simulink model "SAME5x_EXpicGUI_base"  (R2020b)
settings: Solver=FixedStepDiscrete  StartTime=0.0  StopTime=10.0  FixedStep=Ts  RelTol=1e-3  EnableMultiTasking=on
InitFcn:
  | % DC Voltage
  | VDC = 24;
  | 
  | 
  | % Intersective PMW
  | Vmax = VDC/2;
  | Imax = 4;
  | 
  | Ts = 1e-4;
  | 
  | 
  | 
  | 
  | 
  | 
  | % pole paires
  | p = 4;
  | 
  | % QEI
  | lines = 4*1000;
  | eleclines = lines/p;
  | inveleclines = 1/eleclines
  | gainQEIspeed = 2*pi/Ts/lines
  | 
  | 
  | 
  | % Electrical parameters
  | R=0.656; L=0.35e-3; Phif=0.0066;
  | % Mechanical parameters
  | F=1.e-05; J=1e-05; C0 = 0.01;%10;%1;
  | 
  | %% Current control synthesis
  | % Desired Carateristc Equation
  | %  1         2zeta
  | % ---- p^2+ ------- p + 1
  | % wn^2        wn
  | % Overshoot 5%, Trbf x wnbf = 3
  | tauE = L/R;
  | kE = 1/R;
  | trE = 3*tauE;
  | trED = trE;
  | zetaED = 1;
  | trwnE = 5;
  | wnED = trwnE/trED;
  | Pole_elec_desiree = roots([1/wnED^2 2*zetaED/wnED 1]);
  | 
  | % Retour d'etat de la dynamique electrique
  | Ae = [
  |         -R/L 0;
  |         -1 0;
  |     ];
  | 
  | Be = [
  |         1/L;
  |         0;
  |     ];
  | 
  | Kelec = place(Ae,Be,Pole_elec_desiree)
  | Kelec2 = [(2*zetaED*wnED*tauE-1)/kE -tauE*wnED^2/kE]
  | 
  | %% Asservissement de vitesse
  | % Desired polynomial equation
  | %  1         2 zeta
  | % ---- p^2+ ------- p + 1
  | % wn^2        wn
  | % overshoot 5%, Trbf x wnbf = 3
  | tauM = J/F;
  | kM = 3/2*p*Phif/F;
  | trM = 3*tauM;
  | zetaMD = 0.7;
  | trMD = trM/10;
  | trwnM = 3;
  | wnMD = trwnM/trMD;
  | Desired_mecha_pole = roots([1/wnMD^2 2*zetaMD/wnMD 1]);
  | % Mechanical state feedback
  | Am = [
  |         -1/tauM 0;
  |         -1 0;
  |     ];
  | 
  | Bm = [
  |         kM/tauM;
  |         0;
  |     ];
  | 
  | 
  | Kmeca = place(Am,Bm,Desired_mecha_pole)
  | 
  | Kmeca2 = [(2*zetaMD*wnMD*tauM-1)/kM -tauM*wnMD^2/kM]
  | 
  | 
  | 
  | 
  | 
  | 
  | % pole paires
  | pinit = 5;
  | % Electrical parameters
  | Rinit=0; Linit=0; Phifinit=0;
  | % Mechanical parameters
  | finit=1.0441e-04; Jinit=1.908e-04;
  | 
  | 
  | linesinit = 250;
  | 
  | %% Control law
  | %% Current control synthesis
  | 
  | Gainelecinit = 3;
  | Gainmecainit = .1;
undefined symbols (not defined in the file or in its folder): DiscIntNeverNeededParam, gcbh, MCHP_Digital_Input_Callback, MCHP_Digital_Output_Write_Callback, MCHP_Master_Callback, MCHP_OrderInOut, myParam, PA10, PA11, PA12, PA13, pad0, pad1, pad2, pad3, Pin
libraries: simulink x13, MCHP_Blockset x5
(part 1 of 3)
Description:
  | Motor Control Demo SAME5x
  | contacts : romain.delpoux@insa-lyon.fr, lubin.kerhuel@microchip.com
settings Model: Creator=r.delpoux  LastModifiedBy=promu
settings OptimizationCC: DefaultParameterBehavior=Inlined  DefaultUnderspecifiedDataType=single  EnhancedBackFolding=on  BooleansAsBitfields=on  PassReuseOutputArgsAs=Individual arguments  ZeroExternalMemoryAtStartup=off  ZeroInternalMemoryAtStartup=off  OptimizeBlockOrder=speed  DifferentSizesBufferReuse=on  EfficientTunableParamExpr=on
settings DebuggingCC: MultiTaskDSMMsg=none  MultiTaskCondExecSysMsg=warning  ParameterTunabilityLossMsg=error
settings HardwareCC: ProdBitPerPointer=32  ProdBitPerSizeT=32  ProdBitPerPtrDiffT=32  ProdLargestAtomicInteger=Long  ProdLargestAtomicFloat=Double  ProdWordSize=32  ProdHWDeviceType=ARM Compatible->ARM Cortex
settings ModelReferenceCC: ModelReferenceNumInstancesAllowed=Single
settings SFSimCC: MATLABDynamicMemAlloc=off
settings RTWCC: Description=Microchip Embedded Target Cortex M7 (real-time)  SystemTargetFile=MCHP_ARM7_stf.tlc  TemplateMakefile=MCHP_ARM7.tmf  Toolchain=xc32 - v2.50 for Mirochip SAMx7 device  BuildConfiguration=Specify
settings CodeAppCC: ForceParamTrailComments=on  IgnoreCustomStorageClasses=off  MaxIdLength=255  OperatorAnnotations=on  SimulinkDataObjDesc=on  SFDataObjDesc=on  InsertBlockDesc=on
settings STFCustomTargetCC: MultiwordLength=256  ConcurrentExecutionCompliant=off  IncludeMdlTerminateFcn=off  CombineOutputUpdateFcns=on  CombineSignalStateStructs=on  SuppressErrorStatus=on  ERTCustomFileBanners=on  SupportContinuousTime=off  RemoveResetFunc=on  MATLABClassNameForMDSCustomization=Simulink.SoftwareTarget.ERTCustomization  CPPClassGenCompliant=off  GRTInterface=off  UseToolchainInfoCompliant=on  SystemTargetFile=MCHP_ARM7_stf.tlc
settings ERTTargetCC: ParMdlRefBuildCompliant=off  CompOptLevelCompliant=off  ConcurrentExecutionCompliant=off  IncludeMdlTerminateFcn=off  CombineSignalStateStructs=on  SuppressErrorStatus=on  SupportNonInlinedSFcns=on  ModelStepFunctionPrototypeControlCompliant=off  CPPClassGenCompliant=off  ExtModeStaticAllocSize=2000  InlinedParameterPlacement=NonHierarchical  ERTSrcFileBannerTemplate=MCHP_dsPIC_code_template.cgt  ERTHdrFileBannerTemplate=MCHP_dsPIC_code_template.cgt  ERTDataSrcFileTemplate=MCHP_dsPIC_code_template.cgt  ERTDataHdrFileTemplate=MCHP_dsPIC_code_template.cgt  ERTCustomFileTemplate=MCHP_main.tlc  MaxLineWidth=110

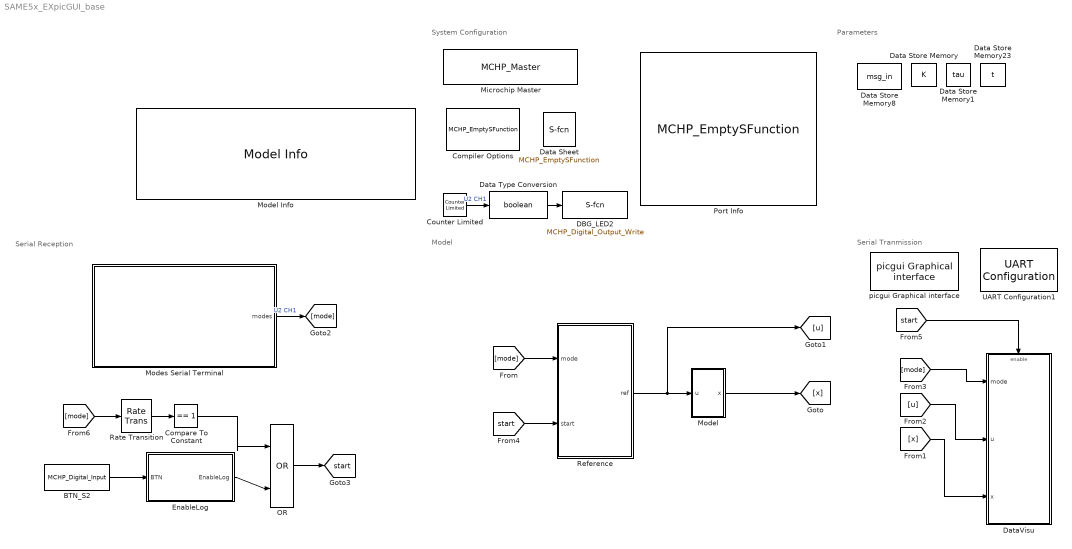
== system SAME5x_EXpicGUI_base ==
  note: Serial Reception
  note: System Configuration
  note: Serial Tranmission
  note: Model
  note: Parameters
  BTN_S2 : S-Function  FunctionName=MCHP_Digital_Input  Parameters=SampleTime,[],MCHP_Digital_Input_Callback(gcb,'S_OUTPUT'),MCHP_OrderInOut(gcbh)  SFunctionDeploymentMode=off  EnableBusSupport=off  mask(Input driver for Digital Input Pins){PORT=Dynamic Options, PORT_TXT=D   [ 0  1  8  9  10  11  12  20  21 ], PIN=9, PACK=off, SIMULTANEOUS=off, ORDERING=None, SampleTime=.1, MCHP_PORT={Digital In}{DIN}2:0:D9;, MCHP_MASTERLINK=SAME5x_EXpicGUI/Microchip Master}
      mask prompts: PORT_TXT "Port TXT"; PIN "PORT D Indexes within [ 0  1  8  9  10  11  12  20  21 ]"; PACK "set block output as one uint32"; SIMULTANEOUS "Exact simultaneous sample"; ORDERING "Block execution ordering"; SampleTime "Sample Time"
      mask help:
      | Selected pin(s) are configured as a digital input.
      |
      | When the block output is defined as one uint16, user should
      | take into account only bits corresponding to pins selected.
      mask init:
      | MCHP_Digital_Input_Callback(gcb,'INITIALISATION');
      settings: PreSaveFcn=MCHP_Fun.PreSaveFcn_DynamicOptions(gcbh);  OpenFcn=MCHP_Digital_Input_Callback(gcb,'OPEN');
      mask TypeOptions PORT: Dynamic Options
      mask Callback PORT: MCHP_Fun.BlockUpdate(gcbh);
      mask Callback PIN: MCHP_Fun.BlockUpdate(gcbh);
      mask Callback PACK: MCHP_Fun.BlockUpdate(gcbh);
      mask Callback SIMULTANEOUS: %MCHP_Fun.BlockUpdate(gcbh);
      mask TypeOptions ORDERING: None | Input | Output | Input & Output
      mask Display:
      | MCHP_DrawLogo;fprintf('Digital\nInput')
      | port_label('output',1,'D9');
  Compare To Constant : simulink/Logic and Bit Operations/Compare To Constant  relop===  const=1  OutDataTypeStr=boolean
  Compiler Options : S-Function  Priority=1  FunctionName=MCHP_EmptySFunction  SFunctionDeploymentMode=off  EnableBusSupport=off  mask{LATEST_CMPLR=on, COMP_LIST=Dynamic Options, COMP_LIST_TXT=xc32 - v2.50, DFP_LIST=Dynamic Options, DFP_LIST_TXT=v 3.2.56, CMSIS_DSP=Dynamic Options, CMSIS_DSP_TXT=Not used, USE_64BIT_DOUBLE=off, MCHP_MULTITHREAD_COMPILATION=on, UseCustom_LinkerScript=off, LinkerScript=, MCHP_MASTERLINK=SAME5x_EXpicGUI/Microchip Master, OPTIMIZATION_LEVEL=3, OPTIMIZATION_FLTO=off, OPTIMIZATION_REORDER=off, UNROLL_LOOPS=off, PROCEDURAL_ABSTRACTION=off, MPLAB_LINKLIB=default, MPLAB_LINKLIB1=fast floating-point math, CUSTOM_OPTIM=, CUSTOM_OPTIM_LD=, MCODE=is less than 32768 (faster), MCONST=in data memory, MDATA=Use only memory below address 8192 (faster), MSCALAR=Use only memory below address 8192 (faster), MLARGEARRAY=off, MAGGREGATE=off, HEAP_SIZE=1024, OMF=elf, DEBUG_INFO=on, ProduceHexOutput=on, AssemblyListing=off, NO_EDS_WARN=on, PRINT_STATISTICS=off}
      mask prompts: LATEST_CMPLR "Always use the latest compiler"; COMP_LIST "Select Compiler"; DFP_LIST "Device Family Pack (DFP)"; CMSIS_DSP "CMSIS DSP library"; USE_64BIT_DOUBLE "Use 64-bit double"; MCHP_MULTITHREAD_COMPILATION "Multithread Compilation (faster build)"; UseCustom_LinkerScript "Use a Custom Linker Script"; LinkerScript "Linker Script filename (full path if not in the model folder)"; OPTIMIZATION_LEVEL "Optimisation Level"; OPTIMIZATION_FLTO "Enable link-time optimizer"; OPTIMIZATION_REORDER "Allow reordering for ( fcts - variable - asm )"; UNROLL_LOOPS "Unroll Loops (improve speed)"; PROCEDURAL_ABSTRACTION "Procedural abstraction (reduce size)"; MPLAB_LINKLIB "Math Library"; MPLAB_LINKLIB1 "Math Library"; CUSTOM_OPTIM "Add custom argument for compiler"; CUSTOM_OPTIM_LD "Add custom argument for linker (coma separated)"; MCODE "Code size"; MCONST "Store Constant"; MDATA "Table data"; MSCALAR "Scalar data"; MLARGEARRAY "Allow array larger than 32K"; MAGGREGATE "Use aggregate data model"; HEAP_SIZE "Heap size"; OMF "Binary format :"; DEBUG_INFO "Generate debugging information"; ProduceHexOutput "Produce hex binary output file (.hex)"; AssemblyListing "Produce assembly listing file (.lst)"; NO_EDS_WARN "Disable eds-warning"; PRINT_STATISTICS "Print some statistics"
      mask init:
      | MCHP_CompilerOptimisation_Callback(gcbh, 'INITIALISATION');
      settings: PreSaveFcn=MCHP_Fun.PreSaveFcn_DynamicOptions(gcbh);  OpenFcn=MCHP_CompilerOptimisation_Callback(gcbh, 'OPEN');
      mask Callback LATEST_CMPLR: MCHP_Fun.BlockUpdate(gcbh);
      mask TypeOptions COMP_LIST: Dynamic Options
      mask Callback COMP_LIST: MCHP_Fun.BlockUpdate(gcbh);
      mask TypeOptions DFP_LIST: Dynamic Options
      mask TypeOptions CMSIS_DSP: Dynamic Options
      mask Callback UseCustom_LinkerScript: MCHP_CompilerOptimisation_Callback(gcbh, 'UseCustom_LinkerScript');
      mask TypeOptions OPTIMIZATION_LEVEL: 0 | 1 | 2 | s | 3
      mask TypeOptions MPLAB_LINKLIB: default | fast floating-point math | relaxed floating-point math
      mask TypeOptions MPLAB_LINKLIB1: default | fast floating-point math
      mask TypeOptions MCODE: is less than 32768 (faster) | is more than 32768
      mask TypeOptions MCONST: in code memory | in data memory
      mask TypeOptions MDATA: Use only memory below address 8192 (faster) | Can use all available memory
      mask TypeOptions MSCALAR: Use only memory below address 8192 (faster) | Can use all available memory
      mask TypeOptions OMF: elf | coff
      mask DialogControl ParameterTabVar0 Prompt: Compiler
      mask DialogControl ParameterTabVar01 Prompt: Optimization
      mask DialogControl ParameterTabVar012 Prompt: Memory
      mask DialogControl ParameterTabVar0123 Prompt: Output
      mask DialogControl ParameterTabVar01234 Prompt: Messages
      mask Display: MCHP_DrawLogo;disp(['Compiler-Version\n' COMP_LIST_TXT]);
  Counter Limited : simulink/Sources/Counter Limited  uplimit=1  tsamp=.1
  DBG_LED2 : S-Function  FunctionName=MCHP_Digital_Output_Write  Parameters=SampleTime,MCHP_Digital_Output_Write_Callback(gcb,'S_INPUT'),MCHP_Digital_Output_Write_Callback(gcb,'S_OUTPUT'),MCHP_OrderInOut(gcbh)  SFunctionDeploymentMode=off  EnableBusSupport=off  mask(Output driver for Digital Output Pins){PORT=Dynamic Options, PORT_TXT=B   [ 0 : 31 ], PIN=26, PACK=off, SIMULTANEOUS=off, ORDERING=None, SampleTime=-1, MCHP_PORT={Digital Out}{DOU}1:1:B26;, MCHP_MASTERLINK=SAME5x_EXpicGUI/Microchip Master}
      mask prompts: PORT_TXT "Port TXT"; PIN "PORT D Indexes within [ 0  1  8  9  10  11  12  20  21 ]"; PACK "set input as one uint16"; SIMULTANEOUS "Exact simultaneous update"; ORDERING "Block execution ordering"; SampleTime "Sample Time"
      mask help:
      | Selected pin(s) are configured as a digital output.
      |
      | When the block input is defined as one uint16, the value
      | is beeing used as is without masks.
      | This behaviour might affect others pins from the same port
      | provided they are configured as digital output as well.
      mask init:
      | MCHP_Digital_Output_Write_Callback(gcb,'INITIALISATION');
      settings: PreSaveFcn=MCHP_Fun.PreSaveFcn_DynamicOptions(gcbh);  OpenFcn=MCHP_Digital_Output_Write_Callback(gcb,'OPEN');
      mask TypeOptions PORT: Dynamic Options
      mask Callback PORT: MCHP_Fun.BlockUpdate(gcbh);
      mask Callback PIN: MCHP_Fun.BlockUpdate(gcbh);
      mask Callback PACK: MCHP_Fun.BlockUpdate(gcbh);
      mask Callback SIMULTANEOUS: %MCHP_Digital_Output_Write_Callback(gcb,'SIMULTANEOUS');
      mask TypeOptions ORDERING: None | Input | Output | Input & Output
      mask Display:
      | MCHP_DrawLogo;fprintf('Digital\nOutput\nWrite')
      | port_label('input',1,'B26');
  Data Sheet : S-Function  FunctionName=MCHP_EmptySFunction  SFunctionDeploymentMode=off  EnableBusSupport=off  mask{DOC_Type=datasheet, DOC_MCHP_Id=SAME54P20A_datasheet, DOC_FilePath=C:\Users\M91449\AppData\Local\Temp\60001507E.pdf, DOC_FileLastCheckTime=[2020              3             11             16              4         38.212], cpy_MCHP_Id=SAME54P20A, MCHP_MASTERLINK=SAME5x_EXpicGUI/Microchip Master}
      mask init:
      | MCHP_Doc_Callback(gcb,'INITIALISATION');
      settings: AttributesFormatString=%<cpy_MCHP_Id>  CopyFcn=MCHP_Doc_Callback(gcb,'COPY');  OpenFcn=MCHP_Doc_Callback(gcb,'OPEN');
      mask TypeOptions DOC_Type: datasheet | errata | www
      mask Display:
      | MCHP_DrawLogo;
      | plot([.8 0 0 1 1 .8 .8 1],[1 1 0 0 .8 1 .8 .8]);
      | text(.5,.6,'DOC','horizontalalignment','center');
      | text(.95,.05,'Pdf','verticalalignment','bottom','horizontalalignment','right');
  Data Store Memory : DataStoreMemory  DataStoreName=K  ReadBeforeWriteMsg=warning  WriteAfterWriteMsg=warning  WriteAfterReadMsg=warning  InitialValue=1  ShowAdditionalParam=off  OutDataTypeStr=single
  Data Store Memory1 : DataStoreMemory  DataStoreName=tau  ReadBeforeWriteMsg=warning  WriteAfterWriteMsg=warning  WriteAfterReadMsg=warning  InitialValue=0.1  ShowAdditionalParam=off  OutDataTypeStr=single
  Data Store Memory23 : DataStoreMemory  DataStoreName=t  ReadBeforeWriteMsg=warning  WriteAfterWriteMsg=warning  WriteAfterReadMsg=warning  InitialValue=1  ShowAdditionalParam=off  OutDataTypeStr=single
  Data Store Memory8 : DataStoreMemory  DataStoreName=msg_in  ReadBeforeWriteMsg=warning  WriteAfterWriteMsg=warning  WriteAfterReadMsg=warning  InitialValue=zeros(1,50)  ShowAdditionalParam=off
  Data Type Conversion : DataTypeConversion  OutDataTypeStr=boolean
  DataVisu : Subsystem
  EnableLog : Subsystem
  Microchip Master : S-Function  Priority=1  InitFcn=MCHP_Master_Callback(gcbh,'INIT');  FunctionName=MCHP_Master  SFunctionDeploymentMode=off  EnableBusSupport=off  mask{PICREF=SAME54P20A - TQFP128, PICREF_spd=, TIMESTEP_REF=Timer  ( 0.001s ), BUSYFLAG=Dynamic Options, BUSYFLAG_TXT=None, PWRTEN=Not used, BOREN=Disable, BODENV=2.7V, BORV=Not used, FPWRT=64ms, DSBOREN=Enable ZPBOR during Deep Sleep Mode, DSLPBOR=Not used, MCLRE=Enabled, SMCLR=MCLR pin generates a normal system Reset, PMDL1WAY=Allow only one reconfiguration, RSTPRI=Device will obtain reset instruction from Primary flash, TEMP=Not used, SOSCSRC=Not used, SOSCSEL=Not used, IOL1WAY=Allow only one reconfiguration, ALTVREF=Not used, DISUVREG=Not used, DSSWEN=Not used, LPCFG=Not used, RTCBAT=Not used, VBTBOR=Not used, WUTSEL=Not used, POWERSAVE=off, FNOSC=Primary Oscillator with PLL module (XT + PLL; HS + PLL; EC + PLL), FPR=ECIO w/ PLL 16x, FOSFPR=HS3 w/PLL 16x, FOS=Internal Fast RC, FRANGE=High Range, OSCILLATOR_SELECT=Crystal Oscillator in 8-48MHz on XIN/XOUT 0, OSCILLATOR_SELECT_spd=Crystal Oscillator in 8-48MHz on XIN/XOUT 0, QUARTZ=12e6, QUARTZ_spd=12e6, POSCGAIN=2x gain setting, POSCBOOST=Boost the kick start of the oscillator, SOSCGAIN=2x gain setting, SOSCBOOST=Boost the kick start of the oscillator, ACTIV_PLL=on, ACTIV_PLL_spd=on, MIPS_DESIRED=100e6, MIPS_DESIRED_spd=100e6, FPLLMUL=Not used, FPLLIDIV=8x Divider, POSCFREQ=Not used, POSCMD=Primary Oscillator Disabled, POSCMOD=Primary osc disabled, MIPS=100 * 1e6, ACLKCON=Optimized for PWM resolution & ADC conversion speed, ACLKCON_spd=Optimized for PWM resolution & ADC conversion speed, ACLKCON_Info=use FRC with auxilliary PLL, ADC Tad = 16.961(ns), PWM max resolution = 1.06(ns), FPLLODIV=32x Divider, PLLKEN=Clock switch to PLL source will wait until the PLL lock signal is valid, FCKSM=Both Clock switching and Fail-safe Clock Monitor are disabled, FCKSMEN=Sw Disabled; Mon Disabled, IESO=Start up with FRC; then switch, DSWDTPS=1:2^36, FWDTEN=Disable, FWDTWINSZ=Window size is 25%, FWPSA=1:512, FWPSA0=1:128, FWPSB=1:16, WDT=Disable, WDTPOST=1:32768, WDTPRE=1:128, WDTPS=1:1048576, WINDIS=Watchdog Timer in Non-Window mode, WWDTEN=Non-Window mode, DSWDTEN=Enable DSWDT during Deep Sleep Mode, DSWDTOSC=Select LPRC as DSWDT Reference clock, FPBDIV=Not used, FSOSCEN=Disable Secondary Oscillator, LPRCSEL=Not used, OSCIOFCN=Not used, OSCIOFNC=OSC2 is clock output, LVRCFG=Not used, PLL_96MHZ=Not used, PLL96MHZ=Not used, PLLDIV=Not used, WDTCLK=Not used, WDTCMX=Not used, WDTWIN=WDT Window is 25% of WDT period, XTCFG=24-32 MHz crystals, XTBST=Boost the kick-start, APL=Aux Flash Code protect is disabled, APLK=Aux Flash Write Protection or Code Protection is Enabled, AWRP=Auxiliary program memory is not write-protected, BSS=No Protection (other than BWRP), BWP=Not used, BWRP=Boot Segment may be written, CP=Protection Disabled, EBS=No Boot EEPROM, ESS=No Segment Data EEPROM, GCP=Disable, GSS=No Protection (other than GWRP), GSS0=Not used, GSSK=General Segment Write Protection or Code Protection is Enabled, GWRP=General Segment may be written, PWP=Not used, RBS=No Boot RAM, RSS=No Secure RAM, SSS=No Secure Segment, SWRP=Secure segment may be written, WPCFG=Not used, WPDIS=Not used, WPEND=Not used, WPFP=Not used, ICESEL=Communicate on PGEC1/PGED1, ICS=Communicate on PGEC1 and PGED1, JTAGEN=Disable, COE=Not used, RES=Not used, DEBUG=Debugger is disabled, BACKBUG=Not used, BKBUG=Not used, ALTI2C=I2C mapped to SDA1/SCL1 pins, ALTI2C1=I2C1 mapped to SDA1/SCL1 pins, ALTI2C2=I2C2 mapped to SDA2/SCL2 pins, ALTI2C3=I2C3 mapped to SDA3/SCL3 pins, ALTQIO=QEA1; QEB1; INDX1 are selected as inputs to QEI1, ALTSS1=SS1A is selected as the I/O pin for SPI1, CMPPOL0=Hysteresis is applied to falling edge, CMPPOL1=Hysteresis is applied to falling edge, FCANIO=Not used, FETHIO=Default Ethernet I/O, FMIIEN=MII Enabled, FSRSSEL=Not used, FUSBIDIO=Controlled by the USB Module, FVBUSONIO=Not used, HPOL=Active High, HYST0=45 mV Hysteresis, HYST1=45 mV Hysteresis, I2C1SEL=Not used, LPOL=Active High, PWMPIN=Control with PORT/TRIS regs, RTCOSC=Not used, UPLLEN=USB PLL Disabled, UPLLIDIV=Not used, ATMOD8=Not used, ALTPMP=Not used, I2C2SEL=Not used, ALTADREF=Not used, ALTCVREF=Not used, PWMLOCK=PWM registers may be written without key sequence, INT_PRIORITY_DMA=0, MCHP_TIMER_REQUEST={Time Step}{TS}0:2:3:1:[]:70000;, MCHP_TIMER_RESULT=[1 8748.999999999992724 ], MCHP_PORT=, MCHP_PLLRegisters=[5    243  16387     -1     -1], MCHPVAR=MCHP.id.name='SAME54P20A';MCHP.id.N=reshape([54 20 -1],1,3);MCHP.id.L=reshape({ 'SAME','P','A'},1,3);MCHP.id.Arch=5;MCHP.id.pinout=reshape({ 'TFBGA120','TQFP128'},1,2);MCHP.Rx=reshape([1 125 3 13 -1 -1 -1 -1 -1 -1 -1 -1 -1 -1 -1 -1 -1 -1 -1 -1 -1 2 126 4 16 -1 -1 -1 -1 -1 -1 -1 -1 -1 -1 -1 -1 -1 -1 -1 -1 -1 9 127 7 -1 -1 -1 -1 -1 -1 -1 -1 -1 -1 -1 -1 -1 -1 -1 -1 -1 -1 10 128 8 -1 -1 -1 -1 -1 -1 -1 -1 -1 -1 -1 -1 -1 -1 -1 -1 -1 -1 21 11 27 -1 -1 -1 -1 -1 -1 -1 -1 -1 -1 -1 -1 -1 -1 -1 -1 -1 -1 22 12 28 -1 -1 -1 -1 -1 -1 -1 -1 -1 -1 -1 -1 -1 -1 -1 -1 -1 -1 23 17 29 -1 -1 -1 -1 -1 -1 -1 -1 -1 -1 -1 -1 -1 -1 -1 -1 -1 -1 24 18 30 -1 -1 -1 -1 -1 -1 -1 -1 -1 -1 -1 -1 -1 -1 -1 -1 -1 -1 33 19 -1 47 -1 -1 -1 -1 -1 -1 -1 -1 -1 -1 -1 -1 -1 -1 -1 -1 -1 34 20 -1 48 -1 -1 -1 -1 -1 -1 -1 -1 -1 -1 -1 -1 -1 -1 -1 -1 -1 35 39 52 49 -1 -1 -1 -1 -1 -1 -1 -1 -1 -1 -1 -1 -1 -1 -1 -1 -1 36 40 55 50 -1 -1 -1 -1 -1 -1 -1 -1 -1 -1 -1 -1 -1 -1 -1 -1 -1 60 41 56 51 -1 -1 -1 -1 -1 -1 -1 -1 -1 -1 -1 -1 -1 -1 -1 -1 -1 61 42 57 -1 -1 -1 -1 -1 -1 -1 -1 -1 -1 -1 -1 -1 -1 -1 -1 -1 -1 62 43 58 -1 -1 -1 -1 -1 -1 -1 -1 -1 -1 -1 -1 -1 -1 -1 -1 -1 -1 63 44 59 -1 -1 -1 -1 -1 -1 -1 -1 -1 -1 -1 -1 -1 -1 -1 -1 -1 -1 66 82 70 -1 -1 -1 -1 -1 -1 -1 -1 -1 -1 -1 -1 -1 -1 -1 -1 -1 -1 67 83 71 -1 -1 -1 -1 -1 -1 -1 -1 -1 -1 -1 -1 -1 -1 -1 -1 -1 -1 68 84 72 -1 -1 -1 -1 -1 -1 -1 -1 -1 -1 -1 -1 -1 -1 -1 -1 -1 -1 69 85 73 -1 -1 -1 -1 -1 -1 -1 -1 -1 -1 -1 -1 -1 -1 -1 -1 -1 -1 88 86 74 80 -1 -1 -1 -1 -1 -1 -1 -1 -1 -1 -1 -1 -1 -1 -1 -1 -1 89 87 75 81 -1 -1 -1 -1 -1 -1 -1 -1 -1 -1 -1 -1 -1 -1 -1 -1 -1 92 98 76 -1 -1 -1 -1 -1 -1 -1 -1 -1 -1 -1 -1 -1 -1 -1 -1 -1 -1 93 99 77 -1 -1 -1 -1 -1 -1 -1 -1 -1 -1 -1 -1 -1 -1 -1 -1 -1 -1 94 100 108 -1 -1 -1 -1 -1 -1 -1 -1 -1 -1 -1 -1 -1 -1 -1 -1 -1 -1 95 101 109 -1 -1 -1 -1 -1 -1 -1 -1 -1 -1 -1 -1 -1 -1 -1 -1 -1 -1 -1 102 110 -1 -1 -1 -1 -1 -1 -1 -1 -1 -1 -1 -1 -1 -1 -1 -1 -1 -1 113 103 111 -1 -1 -1 -1 -1 -1 -1 -1 -1 -1 -1 -1 -1 -1 -1 -1 -1 -1 -1 104 112 -1 -1 -1 -1 -1 -1 -1 -1 -1 -1 -1 -1 -1 -1 -1 -1 -1 -1 -1 105 -1 -1 -1 -1 -1 -1 -1 -1 -1 -1 -1 -1 -1 -1 -1 -1 -1 -1 -1 119 121 123 -1 -1 -1 -1 -1 -1 -1 -1 -1 -1 -1 -1 -1 -1 -1 -1 -1 -1 120 122 124 -1 -1 -1 -1 -1 -1 -1 -1 -1 -1 -1 -1 -1 -1 -1 -1 -1 -1],21,32);MCHP.memory.FLASH.size=1048576;MCHP.memory.SW0.size=16;MCHP.memory.TEMP_LOG.size=512;MCHP.memory.USER_PAGE.size=512;MCHP.memory.CMCC.size=16777216;MCHP.memory.CMCC_DATARAM.size=4096;MCHP.memory.CMCC_TAGRAM.size=1024;MCHP.memory.CMCC_VALIDRAM.size=64;MCHP.memory.QSPI.size=16777216;MCHP.memory.HSRAM.size=262144;MCHP.memory.HSRAM_ETB.size=32768;MCHP.memory.HSRAM_RET1.size=32768;MCHP.memory.HPB0.size=17408;MCHP.memory.HPB1.size=139264;MCHP.memory.HPB2.size=15360;MCHP.memory.HPB3.size=12288;MCHP.memory.SEEPROM.size=131072;MCHP.memory.SDHC0.size=3072;MCHP.memory.SDHC1.size=3072;MCHP.memory.BKUPRAM.size=8192;MCHP.memory.PPB.size=1048576;MCHP.memory.SCS.size=4096;MCHP.memory.PERIPHERALS.size=MCHP_Fun.Hex2num('41C0000000000000');MCHP.module.PM.PID=0;MCHP.module.PM.vector='PM';MCHP.module.MCLK.PID=1;MCHP.module.MCLK.vector='MCLK';MCHP.module.OSCCTRL(1).PID=2;MCHP.module.OSCCTRL(1).vector='OSCCTRL_XOSC0';MCHP.module.OSCCTRL(2).PID=3;MCHP.module.OSCCTRL(2).vector='OSCCTRL_XOSC1';MCHP.module.OSCCTRL(3).PID=4;MCHP.module.OSCCTRL(3).vector='OSCCTRL_DFLL';MCHP.module.OSCCTRL(4).PID=5;MCHP.module.OSCCTRL(4).vector='OSCCTRL_DPLL0';MCHP.module.OSCCTRL(5).PID=6;MCHP.module.OSCCTRL(5).vector='OSCCTRL_DPLL1';MCHP.module.OSC32KCTRL.PID=7;MCHP.module.OSC32KCTRL.vector='OSC32KCTRL';MCHP.module.SUPC(1).PID=8;MCHP.module.SUPC(1).vector='SUPC_OTHER';MCHP.module.SUPC(2).PID=9;MCHP.module.SUPC(2).vector='SUPC_BODDET';MCHP.module.WDT.PID=10;MCHP.module.WDT.vector='WDT';MCHP.module.RTC.PID=11;MCHP.module.RTC.vector='RTC';MCHP.module.EIC(1).PID=12;MCHP.module.EIC(1).vector='EIC_EXTINT_0';MCHP.module.EIC(1).pin.EXTINT0.txt=reshape({ 'PA00','PA16','PB00','PB16','PC00','PC16','PD00'},1,7);MCHP.module.EIC(1).pin.EXTINT0.Rx_idx=reshape([0 16 32 48 64 80 96],1,7);MCHP.module.EIC(1).pin.EXTINT0.ABCD=reshape([0 0 0 0 0 0 0],1,7);MCHP.module.EIC(1).pin.EXTINT1.txt=reshape({ 'PA01','PA17','PB01','PB17','PC01','PC17','PD01'},1,7);MCHP.module.EIC(1).pin.EXTINT1.Rx_idx=reshape([1 17 33 49 65 81 97],1,7);MCHP.module.EIC(1).pin.EXTINT1.ABCD=reshape([0 0 0 0 0 0 0],1,7);MCHP.module.EIC(1).pin.EXTINT2.txt=reshape({ 'PA02','PA18','PB02','PB18','PC02','PC18'},1,6);MCHP.module.EIC(1).pin.EXTINT2.Rx_idx=reshape([2 18 34 50 66 82],1,6);MCHP.module.EIC(1).pin.EXTINT2.ABCD=reshape([0 0 0 0 0 0],1,6);MCHP.module.EIC(1).pin.EXTINT3.txt=reshape({ 'PA03','PA19','PB03','PB19','PC03','PC19','PD08'},1,7);MCHP.module.EIC(1).pin.EXTINT3.Rx_idx=reshape([3 19 35 51 67 83 104],1,7);MCHP.module.EIC(1).pin.EXTINT3.ABCD=reshape([0 0 0 0 0 0 0],1,7);MCHP.module.EIC(1).pin.EXTINT4.txt=reshape({ 'PA04','PA20','PB04','PB20','PC04','PC20','PD09'},1,7);MCHP.module.EIC(1).pin.EXTINT4.Rx_idx=reshape([4 20 36 52 68 84 105],1,7);MCHP.module.EIC(1).pin.EXTINT4.ABCD=reshape([0 0 0 0 0 0 0],1,7);MCHP.module.EIC(1).pin.EXTINT5.txt=reshape({ 'PA05','PA21','PB05','PB21','PC05','PC21','PD10'},1,7);MCHP.module.EIC(1).pin.EXTINT5.Rx_idx=reshape([5 21 37 53 69 85 106],1,7);MCHP.module.EIC(1).pin.EXTINT5.ABCD=reshape([0 0 0 0 0 0 0],1,7);MCHP.module.EIC(1).pin.EXTINT6.txt=reshape({ 'PA06','PA22','PB06','PB22','PC06','PC22','PD11'},1,7);MCHP.module.EIC(1).pin.EXTINT6.Rx_idx=reshape([6 22 38 54 70 86 107],1,7);MCHP.module.EIC(1).pin.EXTINT6.ABCD=reshape([0 0 0 0 0 0 0],1,7);MCHP.module.EIC(1).pin.EXTINT7.txt=reshape({ 'PA07','PA23','PB07','PB23','PC23','PD12'},1,6);MCHP.module.EIC(1).pin.EXTINT7.Rx_idx=reshape([7 23 39 55 87 108],1,6);MCHP.module.EIC(1).pin.EXTINT7.ABCD=reshape([0 0 0 0 0 0],1,6);MCHP.module.EIC(1).pin.EXTINT8.txt=reshape({ 'PA24','PB08','PB24','PC24'},1,4);MCHP.module.EIC(1).pin.EXTINT8.Rx_idx=reshape([24 40 56 88],1,4);MCHP.module.EIC(1).pin.EXTINT8.ABCD=reshape([0 0 0 0],1,4);MCHP.module.EIC(1).pin.EXTINT9.txt=reshape({ 'PA09','PA25','PB09','PB25','PC07','PC25'},1,6);MCHP.module.EIC(1).pin.EXTINT9.Rx_idx=reshape([9 25 41 57 71 89],1,6);MCHP.module.EIC(1).pin.EXTINT9.ABCD=reshape([0 0 0 0 0 0],1,6);MCHP.module.EIC(1).pin.EXTINT10.txt=reshape({ 'PA10','PB10','PC10','PC26','PD20'},1,5);MCHP.module.EIC(1).pin.EXTINT10.Rx_idx=reshape([10 42 74 90 116],1,5);MCHP.module.EIC(1).pin.EXTINT10.ABCD=reshape([0 0 0 0 0],1,5);MCHP.module.EIC(1).pin.EXTINT11.txt=reshape({ 'PA11','PA27','PB11','PC11','PC27','PD21'},1,6);MCHP.module.EIC(1).pin.EXTINT11.Rx_idx=reshape([11 27 43 75 91 117],1,6);MCHP.module.EIC(1).pin.EXTINT11.ABCD=reshape([0 0 0 0 0 0],1,6);MCHP.module.EIC(1).pin.EXTINT12.txt=reshape({ 'PA12','PB12','PB26','PC12','PC28'},1,5);MCHP.module.EIC(1).pin.EXTINT12.Rx_idx=reshape([12 44 58 76 92],1,5);MCHP.module.EIC(1).pin.EXTINT12.ABCD=reshape([0 0 0 0 0],1,5);MCHP.module.EIC(1).pin.EXTINT13.txt=reshape({ 'PA13','PB13','PB27','PC13'},1,4);MCHP.module.EIC(1).pin.EXTINT13.Rx_idx=reshape([13 45 59 77],1,4);MCHP.module.EIC(1).pin.EXTINT13.ABCD=reshape([0 0 0 0],1,4);MCHP.module.EIC(1).pin.EXTINT14.txt=reshape({ 'PA30','PB14','PB28','PB30','PC14','PC30','PA14'},1,7);MCHP.module.EIC(1).pin.EXTINT14.Rx_idx=reshape([30 46 60 62 78 94 14],1,7);MCHP.module.EIC(1).pin.EXTINT14.ABCD=reshape([0 0 0 0 0 0 0],1,7);MCHP.module.EIC(1).pin.EXTINT15.txt=reshape({ 'PA15','PA31','PB15','PB29','PB31','PC15','PC31'},1,7);MCHP.module.EIC(1).pin.EXTINT15.Rx_idx=reshape([15 31 47 61 63 79 95],1,7);MCHP.module.EIC(1).pin.EXTINT15.ABCD=reshape([0 0 0 0 0 0 0],1,7);MCHP.module.EIC(1).pin.NMI.txt={ 'PA08'};MCHP.module.EIC(1).pin.NMI.Rx_idx=8;MCHP.module.EIC(1).pin.NMI.ABCD=0;MCHP.module.EIC(2).PID=13;MCHP.module.EIC(2).vector='EIC_EXTINT_1';MCHP.module.EIC(2).pin=reshape(MCHP_Fun.Hex2num('[]'),0,0);MCHP.module.EIC(3).PID=14;MCHP.module.EIC(3).vector='EIC_EXTINT_2';MCHP.module.EIC(3).pin=reshape(MCHP_Fun.Hex2num('[]'),0,0);MCHP.module.EIC(4).PID=15;MCHP.module.EIC(4).vector='EIC_EXTINT_3';MCHP.module.EIC(4).pin=reshape(MCHP_Fun.Hex2num('[]'),0,0);MCHP.module.EIC(5).PID=16;MCHP.module.EIC(5).vector='EIC_EXTINT_4';MCHP.module.EIC(5).pin=reshape(MCHP_Fun.Hex2num('[]'),0,0);MCHP.module.EIC(6).PID=17;MCHP.module.EIC(6).vector='EIC_EXTINT_5';MCHP.module.EIC(6).pin=reshape(MCHP_Fun.Hex2num('[]'),0,0);MCHP.module.EIC(7).PID=18;MCHP.module.EIC(7).vector='EIC_EXTINT_6';MCHP.module.EIC(7).pin=reshape(MCHP_Fun.Hex2num('[]'),0,0);MCHP.module.EIC(8).PID=19;MCHP.module.EIC(8).vector='EIC_EXTINT_7';MCHP.module.EIC(8).pin=reshape(MCHP_Fun.Hex2num('[]'),0,0);MCHP.module.EIC(9).PID=20;MCHP.module.EIC(9).vector='EIC_EXTINT_8';MCHP.module.EIC(9).pin=reshape(MCHP_Fun.Hex2num('[]'),0,0);MCHP.module.EIC(10).PID=21;MCHP.module.EIC(10).vector='EIC_EXTINT_9';MCHP.module.EIC(10).pin=reshape(MCHP_Fun.Hex2num('[]'),0,0);MCHP.module.EIC(11).PID=22;MCHP.module.EIC(11).vector='EIC_EXTINT_10';MCHP.module.EIC(11).pin=reshape(MCHP_Fun.Hex2num('[]'),0,0);MCHP.module.EIC(12).PID=23;MCHP.module.EIC(12).vector='EIC_EXTINT_11';MCHP.module.EIC(12).pin=reshape(MCHP_Fun.Hex2num('[]'),0,0);MCHP.module.EIC(13).PID=24;MCHP.module.EIC(13).vector='EIC_EXTINT_12';MCHP.module.EIC(13).pin=reshape(MCHP_Fun.Hex2num('[]'),0,0);MCHP.module.EIC(14).PID=25;MCHP.module.EIC(14).vector='EIC_EXTINT_13';MCHP.module.EIC(14).pin=reshape(MCHP_Fun.Hex2num('[]'),0,0);MCHP.module.EIC(15).PID=26;MCHP.module.EIC(15).vector='EIC_EXTINT_14';MCHP.module.EIC(15).pin=reshape(MCHP_Fun.Hex2num('[]'),0,0);MCHP.module.EIC(16).PID=27;MCHP.module.EIC(16).vector='EIC_EXTINT_15';MCHP.module.EIC(16).pin=reshape(MCHP_Fun.Hex2num('[]'),0,0);MCHP.module.FREQM.PID=28;MCHP.module.FREQM.vector='FREQM';MCHP.module.NVMCTRL(1).PID=29;MCHP.module.NVMCTRL(1).vector='NVMCTRL_0';MCHP.module.NVMCTRL(2).PID=30;MCHP.module.NVMCTRL(2).vector='NVMCTRL_1';MCHP.module.DMAC(1).PID=31;MCHP.module.DMAC(1).vector='DMAC_0';MCHP.module.DMAC(2).PID=32;MCHP.module.DMAC(2).vector='DMAC_1';MCHP.module.DMAC(3).PID=33;MCHP.module.DMAC(3).vector='DMAC_2';MCHP.module.DMAC(4).PID=34;MCHP.module.DMAC(4).vector='DMAC_3';MCHP.module.DMAC(5).PID=35;MCHP.module.DMAC(5).vector='DMAC_OTHER';MCHP.module.EVSYS(1).PID=36;MCHP.module.EVSYS(1).vector='EVSYS_0';MCHP.module.EVSYS(2).PID=37;MCHP.module.EVSYS(2).vector='EVSYS_1';MCHP.module.EVSYS(3).PID=38;MCHP.module.EVSYS(3).vector='EVSYS_2';MCHP.module.EVSYS(4).PID=39;MCHP.module.EVSYS(4).vector='EVSYS_3';MCHP.module.EVSYS(5).PID=40;MCHP.module.EVSYS(5).vector='EVSYS_OTHER';MCHP.module.PAC.PID=41;MCHP.module.PAC.vector='PAC';MCHP.module.RAMECC.PID=45;MCHP.module.RAMECC.vector='RAMECC';MCHP.module.SERCOM0(1).PID=46;MCHP.module.SERCOM0(1).vector='SERCOM0_0';MCHP.module.SERCOM0(1).pin.PAD0.txt=reshape({ 'PA04','PC17','PA08','PB24'},1,4);MCHP.module.SERCOM0(1).pin.PAD0.Rx_idx=reshape([4 81 8 56],1,4);MCHP.module.SERCOM0(1).pin.PAD0.ABCD=reshape([3 3 2 2],1,4);MCHP.module.SERCOM0(1).pin.PAD1.txt=reshape({ 'PA05','PC16','PA09','PB25'},1,4);MCHP.module.SERCOM0(1).pin.PAD1.Rx_idx=reshape([5 80 9 57],1,4);MCHP.module.SERCOM0(1).pin.PAD1.ABCD=reshape([3 3 2 2],1,4);MCHP.module.SERCOM0(1).pin.PAD2.txt=reshape({ 'PA06','PC18','PA10','PC24'},1,4);MCHP.module.SERCOM0(1).pin.PAD2.Rx_idx=reshape([6 82 10 88],1,4);MCHP.module.SERCOM0(1).pin.PAD2.ABCD=reshape([3 3 2 2],1,4);MCHP.module.SERCOM0(1).pin.PAD3.txt=reshape({ 'PA07','PC19','PA11','PC25'},1,4);MCHP.module.SERCOM0(1).pin.PAD3.Rx_idx=reshape([7 83 11 89],1,4);MCHP.module.SERCOM0(1).pin.PAD3.ABCD=reshape([3 3 2 2],1,4);MCHP.module.SERCOM0(2).PID=47;MCHP.module.SERCOM0(2).vector='SERCOM0_1';MCHP.module.SERCOM0(2).pin=reshape(MCHP_Fun.Hex2num('[]'),0,0);MCHP.module.SERCOM0(3).PID=48;MCHP.module.SERCOM0(3).vector='SERCOM0_2';MCHP.module.SERCOM0(3).pin=reshape(MCHP_Fun.Hex2num('[]'),0,0);MCHP.module.SERCOM0(4).PID=49;MCHP.module.SERCOM0(4).vector='SERCOM0_OTHER';MCHP.module.SERCOM0(4).pin=reshape(MCHP_Fun.Hex2num('[]'),0,0);MCHP.module.SERCOM1(1).PID=50;MCHP.module.SERCOM1(1).vector='SERCOM1_0';MCHP.module.SERCOM1(1).pin.PAD0.txt=reshape({ 'PA00','PA16','PC22','PC27'},1,4);MCHP.module.SERCOM1(1).pin.PAD0.Rx_idx=reshape([0 16 86 91],1,4);MCHP.module.SERCOM1(1).pin.PAD0.ABCD=reshape([3 2 2 2],1,4);MCHP.module.SERCOM1(1).pin.PAD1.txt=reshape({ 'PA01','PA17','PC23','PC28'},1,4);MCHP.module.SERCOM1(1).pin.PAD1.Rx_idx=reshape([1 17 87 92],1,4);MCHP.module.SERCOM1(1).pin.PAD1.ABCD=reshape([3 2 2 2],1,4);MCHP.module.SERCOM1(1).pin.PAD2.txt=reshape({ 'PA30','PA18','PB22','PD20'},1,4);MCHP.module.SERCOM1(1).pin.PAD2.Rx_idx=reshape([30 18 54 116],1,4);MCHP.module.SERCOM1(1).pin.PAD2.ABCD=reshape([3 2 2 2],1,4);MCHP.module.SERCOM1(1).pin.PAD3.txt=reshape({ 'PA31','PA19','PB23','PD21'},1,4);MCHP.module.SERCOM1(1).pin.PAD3.Rx_idx=reshape([31 19 55 117],1,4);MCHP.module.SERCOM1(1).pin.PAD3.ABCD=reshape([3 2 2 2],1,4);MCHP.module.SERCOM1(2).PID=51;MCHP.module.SERCOM1(2).vector='SERCOM1_1';MCHP.module.SERCOM1(2).pin=reshape(MCHP_Fun.Hex2num('[]'),0,0);MCHP.module.SERCOM1(3).PID=52;MCHP.module.SERCOM1(3).vector='SERCOM1_2';MCHP.module.SERCOM1(3).pin=reshape(MCHP_Fun.Hex2num('[]'),0,0);MCHP.module.SERCOM1(4).PID=53;MCHP.module.SERCOM1(4).vector='SERCOM1_OTHER';MCHP.module.SERCOM1(4).pin=reshape(MCHP_Fun.Hex2num('[]'),0,0);MCHP.module.SERCOM2(1).PID=54;MCHP.module.SERCOM2(1).vector='SERCOM2_0';MCHP.module.SERCOM2(1).pin.PAD0.txt=reshape({ 'PA09','PB25','PA12','PB26'},1,4);MCHP.module.SERCOM2(1).pin.PAD0.Rx_idx=reshape([9 57 12 58],1,4);MCHP.module.SERCOM2(1).pin.PAD0.ABCD=reshape([3 3 2 2],1,4);MCHP.module.SERCOM2(1).pin.PAD1.txt=reshape({ 'PA08','PB24','PA13','PB27'},1,4);MCHP.module.SERCOM2(1).pin.PAD1.Rx_idx=reshape([8 56 13 59],1,4);MCHP.module.SERCOM2(1).pin.PAD1.ABCD=reshape([3 3 2 2],1,4);MCHP.module.SERCOM2(1).pin.PAD2.txt=reshape({ 'PA10','PC24','PB28','PA14'},1,4);MCHP.module.SERCOM2(1).pin.PAD2.Rx_idx=reshape([10 88 60 14],1,4);MCHP.module.SERCOM2(1).pin.PAD2.ABCD=reshape([3 3 2 2],1,4);MCHP.module.SERCOM2(1).pin.PAD3.txt=reshape({ 'PA11','PC25','PB29','PA15'},1,4);MCHP.module.SERCOM2(1).pin.PAD3.Rx_idx=reshape([11 89 61 15],1,4);MCHP.module.SERCOM2(1).pin.PAD3.ABCD=reshape([3 3 2 2],1,4);MCHP.module.SERCOM2(2).PID=55;MCHP.module.SERCOM2(2).vector='SERCOM2_1';MCHP.module.SERCOM2(2).pin=reshape(MCHP_Fun.Hex2num('[]'),0,0);MCHP.module.SERCOM2(3).PID=56;MCHP.module.SERCOM2(3).vector='SERCOM2_2';MCHP.module.SERCOM2(3).pin=reshape(MCHP_Fun.Hex2num('[]'),0,0);MCHP.module.SERCOM2(4).PID=57;MCHP.module.SERCOM2(4).vector='SERCOM2_OTHER';MCHP.module.SERCOM2(4).pin=reshape(MCHP_Fun.Hex2num('[]'),0,0);MCHP.module.SERCOM3(1).PID=58;MCHP.module.SERCOM3(1).vector='SERCOM3_0';MCHP.module.SERCOM3(1).pin.PAD0.txt=reshape({ 'PA17','PC23','PA22','PB20'},1,4);MCHP.module.SERCOM3(1).pin.PAD0.Rx_idx=reshape([17 87 22 52],1,4);MCHP.module.SERCOM3(1).pin.PAD0.ABCD=reshape([3 3 2 2],1,4);MCHP.module.SERCOM3(1).pin.PAD1.txt=reshape({ 'PA16','PC22','PA23','PB21'},1,4);MCHP.module.SERCOM3(1).pin.PAD1.Rx_idx=reshape([16 86 23 53],1,4);MCHP.module.SERCOM3(1).pin.PAD1.ABCD=reshape([3 3 2 2],1,4);MCHP.module.SERCOM3(1).pin.PAD2.txt=reshape({ 'PA18','PA20','PD20','PA24'},1,4);MCHP.module.SERCOM3(1).pin.PAD2.Rx_idx=reshape([18 20 116 24],1,4);MCHP.module.SERCOM3(1).pin.PAD2.ABCD=reshape([3 3 3 2],1,4);MCHP.module.SERCOM3(1).pin.PAD3.txt=reshape({ 'PA19','PA21','PD21','PA25'},1,4);MCHP.module.SERCOM3(1).pin.PAD3.Rx_idx=reshape([19 21 117 25],1,4);MCHP.module.SERCOM3(1).pin.PAD3.ABCD=reshape([3 3 3 2],1,4);MCHP.module.SERCOM3(2).PID=59;MCHP.module.SERCOM3(2).vector='SERCOM3_1';MCHP.module.SERCOM3(2).pin=reshape(MCHP_Fun.Hex2num('[]'),0,0);MCHP.module.SERCOM3(3).PID=60;MCHP.module.SERCOM3(3).vector='SERCOM3_2';MCHP.module.SERCOM3(3).pin=reshape(MCHP_Fun.Hex2num('[]'),0,0);MCHP.module.SERCOM3(4).PID=61;MCHP.module.SERCOM3(4).vector='SERCOM3_OTHER';MCHP.module.SERCOM3(4).pin=reshape(MCHP_Fun.Hex2num('[]'),0,0);MCHP.module.SERCOM4(1).PID=62;MCHP.module.SERCOM4(1).vector='SERCOM4_0';MCHP.module.SERCOM4(1).pin.PAD0.txt=reshape({ 'PA13','PB08','PB27','PB12'},1,4);MCHP.module.SERCOM4(1).pin.PAD0.Rx_idx=reshape([13 40 59 44],1,4);MCHP.module.SERCOM4(1).pin.PAD0.ABCD=reshape([3 3 3 2],1,4);MCHP.module.SERCOM4(1).pin.PAD1.txt=reshape({ 'PA12','PB09','PB26','PB13'},1,4);MCHP.module.SERCOM4(1).pin.PAD1.Rx_idx=reshape([12 41 58 45],1,4);MCHP.module.SERCOM4(1).pin.PAD1.ABCD=reshape([3 3 3 2],1,4);MCHP.module.SERCOM4(1).pin.PAD2.txt=reshape({ 'PA14','PB10','PB28','PB14'},1,4);MCHP.module.SERCOM4(1).pin.PAD2.Rx_idx=reshape([14 42 60 46],1,4);MCHP.module.SERCOM4(1).pin.PAD2.ABCD=reshape([3 3 3 2],1,4);MCHP.module.SERCOM4(1).pin.PAD3.txt=reshape({ 'PB11','PB29','PA15','PB15'},1,4);MCHP.module.SERCOM4(1).pin.PAD3.Rx_idx=reshape([43 61 15 47],1,4);MCHP.module.SERCOM4(1).pin.PAD3.ABCD=reshape([3 3 3 2],1,4);MCHP.module.SERCOM4(2).PID=63;MCHP.module.SERCOM4(2).vector='SERCOM4_1';MCHP.module.SERCOM4(2).pin=reshape(MCHP_Fun.Hex2num('[]'),0,0);MCHP.module.SERCOM4(3).PID=64;MCHP.module.SERCOM4(3).vector='SERCOM4_2';MCHP.module.SERCOM4(3).pin=reshape(MCHP_Fun.Hex2num('[]'),0,0);MCHP.module.SERCOM4(4).PID=65;MCHP.module.SERCOM4(4).vector='SERCOM4_OTHER';MCHP.module.SERCOM4(4).pin=reshape(MCHP_Fun.Hex2num('[]'),0,0);MCHP.module.SERCOM5(1).PID=66;MCHP.module.SERCOM5(1).vector='SERCOM5_0';MCHP.module.SERCOM5(1).pin.PAD0.txt=reshape({ 'PA23','PB02','PB31','PB16'},1,4);MCHP.module.SERCOM5(1).pin.PAD0.Rx_idx=reshape([23 34 63 48],1,4);MCHP.module.SERCOM5(1).pin.PAD0.ABCD=reshape([3 3 3 2],1,4);MCHP.module.SERCOM5(1).pin.PAD1.txt=reshape({ 'PA22','PB03','PB30','PB17'},1,4);MCHP.module.SERCOM5(1).pin.PAD1.Rx_idx=reshape([22 35 62 49],1,4);MCHP.module.SERCOM5(1).pin.PAD1.ABCD=reshape([3 3 3 2],1,4);MCHP.module.SERCOM5(1).pin.PAD2.txt=reshape({ 'PA24','PB00','PB22','PA20','PB18'},1,5);MCHP.module.SERCOM5(1).pin.PAD2.Rx_idx=reshape([24 32 54 20 50],1,5);MCHP.module.SERCOM5(1).pin.PAD2.ABCD=reshape([3 3 3 2 2],1,5);MCHP.module.SERCOM5(1).pin.PAD3.txt=reshape({ 'PA25','PB01','PB23','PA21','PB19'},1,5);MCHP.module.SERCOM5(1).pin.PAD3.Rx_idx=reshape([25 33 55 21 51],1,5);MCHP.module.SERCOM5(1).pin.PAD3.ABCD=reshape([3 3 3 2 2],1,5);MCHP.module.SERCOM5(2).PID=67;MCHP.module.SERCOM5(2).vector='SERCOM5_1';MCHP.module.SERCOM5(2).pin=reshape(MCHP_Fun.Hex2num('[]'),0,0);MCHP.module.SERCOM5(3).PID=68;MCHP.module.SERCOM5(3).vector='SERCOM5_2';MCHP.module.SERCOM5(3).pin=reshape(MCHP_Fun.Hex2num('[]'),0,0);MCHP.module.SERCOM5(4).PID=69;MCHP.module.SERCOM5(4).vector='SERCOM5_OTHER';MCHP.module.SERCOM5(4).pin=reshape(MCHP_Fun.Hex2num('[]'),0,0);MCHP.module.SERCOM6(1).PID=70;MCHP.module.SERCOM6(1).vector='SERCOM6_0';MCHP.module.SERCOM6(1).pin.PAD0.txt=reshape({ 'PD09','PC13','PC04','PC16'},1,4);MCHP.module.SERCOM6(1).pin.PAD0.Rx_idx=reshape([105 77 68 80],1,4);MCHP.module.SERCOM6(1).pin.PAD0.ABCD=reshape([3 3 2 2],1,4);MCHP.module.SERCOM6(1).pin.PAD1.txt=reshape({ 'PD08','PC12','PC05','PC17'},1,4);MCHP.module.SERCOM6(1).pin.PAD1.Rx_idx=reshape([104 76 69 81],1,4);MCHP.module.SERCOM6(1).pin.PAD1.ABCD=reshape([3 3 2 2],1,4);MCHP.module.SERCOM6(1).pin.PAD2.txt=reshape({ 'PC14','PD10','PC06','PC10','PC18'},1,5);MCHP.module.SERCOM6(1).pin.PAD2.Rx_idx=reshape([78 106 70 74 82],1,5);MCHP.module.SERCOM6(1).pin.PAD2.ABCD=reshape([3 3 2 2 2],1,5);MCHP.module.SERCOM6(1).pin.PAD3.txt=reshape({ 'PC15','PD11','PC07','PC11','PC19'},1,5);MCHP.module.SERCOM6(1).pin.PAD3.Rx_idx=reshape([79 107 71 75 83],1,5);MCHP.module.SERCOM6(1).pin.PAD3.ABCD=reshape([3 3 2 2 2],1,5);MCHP.module.SERCOM6(2).PID=71;MCHP.module.SERCOM6(2).vector='SERCOM6_1';MCHP.module.SERCOM6(2).pin=reshape(MCHP_Fun.Hex2num('[]'),0,0);MCHP.module.SERCOM6(3).PID=72;MCHP.module.SERCOM6(3).vector='SERCOM6_2';MCHP.module.SERCOM6(3).pin=reshape(MCHP_Fun.Hex2num('[]'),0,0);MCHP.module.SERCOM6(4).PID=73;MCHP.module.SERCOM6(4).vector='SERCOM6_OTHER';MCHP.module.SERCOM6(4).pin=reshape(MCHP_Fun.Hex2num('[]'),0,0);MCHP.module.SERCOM7(1).PID=74;MCHP.module.SERCOM7(1).vector='SERCOM7_0';MCHP.module.SERCOM7(1).pin.PAD0.txt=reshape({ 'PB21','PD08','PB30','PC12'},1,4);MCHP.module.SERCOM7(1).pin.PAD0.Rx_idx=reshape([53 104 62 76],1,4);MCHP.module.SERCOM7(1).pin.PAD0.ABCD=reshape([3 2 2 2],1,4);MCHP.module.SERCOM7(1).pin.PAD1.txt=reshape({ 'PB20','PD09','PB31','PC13'},1,4);MCHP.module.SERCOM7(1).pin.PAD1.Rx_idx=reshape([52 105 63 77],1,4);MCHP.module.SERCOM7(1).pin.PAD1.ABCD=reshape([3 2 2 2],1,4);MCHP.module.SERCOM7(1).pin.PAD2.txt=reshape({ 'PB18','PC10','PC14','PD10','PA30'},1,5);MCHP.module.SERCOM7(1).pin.PAD2.Rx_idx=reshape([50 74 78 106 30],1,5);MCHP.module.SERCOM7(1).pin.PAD2.ABCD=reshape([3 3 2 2 2],1,5);MCHP.module.SERCOM7(1).pin.PAD3.txt=reshape({ 'PB19','PC11','PC15','PD11','PA31'},1,5);MCHP.module.SERCOM7(1).pin.PAD3.Rx_idx=reshape([51 75 79 107 31],1,5);MCHP.module.SERCOM7(1).pin.PAD3.ABCD=reshape([3 3 2 2 2],1,5);MCHP.module.SERCOM7(2).PID=75;MCHP.module.SERCOM7(2).vector='SERCOM7_1';MCHP.module.SERCOM7(2).pin=reshape(MCHP_Fun.Hex2num('[]'),0,0);MCHP.module.SERCOM7(3).PID=76;MCHP.module.SERCOM7(3).vector='SERCOM7_2';MCHP.module.SERCOM7(3).pin=reshape(MCHP_Fun.Hex2num('[]'),0,0);MCHP.module.SERCOM7(4).PID=77;MCHP.module.SERCOM7(4).vector='SERCOM7_OTHER';MCHP.module.SERCOM7(4).pin=reshape(MCHP_Fun.Hex2num('[]'),0,0);MCHP.module.CAN0.PID=78;MCHP.module.CAN0.vector='CAN0';MCHP.module.CAN0.pin.RX.txt=reshape({ 'PA23','PA25'},1,2);MCHP.module.CAN0.pin.RX.Rx_idx=reshape([23 25],1,2);MCHP.module.CAN0.pin.RX.ABCD=reshape([8 8],1,2);MCHP.module.CAN0.pin.TX.txt=reshape({ 'PA22','PA24'},1,2);MCHP.module.CAN0.pin.TX.Rx_idx=reshape([22 24],1,2);MCHP.module.CAN0.pin.TX.ABCD=reshape([8 8],1,2);MCHP.module.CAN1.PID=79;MCHP.module.CAN1.vector='CAN1';MCHP.module.CAN1.pin.RX.txt=reshape({ 'PB13','PB15'},1,2);MCHP.module.CAN1.pin.RX.Rx_idx=reshape([45 47],1,2);MCHP.module.CAN1.pin.RX.ABCD=reshape([7 7],1,2);MCHP.module.CAN1.pin.TX.txt=reshape({ 'PB12','PB14'},1,2);MCHP.module.CAN1.pin.TX.Rx_idx=reshape([44 46],1,2);MCHP.module.CAN1.pin.TX.ABCD=reshape([7 7],1,2);MCHP.module.USB(1).PID=80;MCHP.module.USB(1).vector='USB_OTHER';MCHP.module.USB(1).pin.DM.txt={ 'PA24'};MCHP.module.USB(1).pin.DM.Rx_idx=24;MCHP.module.USB(1).pin.DM.ABCD=7;MCHP.module.USB(1).pin.DP.txt={ 'PA25'};MCHP.module.USB(1).pin.DP.Rx_idx=25;MCHP.module.USB(1).pin.DP.ABCD=7;MCHP.module.USB(1).pin.SOF_1KHZ.txt=reshape({ 'PA23','PB22'},1,2);MCHP.module.USB(1).pin.SOF_1KHZ.Rx_idx=reshape([23 54],1,2);MCHP.module.USB(1).pin.SOF_1KHZ.ABCD=reshape([7 7],1,2);MCHP.module.USB(2).PID=81;MCHP.module.USB(2).vector='USB_SOF_HSOF';MCHP.module.USB(2).pin=reshape(MCHP_Fun.Hex2num('[]'),0,0);MCHP.module.USB(3).PID=82;MCHP.module.USB(3).vector='USB_TRCPT0';MCHP.module.USB(3).pin=reshape(MCHP_Fun.Hex2num('[]'),0,0);MCHP.module.USB(4).PID=83;MCHP.module.USB(4).vector='USB_TRCPT1';MCHP.module.USB(4).pin=reshape(MCHP_Fun.Hex2num('[]'),0,0);MCHP.module.GMAC.PID=84;MCHP.module.GMAC.vector='GMAC';MCHP.module.GMAC.pin.GCOL.txt={ 'PC21'};MCHP.module.GMAC.pin.GCOL.Rx_idx=85;MCHP.module.GMAC.pin.GCOL.ABCD=11;MCHP.module.GMAC.pin.GCRS.txt={ 'PA16'};MCHP.module.GMAC.pin.GCRS.Rx_idx=16;MCHP.module.GMAC.pin.GCRS.ABCD=11;MCHP.module.GMAC.pin.GMDC.txt=reshape({ 'PA20','PB14','PC11','PC22'},1,4);MCHP.module.GMAC.pin.GMDC.Rx_idx=reshape([20 46 75 86],1,4);MCHP.module.GMAC.pin.GMDC.ABCD=reshape([11 11 11 11],1,4);MCHP.module.GMAC.pin.GMDIO.txt=reshape({ 'PA21','PB15','PC12','PC23'},1,4);MCHP.module.GMAC.pin.GMDIO.Rx_idx=reshape([21 47 76 87],1,4);MCHP.module.GMAC.pin.GMDIO.ABCD=reshape([11 11 11 11],1,4);MCHP.module.GMAC.pin.GRX0.txt={ 'PA13'};MCHP.module.GMAC.pin.GRX0.Rx_idx=13;MCHP.module.GMAC.pin.GRX0.ABCD=11;MCHP.module.GMAC.pin.GRX1.txt={ 'PA12'};MCHP.module.GMAC.pin.GRX1.Rx_idx=12;MCHP.module.GMAC.pin.GRX1.ABCD=11;MCHP.module.GMAC.pin.GRX2.txt={ 'PC15'};MCHP.module.GMAC.pin.GRX2.Rx_idx=79;MCHP.module.GMAC.pin.GRX2.ABCD=11;MCHP.module.GMAC.pin.GRX3.txt={ 'PC14'};MCHP.module.GMAC.pin.GRX3.Rx_idx=78;MCHP.module.GMAC.pin.GRX3.ABCD=11;MCHP.module.GMAC.pin.GRXCK.txt={ 'PC18'};MCHP.module.GMAC.pin.GRXCK.Rx_idx=82;MCHP.module.GMAC.pin.GRXCK.ABCD=11;MCHP.module.GMAC.pin.GRXDV.txt={ 'PC20'};MCHP.module.GMAC.pin.GRXDV.Rx_idx=84;MCHP.module.GMAC.pin.GRXDV.ABCD=11;MCHP.module.GMAC.pin.GRXER.txt={ 'PA15'};MCHP.module.GMAC.pin.GRXER.Rx_idx=15;MCHP.module.GMAC.pin.GRXER.ABCD=11;MCHP.module.GMAC.pin.GTX0.txt={ 'PA18'};MCHP.module.GMAC.pin.GTX0.Rx_idx=18;MCHP.module.GMAC.pin.GTX0.ABCD=11;MCHP.module.GMAC.pin.GTX1.txt={ 'PA19'};MCHP.module.GMAC.pin.GTX1.Rx_idx=19;MCHP.module.GMAC.pin.GTX1.ABCD=11;MCHP.module.GMAC.pin.GTX2.txt={ 'PC16'};MCHP.module.GMAC.pin.GTX2.Rx_idx=80;MCHP.module.GMAC.pin.GTX2.ABCD=11;MCHP.module.GMAC.pin.GTX3.txt={ 'PC17'};MCHP.module.GMAC.pin.GTX3.Rx_idx=81;MCHP.module.GMAC.pin.GTX3.ABCD=11;MCHP.module.GMAC.pin.GTXCK.txt={ 'PA14'};MCHP.module.GMAC.pin.GTXCK.Rx_idx=14;MCHP.module.GMAC.pin.GTXCK.ABCD=11;MCHP.module.GMAC.pin.GTXEN.txt={ 'PA17'};MCHP.module.GMAC.pin.GTXEN.Rx_idx=17;MCHP.module.GMAC.pin.GTXEN.ABCD=11;MCHP.module.GMAC.pin.GTXER.txt={ 'PC19'};MCHP.module.GMAC.pin.GTXER.Rx_idx=83;MCHP.module.GMAC.pin.GTXER.ABCD=11;MCHP.module.TCC0(1).PID=85;MCHP.module.TCC0(1).vector='TCC0_OTHER';MCHP.module.TCC0(1).pin.WO0.txt=reshape({ 'PA20','PB12','PA08','PC04','PC10','PC16'},1,6);MCHP.module.TCC0(1).pin.WO0.Rx_idx=reshape([20 44 8 68 74 80],1,6);MCHP.module.TCC0(1).pin.WO0.ABCD=reshape([6 6 5 5 5 5],1,6);MCHP.module.TCC0(1).pin.WO1.txt=reshape({ 'PA21','PB13','PA09','PC11','PC17','PD08'},1,6);MCHP.module.TCC0(1).pin.WO1.Rx_idx=reshape([21 45 9 75 81 104],1,6);MCHP.module.TCC0(1).pin.WO1.ABCD=reshape([6 6 5 5 5 5],1,6);MCHP.module.TCC0(1).pin.WO2.txt=reshape({ 'PA22','PB14','PA10','PC12','PC18','PD09'},1,6);MCHP.module.TCC0(1).pin.WO2.Rx_idx=reshape([22 46 10 76 82 105],1,6);MCHP.module.TCC0(1).pin.WO2.ABCD=reshape([6 6 5 5 5 5],1,6);MCHP.module.TCC0(1).pin.WO3.txt=reshape({ 'PA23','PB15','PA11','PC13','PC19','PD10'},1,6);MCHP.module.TCC0(1).pin.WO3.Rx_idx=reshape([23 47 11 77 83 106],1,6);MCHP.module.TCC0(1).pin.WO3.ABCD=reshape([6 6 5 5 5 5],1,6);MCHP.module.TCC0(1).pin.WO4.txt=reshape({ 'PA16','PB16','PB10','PC14','PC20','PD11'},1,6);MCHP.module.TCC0(1).pin.WO4.Rx_idx=reshape([16 48 42 78 84 107],1,6);MCHP.module.TCC0(1).pin.WO4.ABCD=reshape([6 6 5 5 5 5],1,6);MCHP.module.TCC0(1).pin.WO5.txt=reshape({ 'PA17','PB17','PB11','PC15','PC21','PD12'},1,6);MCHP.module.TCC0(1).pin.WO5.Rx_idx=reshape([17 49 43 79 85 108],1,6);MCHP.module.TCC0(1).pin.WO5.ABCD=reshape([6 6 5 5 5 5],1,6);MCHP.module.TCC0(1).pin.WO6.txt=reshape({ 'PA18','PB30','PA12','PC22'},1,4);MCHP.module.TCC0(1).pin.WO6.Rx_idx=reshape([18 62 12 86],1,4);MCHP.module.TCC0(1).pin.WO6.ABCD=reshape([6 6 5 5],1,4);MCHP.module.TCC0(1).pin.WO7.txt=reshape({ 'PA19','PB31','PA13','PC23'},1,4);MCHP.module.TCC0(1).pin.WO7.Rx_idx=reshape([19 63 13 87],1,4);MCHP.module.TCC0(1).pin.WO7.ABCD=reshape([6 6 5 5],1,4);MCHP.module.TCC0(2).PID=86;MCHP.module.TCC0(2).vector='TCC0_MC0';MCHP.module.TCC0(2).pin=reshape(MCHP_Fun.Hex2num('[]'),0,0);MCHP.module.TCC0(3).PID=87;MCHP.module.TCC0(3).vector='TCC0_MC1';MCHP.module.TCC0(3).pin=reshape(MCHP_Fun.Hex2num('[]'),0,0);MCHP.module.TCC0(4).PID=88;MCHP.module.TCC0(4).vector='TCC0_MC2';MCHP.module.TCC0(4).pin=reshape(MCHP_Fun.Hex2num('[]'),0,0);MCHP.module.TCC0(5).PID=89;MCHP.module.TCC0(5).vector='TCC0_MC3';MCHP.module.TCC0(5).pin=reshape(MCHP_Fun.Hex2num('[]'),0,0);MCHP.module.TCC0(6).PID=90;MCHP.module.TCC0(6).vector='TCC0_MC4';MCHP.module.TCC0(6).pin=reshape(MCHP_Fun.Hex2num('[]'),0,0);MCHP.module.TCC0(7).PID=91;MCHP.module.TCC0(7).vector='TCC0_MC5';MCHP.module.TCC0(7).pin=reshape(MCHP_Fun.Hex2num('[]'),0,0);MCHP.module.TCC1(1).PID=92;MCHP.module.TCC1(1).vector='TCC1_OTHER';MCHP.module.TCC1(1).pin.WO0.txt=reshape({ 'PB10','PC14','PA16','PB18','PD20'},1,5);MCHP.module.TCC1(1).pin.WO0.Rx_idx=reshape([42 78 16 50 116],1,5);MCHP.module.TCC1(1).pin.WO0.ABCD=reshape([6 6 5 5 5],1,5);MCHP.module.TCC1(1).pin.WO1.txt=reshape({ 'PB11','PC15','PA17','PB19','PD21'},1,5);MCHP.module.TCC1(1).pin.WO1.Rx_idx=reshape([43 79 17 51 117],1,5);MCHP.module.TCC1(1).pin.WO1.ABCD=reshape([6 6 5 5 5],1,5);MCHP.module.TCC1(1).pin.WO2.txt=reshape({ 'PA12','PA14','PA18','PB20','PB26'},1,5);MCHP.module.TCC1(1).pin.WO2.Rx_idx=reshape([12 14 18 52 58],1,5);MCHP.module.TCC1(1).pin.WO2.ABCD=reshape([6 6 5 5 5],1,5);MCHP.module.TCC1(1).pin.WO3.txt=reshape({ 'PA13','PA15','PA19','PB21','PB27'},1,5);MCHP.module.TCC1(1).pin.WO3.Rx_idx=reshape([13 15 19 53 59],1,5);MCHP.module.TCC1(1).pin.WO3.ABCD=reshape([6 6 5 5 5],1,5);MCHP.module.TCC1(1).pin.WO4.txt=reshape({ 'PA08','PC10','PA20','PB28'},1,4);MCHP.module.TCC1(1).pin.WO4.Rx_idx=reshape([8 74 20 60],1,4);MCHP.module.TCC1(1).pin.WO4.ABCD=reshape([6 6 5 5],1,4);MCHP.module.TCC1(1).pin.WO5.txt=reshape({ 'PA09','PC11','PA21','PB29'},1,4);MCHP.module.TCC1(1).pin.WO5.Rx_idx=reshape([9 75 21 61],1,4);MCHP.module.TCC1(1).pin.WO5.ABCD=reshape([6 6 5 5],1,4);MCHP.module.TCC1(1).pin.WO6.txt=reshape({ 'PA10','PC12','PA22'},1,3);MCHP.module.TCC1(1).pin.WO6.Rx_idx=reshape([10 76 22],1,3);MCHP.module.TCC1(1).pin.WO6.ABCD=reshape([6 6 5],1,3);MCHP.module.TCC1(1).pin.WO7.txt=reshape({ 'PA11','PC13','PA23'},1,3);MCHP.module.TCC1(1).pin.WO7.Rx_idx=reshape([11 77 23],1,3);MCHP.module.TCC1(1).pin.WO7.ABCD=reshape([6 6 5],1,3);MCHP.module.TCC1(2).PID=93;MCHP.module.TCC1(2).vector='TCC1_MC0';MCHP.module.TCC1(2).pin=reshape(MCHP_Fun.Hex2num('[]'),0,0);MCHP.module.TCC1(3).PID=94;MCHP.module.TCC1(3).vector='TCC1_MC1';MCHP.module.TCC1(3).pin=reshape(MCHP_Fun.Hex2num('[]'),0,0);MCHP.module.TCC1(4).PID=95;MCHP.module.TCC1(4).vector='TCC1_MC2';MCHP.module.TCC1(4).pin=reshape(MCHP_Fun.Hex2num('[]'),0,0);MCHP.module.TCC1(5).PID=96;MCHP.module.TCC1(5).vector='TCC1_MC3';MCHP.module.TCC1(5).pin=reshape(MCHP_Fun.Hex2num('[]'),0,0);MCHP.module.TCC2(1).PID=97;MCHP.module.TCC2(1).vector='TCC2_OTHER';MCHP.module.TCC2(1).pin.WO0.txt=reshape({ 'PA14','PA30'},1,2);MCHP.module.TCC2(1).pin.WO0.Rx_idx=reshape([14 30],1,2);MCHP.module.TCC2(1).pin.WO0.ABCD=reshape([5 5],1,2);MCHP.module.TCC2(1).pin.WO1.txt=reshape({ 'PA15','PA31'},1,2);MCHP.module.TCC2(1).pin.WO1.Rx_idx=reshape([15 31],1,2);MCHP.module.TCC2(1).pin.WO1.ABCD=reshape([5 5],1,2);MCHP.module.TCC2(1).pin.WO2.txt=reshape({ 'PA24','PB02'},1,2);MCHP.module.TCC2(1).pin.WO2.Rx_idx=reshape([24 34],1,2);MCHP.module.TCC2(1).pin.WO2.ABCD=reshape([5 5],1,2);MCHP.module.TCC2(2).PID=98;MCHP.module.TCC2(2).vector='TCC2_MC0';MCHP.module.TCC2(2).pin=reshape(MCHP_Fun.Hex2num('[]'),0,0);MCHP.module.TCC2(3).PID=99;MCHP.module.TCC2(3).vector='TCC2_MC1';MCHP.module.TCC2(3).pin=reshape(MCHP_Fun.Hex2num('[]'),0,0);MCHP.module.TCC2(4).PID=100;MCHP.module.TCC2(4).vector='TCC2_MC2';MCHP.module.TCC2(4).pin=reshape(MCHP_Fun.Hex2num('[]'),0,0);MCHP.module.TCC3(1).PID=101;MCHP.module.TCC3(1).vector='TCC3_OTHER';MCHP.module.TCC3(1).pin.WO0.txt=reshape({ 'PB12','PB16'},1,2);MCHP.module.TCC3(1).pin.WO0.Rx_idx=reshape([44 48],1,2);MCHP.module.TCC3(1).pin.WO0.ABCD=reshape([5 5],1,2);MCHP.module.TCC3(1).pin.WO1.txt=reshape({ 'PB13','PB17'},1,2);MCHP.module.TCC3(1).pin.WO1.Rx_idx=reshape([45 49],1,2);MCHP.module.TCC3(1).pin.WO1.ABCD=reshape([5 5],1,2);MCHP.module.TCC3(2).PID=102;MCHP.module.TCC3(2).vector='TCC3_MC0';MCHP.module.TCC3(2).pin=reshape(MCHP_Fun.Hex2num('[]'),0,0);MCHP.module.TCC3(3).PID=103;MCHP.module.TCC3(3).vector='TCC3_MC1';MCHP.module.TCC3(3).pin=reshape(MCHP_Fun.Hex2num('[]'),0,0);MCHP.module.TCC4(1).PID=104;MCHP.module.TCC4(1).vector='TCC4_OTHER';MCHP.module.TCC4(1).pin.WO0.txt=reshape({ 'PB14','PB30'},1,2);MCHP.module.TCC4(1).pin.WO0.Rx_idx=reshape([46 62],1,2);MCHP.module.TCC4(1).pin.WO0.ABCD=reshape([5 5],1,2);MCHP.module.TCC4(1).pin.WO1.txt=reshape({ 'PB15','PB31'},1,2);MCHP.module.TCC4(1).pin.WO1.Rx_idx=reshape([47 63],1,2);MCHP.module.TCC4(1).pin.WO1.ABCD=reshape([5 5],1,2);MCHP.module.TCC4(2).PID=105;MCHP.module.TCC4(2).vector='TCC4_MC0';MCHP.module.TCC4(2).pin=reshape(MCHP_Fun.Hex2num('[]'),0,0);MCHP.module.TCC4(3).PID=106;MCHP.module.TCC4(3).vector='TCC4_MC1';MCHP.module.TCC4(3).pin=reshape(MCHP_Fun.Hex2num('[]'),0,0);MCHP.module.TC0.PID=107;MCHP.module.TC0.vector='TC0';MCHP.module.TC0.pin.WO0.txt=reshape({ 'PA04','PA08','PB30'},1,3);MCHP.module.TC0.pin.WO0.Rx_idx=reshape([4 8 62],1,3);MCHP.module.TC0.pin.WO0.ABCD=reshape([4 4 4],1,3);MCHP.module.TC0.pin.WO1.txt=reshape({ 'PA05','PA09','PB31'},1,3);MCHP.module.TC0.pin.WO1.Rx_idx=reshape([5 9 63],1,3);MCHP.module.TC0.pin.WO1.ABCD=reshape([4 4 4],1,3);MCHP.module.TC1.PID=108;MCHP.module.TC1.vector='TC1';MCHP.module.TC1.pin.WO0.txt=reshape({ 'PA06','PA10'},1,2);MCHP.module.TC1.pin.WO0.Rx_idx=reshape([6 10],1,2);MCHP.module.TC1.pin.WO0.ABCD=reshape([4 4],1,2);MCHP.module.TC1.pin.WO1.txt=reshape({ 'PA07','PA11'},1,2);MCHP.module.TC1.pin.WO1.Rx_idx=reshape([7 11],1,2);MCHP.module.TC1.pin.WO1.ABCD=reshape([4 4],1,2);MCHP.module.TC2.PID=109;MCHP.module.TC2.vector='TC2';MCHP.module.TC2.pin.WO0.txt=reshape({ 'PA12','PA16','PA00'},1,3);MCHP.module.TC2.pin.WO0.Rx_idx=reshape([12 16 0],1,3);MCHP.module.TC2.pin.WO0.ABCD=reshape([4 4 4],1,3);MCHP.module.TC2.pin.WO1.txt=reshape({ 'PA01','PA13','PA17'},1,3);MCHP.module.TC2.pin.WO1.Rx_idx=reshape([1 13 17],1,3);MCHP.module.TC2.pin.WO1.ABCD=reshape([4 4 4],1,3);MCHP.module.TC3.PID=110;MCHP.module.TC3.vector='TC3';MCHP.module.TC3.pin.WO0.txt=reshape({ 'PA18','PA14'},1,2);MCHP.module.TC3.pin.WO0.Rx_idx=reshape([18 14],1,2);MCHP.module.TC3.pin.WO0.ABCD=reshape([4 4],1,2);MCHP.module.TC3.pin.WO1.txt=reshape({ 'PA15','PA19'},1,2);MCHP.module.TC3.pin.WO1.Rx_idx=reshape([15 19],1,2);MCHP.module.TC3.pin.WO1.ABCD=reshape([4 4],1,2);MCHP.module.TC4.PID=111;MCHP.module.TC4.vector='TC4';MCHP.module.TC4.pin.WO0.txt=reshape({ 'PA22','PB08','PB12'},1,3);MCHP.module.TC4.pin.WO0.Rx_idx=reshape([22 40 44],1,3);MCHP.module.TC4.pin.WO0.ABCD=reshape([4 4 4],1,3);MCHP.module.TC4.pin.WO1.txt=reshape({ 'PA23','PB09','PB13'},1,3);MCHP.module.TC4.pin.WO1.Rx_idx=reshape([23 41 45],1,3);MCHP.module.TC4.pin.WO1.ABCD=reshape([4 4 4],1,3);MCHP.module.TC5.PID=112;MCHP.module.TC5.vector='TC5';MCHP.module.TC5.pin.WO0.txt=reshape({ 'PA24','PB10','PB14'},1,3);MCHP.module.TC5.pin.WO0.Rx_idx=reshape([24 42 46],1,3);MCHP.module.TC5.pin.WO0.ABCD=reshape([4 4 4],1,3);MCHP.module.TC5.pin.WO1.txt=reshape({ 'PA25','PB11','PB15'},1,3);MCHP.module.TC5.pin.WO1.Rx_idx=reshape([25 43 47],1,3);MCHP.module.TC5.pin.WO1.ABCD=reshape([4 4 4],1,3);MCHP.module.TC6.PID=113;MCHP.module.TC6.vector='TC6';MCHP.module.TC6.pin.WO0.txt=reshape({ 'PA30','PB02','PB16'},1,3);MCHP.module.TC6.pin.WO0.Rx_idx=reshape([30 34 48],1,3);MCHP.module.TC6.pin.WO0.ABCD=reshape([4 4 4],1,3);MCHP.module.TC6.pin.WO1.txt=reshape({ 'PA31','PB03','PB17'},1,3);MCHP.module.TC6.pin.WO1.Rx_idx=reshape([31 35 49],1,3);MCHP.module.TC6.pin.WO1.ABCD=reshape([4 4 4],1,3);MCHP.module.TC7.PID=114;MCHP.module.TC7.vector='TC7';MCHP.module.TC7.pin.WO0.txt=reshape({ 'PA20','PB00','PB22'},1,3);MCHP.module.TC7.pin.WO0.Rx_idx=reshape([20 32 54],1,3);MCHP.module.TC7.pin.WO0.ABCD=reshape([4 4 4],1,3);MCHP.module.TC7.pin.WO1.txt=reshape({ 'PA21','PB01','PB23'},1,3);MCHP.module.TC7.pin.WO1.Rx_idx=reshape([21 33 55],1,3);MCHP.module.TC7.pin.WO1.ABCD=reshape([4 4 4],1,3);MCHP.module.PDEC(1).PID=115;MCHP.module.PDEC(1).vector='PDEC_OTHER';MCHP.module.PDEC(1).pin.QDI0.txt=reshape({ 'PB18','PB23','PC16','PA24'},1,4);MCHP.module.PDEC(1).pin.QDI0.Rx_idx=reshape([50 55 80 24],1,4);MCHP.module.PDEC(1).pin.QDI0.ABCD=reshape([6 6 6 6],1,4);MCHP.module.PDEC(1).pin.QDI1.txt=reshape({ 'PB19','PB24','PC17','PA25'},1,4);MCHP.module.PDEC(1).pin.QDI1.Rx_idx=reshape([51 56 81 25],1,4);MCHP.module.PDEC(1).pin.QDI1.ABCD=reshape([6 6 6 6],1,4);MCHP.module.PDEC(1).pin.QDI2.txt=reshape({ 'PB20','PB25','PC18','PB22'},1,4);MCHP.module.PDEC(1).pin.QDI2.Rx_idx=reshape([52 57 82 54],1,4);MCHP.module.PDEC(1).pin.QDI2.ABCD=reshape([6 6 6 6],1,4);MCHP.module.PDEC(2).PID=116;MCHP.module.PDEC(2).vector='PDEC_MC0';MCHP.module.PDEC(2).pin=reshape(MCHP_Fun.Hex2num('[]'),0,0);MCHP.module.PDEC(3).PID=117;MCHP.module.PDEC(3).vector='PDEC_MC1';MCHP.module.PDEC(3).pin=reshape(MCHP_Fun.Hex2num('[]'),0,0);MCHP.module.ADC0(1).PID=118;MCHP.module.ADC0(1).vector='ADC0_OTHER';MCHP.module.ADC0(1).pin.AIN0.txt={ 'PA02'};MCHP.module.ADC0(1).pin.AIN0.Rx_idx=2;MCHP.module.ADC0(1).pin.AIN0.ABCD=1;MCHP.module.ADC0(1).pin.AIN1.txt={ 'PA03'};MCHP.module.ADC0(1).pin.AIN1.Rx_idx=3;MCHP.module.ADC0(1).pin.AIN1.ABCD=1;MCHP.module.ADC0(1).pin.AIN2.txt={ 'PB08'};MCHP.module.ADC0(1).pin.AIN2.Rx_idx=40;MCHP.module.ADC0(1).pin.AIN2.ABCD=1;MCHP.module.ADC0(1).pin.AIN3.txt={ 'PB09'};MCHP.module.ADC0(1).pin.AIN3.Rx_idx=41;MCHP.module.ADC0(1).pin.AIN3.ABCD=1;MCHP.module.ADC0(1).pin.AIN4.txt={ 'PA04'};MCHP.module.ADC0(1).pin.AIN4.Rx_idx=4;MCHP.module.ADC0(1).pin.AIN4.ABCD=1;MCHP.module.ADC0(1).pin.AIN5.txt={ 'PA05'};MCHP.module.ADC0(1).pin.AIN5.Rx_idx=5;MCHP.module.ADC0(1).pin.AIN5.ABCD=1;MCHP.module.ADC0(1).pin.AIN6.txt={ 'PA06'};MCHP.module.ADC0(1).pin.AIN6.Rx_idx=6;MCHP.module.ADC0(1).pin.AIN6.ABCD=1;MCHP.module.ADC0(1).pin.AIN7.txt={ 'PA07'};MCHP.module.ADC0(1).pin.AIN7.Rx_idx=7;MCHP.module.ADC0(1).pin.AIN7.ABCD=1;MCHP.module.ADC0(1).pin.AIN8.txt={ 'PA08'};MCHP.module.ADC0(1).pin.AIN8.Rx_idx=8;MCHP.module.ADC0(1).pin.AIN8.ABCD=1;MCHP.module.ADC0(1).pin.AIN9.txt={ 'PA09'};MCHP.module.ADC0(1).pin.AIN9.Rx_idx=9;MCHP.module.ADC0(1).pin.AIN9.ABCD=1;MCHP.module.ADC0(1).pin.AIN10.txt={ 'PA10'};MCHP.module.ADC0(1).pin.AIN10.Rx_idx=10;MCHP.module.ADC0(1).pin.AIN10.ABCD=1;MCHP.module.ADC0(1).pin.AIN11.txt={ 'PA11'};MCHP.module.ADC0(1).pin.AIN11.Rx_idx=11;MCHP.module.ADC0(1).pin.AIN11.ABCD=1;MCHP.module.ADC0(1).pin.AIN12.txt={ 'PB00'};MCHP.module.ADC0(1).pin.AIN12.Rx_idx=32;MCHP.module.ADC0(1).pin.AIN12.ABCD=1;MCHP.module.ADC0(1).pin.AIN13.txt={ 'PB01'};MCHP.module.ADC0(1).pin.AIN13.Rx_idx=33;MCHP.module.ADC0(1).pin.AIN13.ABCD=1;MCHP.module.ADC0(1).pin.AIN14.txt={ 'PB02'};MCHP.module.ADC0(1).pin.AIN14.Rx_idx=34;MCHP.module.ADC0(1).pin.AIN14.ABCD=1;MCHP.module.ADC0(1).pin.AIN15.txt={ 'PB03'};MCHP.module.ADC0(1).pin.AIN15.Rx_idx=35;MCHP.module.ADC0(1).pin.AIN15.ABCD=1;MCHP.module.ADC0(1).pin.X0.txt={ 'PA03'};MCHP.module.ADC0(1).pin.X0.Rx_idx=3;MCHP.module.ADC0(1).pin.X0.ABCD=1;MCHP.module.ADC0(1).pin.Y0.txt={ 'PA03'};MCHP.module.ADC0(1).pin.Y0.Rx_idx=3;MCHP.module.ADC0(1).pin.Y0.ABCD=1;MCHP.module.ADC0(1).pin.X1.txt={ 'PB08'};MCHP.module.ADC0(1).pin.X1.Rx_idx=40;MCHP.module.ADC0(1).pin.X1.ABCD=1;MCHP.module.ADC0(1).pin.Y1.txt={ 'PB08'};MCHP.module.ADC0(1).pin.Y1.Rx_idx=40;MCHP.module.ADC0(1).pin.Y1.ABCD=1;MCHP.module.ADC0(1).pin.X2.txt={ 'PB09'};MCHP.module.ADC0(1).pin.X2.Rx_idx=41;MCHP.module.ADC0(1).pin.X2.ABCD=1;MCHP.module.ADC0(1).pin.Y2.txt={ 'PB09'};MCHP.module.ADC0(1).pin.Y2.Rx_idx=41;MCHP.module.ADC0(1).pin.Y2.ABCD=1;MCHP.module.ADC0(1).pin.X3.txt={ 'PA04'};MCHP.module.ADC0(1).pin.X3.Rx_idx=4;MCHP.module.ADC0(1).pin.X3.ABCD=1;MCHP.module.ADC0(1).pin.Y3.txt={ 'PA04'};MCHP.module.ADC0(1).pin.Y3.Rx_idx=4;MCHP.module.ADC0(1).pin.Y3.ABCD=1;MCHP.module.ADC0(1).pin.X4.txt={ 'PA06'};MCHP.module.ADC0(1).pin.X4.Rx_idx=6;MCHP.module.ADC0(1).pin.X4.ABCD=1;MCHP.module.ADC0(1).pin.Y4.txt={ 'PA06'};MCHP.module.ADC0(1).pin.Y4.Rx_idx=6;MCHP.module.ADC0(1).pin.Y4.ABCD=1;MCHP.module.ADC0(1).pin.X5.txt={ 'PA07'};MCHP.module.ADC0(1).pin.X5.Rx_idx=7;MCHP.module.ADC0(1).pin.X5.ABCD=1;MCHP.module.ADC0(1).pin.Y5.txt={ 'PA07'};MCHP.module.ADC0(1).pin.Y5.Rx_idx=7;MCHP.module.ADC0(1).pin.Y5.ABCD=1;MCHP.module.ADC0(1).pin.X6.txt={ 'PA08'};MCHP.module.ADC0(1).pin.X6.Rx_idx=8;MCHP.module.ADC0(1).pin.X6.ABCD=1;MCHP.module.ADC0(1).pin.Y6.txt={ 'PA08'};MCHP.module.ADC0(1).pin.Y6.Rx_idx=8;MCHP.module.ADC0(1).pin.Y6.ABCD=1;MCHP.module.ADC0(1).pin.X7.txt={ 'PA09'};MCHP.module.ADC0(1).pin.X7.Rx_idx=9;MCHP.module.ADC0(1).pin.X7.ABCD=1;MCHP.module.ADC0(1).pin.Y7.txt={ 'PA09'};MCHP.module.ADC0(1).pin.Y7.Rx_idx=9;MCHP.module.ADC0(1).pin.Y7.ABCD=1;MCHP.module.ADC0(1).pin.X8.txt={ 'PA10'};MCHP.module.ADC0(1).pin.X8.Rx_idx=10;MCHP.module.ADC0(1).pin.X8.ABCD=1;MCHP.module.ADC0(1).pin.Y8.txt={ 'PA10'};MCHP.module.ADC0(1).pin.Y8.Rx_idx=10;MCHP.module.ADC0(1).pin.Y8.ABCD=1;MCHP.module.ADC0(1).pin.X9.txt={ 'PA11'};MCHP.module.ADC0(1).pin.X9.Rx_idx=11;MCHP.module.ADC0(1).pin.X9.ABCD=1;MCHP.module.ADC0(1).pin.Y9.txt={ 'PA11'};MCHP.module.ADC0(1).pin.Y9.Rx_idx=11;MCHP.module.ADC0(1).pin.Y9.ABCD=1;MCHP.module.ADC0(1).pin.X10.txt={ 'PA16'};MCHP.module.ADC0(1).pin.X10.Rx_idx=16;MCHP.module.ADC0(1).pin.X10.ABCD=1;MCHP.module.ADC0(1).pin.Y10.txt={ 'PA16'};MCHP.module.ADC0(1).pin.Y10.Rx_idx=16;MCHP.module.ADC0(1).pin.Y10.ABCD=1;MCHP.module.ADC0(1).pin.X11.txt={ 'PA17'};MCHP.module.ADC0(1).pin.X11.Rx_idx=17;MCHP.module.ADC0(1).pin.X11.ABCD=1;MCHP.module.ADC0(1).pin.Y11.txt={ 'PA17'};MCHP.module.ADC0(1).pin.Y11.Rx_idx=17;MCHP.module.ADC0(1).pin.Y11.ABCD=1;MCHP.module.ADC0(1).pin.X12.txt={ 'PA18'};MCHP.module.ADC0(1).pin.X12.Rx_idx=18;MCHP.module.ADC0(1).pin.X12.ABCD=1;MCHP.module.ADC0(1).pin.Y12.txt={ 'PA18'};MCHP.module.ADC0(1).pin.Y12.Rx_idx=18;MCHP.module.ADC0(1).pin.Y12.ABCD=1;MCHP.module.ADC0(1).pin.X13.txt={ 'PA19'};MCHP.module.ADC0(1).pin.X13.Rx_idx=19;MCHP.module.ADC0(1).pin.X13.ABCD=1;MCHP.module.ADC0(1).pin.Y13.txt={ 'PA19'};MCHP.module.ADC0(1).pin.Y13.Rx_idx=19;MCHP.module.ADC0(1).pin.Y13.ABCD=1;MCHP.module.ADC0(1).pin.X14.txt={ 'PA20'};MCHP.module.ADC0(1).pin.X14.Rx_idx=20;MCHP.module.ADC0(1).pin.X14.ABCD=1;MCHP.module.ADC0(1).pin.Y14.txt={ 'PA20'};MCHP.module.ADC0(1).pin.Y14.Rx_idx=20;MCHP.module.ADC0(1).pin.Y14.ABCD=1;MCHP.module.ADC0(1).pin.X15.txt={ 'PA21'};MCHP.module.ADC0(1).pin.X15.Rx_idx=21;MCHP.module.ADC0(1).pin.X15.ABCD=1;MCHP.module.ADC0(1).pin.Y15.txt={ 'PA21'};MCHP.module.ADC0(1).pin.Y15.Rx_idx=21;MCHP.module.ADC0(1).pin.Y15.ABCD=1;MCHP.module.ADC0(1).pin.X16.txt={ 'PA22'};MCHP.module.ADC0(1).pin.X16.Rx_idx=22;MCHP.module.ADC0(1).pin.X16.ABCD=1;MCHP.module.ADC0(1).pin.Y16.txt={ 'PA22'};MCHP.module.ADC0(1).pin.Y16.Rx_idx=22;MCHP.module.ADC0(1).pin.Y16.ABCD=1;MCHP.module.ADC0(1).pin.X17.txt={ 'PA23'};MCHP.module.ADC0(1).pin.X17.Rx_idx=23;MCHP.module.ADC0(1).pin.X17.ABCD=1;MCHP.module.ADC0(1).pin.Y17.txt={ 'PA23'};MCHP.module.ADC0(1).pin.Y17.Rx_idx=23;MCHP.module.ADC0(1).pin.Y17.ABCD=1;MCHP.module.ADC0(1).pin.X18.txt={ 'PA27'};MCHP.module.ADC0(1).pin.X18.Rx_idx=27;MCHP.module.ADC0(1).pin.X18.ABCD=1;MCHP.module.ADC0(1).pin.Y18.txt={ 'PA27'};MCHP.module.ADC0(1).pin.Y18.Rx_idx=27;MCHP.module.ADC0(1).pin.Y18.ABCD=1;MCHP.module.ADC0(1).pin.X19.txt={ 'PA30'};MCHP.module.ADC0(1).pin.X19.Rx_idx=30;MCHP.module.ADC0(1).pin.X19.ABCD=1;MCHP.module.ADC0(1).pin.Y19.txt={ 'PA30'};MCHP.module.ADC0(1).pin.Y19.Rx_idx=30;MCHP.module.ADC0(1).pin.Y19.ABCD=1;MCHP.module.ADC0(1).pin.X20.txt={ 'PB02'};MCHP.module.ADC0(1).pin.X20.Rx_idx=34;MCHP.module.ADC0(1).pin.X20.ABCD=1;MCHP.module.ADC0(1).pin.Y20.txt={ 'PB02'};MCHP.module.ADC0(1).pin.Y20.Rx_idx=34;MCHP.module.ADC0(1).pin.Y20.ABCD=1;MCHP.module.ADC0(1).pin.X21.txt={ 'PB03'};MCHP.module.ADC0(1).pin.X21.Rx_idx=35;MCHP.module.ADC0(1).pin.X21.ABCD=1;MCHP.module.ADC0(1).pin.Y21.txt={ 'PB03'};MCHP.module.ADC0(1).pin.Y21.Rx_idx=35;MCHP.module.ADC0(1).pin.Y21.ABCD=1;MCHP.module.ADC0(1).pin.X22.txt={ 'PB04'};MCHP.module.ADC0(1).pin.X22.Rx_idx=36;MCHP.module.ADC0(1).pin.X22.ABCD=1;MCHP.module.ADC0(1).pin.Y22.txt={ 'PB04'};MCHP.module.ADC0(1).pin.Y22.Rx_idx=36;MCHP.module.ADC0(1).pin.Y22.ABCD=1;MCHP.module.ADC0(1).pin.X23.txt={ 'PB05'};MCHP.module.ADC0(1).pin.X23.Rx_idx=37;MCHP.module.ADC0(1).pin.X23.ABCD=1;MCHP.module.ADC0(1).pin.Y23.txt={ 'PB05'};MCHP.module.ADC0(1).pin.Y23.Rx_idx=37;MCHP.module.ADC0(1).pin.Y23.ABCD=1;MCHP.module.ADC0(1).pin.X24.txt={ 'PB06'};MCHP.module.ADC0(1).pin.X24.Rx_idx=38;MCHP.module.ADC0(1).pin.X24.ABCD=1;MCHP.module.ADC0(1).pin.Y24.txt={ 'PB06'};MCHP.module.ADC0(1).pin.Y24.Rx_idx=38;MCHP.module.ADC0(1).pin.Y24.ABCD=1;MCHP.module.ADC0(1).pin.X25.txt={ 'PB07'};MCHP.module.ADC0(1).pin.X25.Rx_idx=39;MCHP.module.ADC0(1).pin.X25.ABCD=1;MCHP.module.ADC0(1).pin.Y25.txt={ 'PB07'};MCHP.module.ADC0(1).pin.Y25.Rx_idx=39;MCHP.module.ADC0(1).pin.Y25.ABCD=1;MCHP.module.ADC0(1).pin.X26.txt={ 'PB12'};MCHP.module.ADC0(1).pin.X26.Rx_idx=44;MCHP.module.ADC0(1).pin.X26.ABCD=1;MCHP.module.ADC0(1).pin.Y26.txt={ 'PB12'};MCHP.module.ADC0(1).pin.Y26.Rx_idx=44;MCHP.module.ADC0(1).pin.Y26.ABCD=1;MCHP.module.ADC0(1).pin.X27.txt={ 'PB13'};MCHP.module.ADC0(1).pin.X27.Rx_idx=45;MCHP.module.ADC0(1).pin.X27.ABCD=1;MCHP.module.ADC0(1).pin.Y27.txt={ 'PB13'};MCHP.module.ADC0(1).pin.Y27.Rx_idx=45;MCHP.module.ADC0(1).pin.Y27.ABCD=1;MCHP.module.ADC0(1).pin.X28.txt={ 'PB14'};MCHP.module.ADC0(1).pin.X28.Rx_idx=46;MCHP.module.ADC0(1).pin.X28.ABCD=1;MCHP.module.ADC0(1).pin.Y28.txt={ 'PB14'};MCHP.module.ADC0(1).pin.Y28.Rx_idx=46;MCHP.module.ADC0(1).pin.Y28.ABCD=1;MCHP.module.ADC0(1).pin.X29.txt={ 'PB15'};MCHP.module.ADC0(1).pin.X29.Rx_idx=47;MCHP.module.ADC0(1).pin.X29.ABCD=1;MCHP.module.ADC0(1).pin.Y29.txt={ 'PB15'};MCHP.module.ADC0(1).pin.Y29.Rx_idx=47;MCHP.module.ADC0(1).pin.Y29.ABCD=1;MCHP.module.ADC0(1).pin.X30.txt={ 'PB00'};MCHP.module.ADC0(1).pin.X30.Rx_idx=32;MCHP.module.ADC0(1).pin.X30.ABCD=1;MCHP.module.ADC0(1).pin.Y30.txt={ 'PB00'};MCHP.module.ADC0(1).pin.Y30.Rx_idx=32;MCHP.module.ADC0(1).pin.Y30.ABCD=1;MCHP.module.ADC0(1).pin.X31.txt={ 'PB01'};MCHP.module.ADC0(1).pin.X31.Rx_idx=33;MCHP.module.ADC0(1).pin.X31.ABCD=1;MCHP.module.ADC0(1).pin.Y31.txt={ 'PB01'};MCHP.module.ADC0(1).pin.Y31.Rx_idx=33;MCHP.module.ADC0(1).pin.Y31.ABCD=1;MCHP.module.ADC0(1).pin.VREFA.txt={ 'PA03'};MCHP.module.ADC0(1).pin.VREFA.Rx_idx=3;MCHP.module.ADC0(1).pin.VREFA.ABCD=1;MCHP.module.ADC0(1).pin.VREFB.txt={ 'PA04'};MCHP.module.ADC0(1).pin.VREFB.Rx_idx=4;MCHP.module.ADC0(1).pin.VREFB.ABCD=1;MCHP.module.ADC0(1).pin.VREFC.txt={ 'PA06'};MCHP.module.ADC0(1).pin.VREFC.Rx_idx=6;MCHP.module.ADC0(1).pin.VREFC.ABCD=1;MCHP.module.ADC0(2).PID=119;MCHP.module.ADC0(2).vector='ADC0_RESRDY';MCHP.module.ADC0(2).pin=reshape(MCHP_Fun.Hex2num('[]'),0,0);MCHP.module.ADC1(1).PID=120;MCHP.module.ADC1(1).vector='ADC1_OTHER';MCHP.module.ADC1(1).pin.AIN0.txt={ 'PB08'};MCHP.module.ADC1(1).pin.AIN0.Rx_idx=40;MCHP.module.ADC1(1).pin.AIN0.ABCD=1;MCHP.module.ADC1(1).pin.AIN1.txt={ 'PB09'};MCHP.module.ADC1(1).pin.AIN1.Rx_idx=41;MCHP.module.ADC1(1).pin.AIN1.ABCD=1;MCHP.module.ADC1(1).pin.AIN2.txt={ 'PA08'};MCHP.module.ADC1(1).pin.AIN2.Rx_idx=8;MCHP.module.ADC1(1).pin.AIN2.ABCD=1;MCHP.module.ADC1(1).pin.AIN3.txt={ 'PA09'};MCHP.module.ADC1(1).pin.AIN3.Rx_idx=9;MCHP.module.ADC1(1).pin.AIN3.ABCD=1;MCHP.module.ADC1(1).pin.AIN4.txt={ 'PC02'};MCHP.module.ADC1(1).pin.AIN4.Rx_idx=66;MCHP.module.ADC1(1).pin.AIN4.ABCD=1;MCHP.module.ADC1(1).pin.AIN5.txt={ 'PC03'};MCHP.module.ADC1(1).pin.AIN5.Rx_idx=67;MCHP.module.ADC1(1).pin.AIN5.ABCD=1;MCHP.module.ADC1(1).pin.AIN6.txt={ 'PB04'};MCHP.module.ADC1(1).pin.AIN6.Rx_idx=36;MCHP.module.ADC1(1).pin.AIN6.ABCD=1;MCHP.module.ADC1(1).pin.AIN7.txt={ 'PB05'};MCHP.module.ADC1(1).pin.AIN7.Rx_idx=37;MCHP.module.ADC1(1).pin.AIN7.ABCD=1;MCHP.module.ADC1(1).pin.AIN8.txt={ 'PB06'};MCHP.module.ADC1(1).pin.AIN8.Rx_idx=38;MCHP.module.ADC1(1).pin.AIN8.ABCD=1;MCHP.module.ADC1(1).pin.AIN9.txt={ 'PB07'};MCHP.module.ADC1(1).pin.AIN9.Rx_idx=39;MCHP.module.ADC1(1).pin.AIN9.ABCD=1;MCHP.module.ADC1(1).pin.AIN10.txt={ 'PC00'};MCHP.module.ADC1(1).pin.AIN10.Rx_idx=64;MCHP.module.ADC1(1).pin.AIN10.ABCD=1;MCHP.module.ADC1(1).pin.AIN11.txt={ 'PC01'};MCHP.module.ADC1(1).pin.AIN11.Rx_idx=65;MCHP.module.ADC1(1).pin.AIN11.ABCD=1;MCHP.module.ADC1(1).pin.AIN12.txt={ 'PC30'};MCHP.module.ADC1(1).pin.AIN12.Rx_idx=94;MCHP.module.ADC1(1).pin.AIN12.ABCD=1;MCHP.module.ADC1(1).pin.AIN13.txt={ 'PC31'};MCHP.module.ADC1(1).pin.AIN13.Rx_idx=95;MCHP.module.ADC1(1).pin.AIN13.ABCD=1;MCHP.module.ADC1(1).pin.AIN14.txt={ 'PD00'};MCHP.module.ADC1(1).pin.AIN14.Rx_idx=96;MCHP.module.ADC1(1).pin.AIN14.ABCD=1;MCHP.module.ADC1(1).pin.AIN15.txt={ 'PD01'};MCHP.module.ADC1(1).pin.AIN15.Rx_idx=97;MCHP.module.ADC1(1).pin.AIN15.ABCD=1;MCHP.module.ADC1(2).PID=121;MCHP.module.ADC1(2).vector='ADC1_RESRDY';MCHP.module.ADC1(2).pin=reshape(MCHP_Fun.Hex2num('[]'),0,0);MCHP.module.AC.PID=122;MCHP.module.AC.vector='AC';MCHP.module.AC.pin.AIN0.txt={ 'PA04'};MCHP.module.AC.pin.AIN0.Rx_idx=4;MCHP.module.AC.pin.AIN0.ABCD=1;MCHP.module.AC.pin.AIN1.txt={ 'PA05'};MCHP.module.AC.pin.AIN1.Rx_idx=5;MCHP.module.AC.pin.AIN1.ABCD=1;MCHP.module.AC.pin.AIN2.txt={ 'PA06'};MCHP.module.AC.pin.AIN2.Rx_idx=6;MCHP.module.AC.pin.AIN2.ABCD=1;MCHP.module.AC.pin.AIN3.txt={ 'PA07'};MCHP.module.AC.pin.AIN3.Rx_idx=7;MCHP.module.AC.pin.AIN3.ABCD=1;MCHP.module.AC.pin.CMP0.txt=reshape({ 'PA12','PA18','PB24'},1,3);MCHP.module.AC.pin.CMP0.Rx_idx=reshape([12 18 56],1,3);MCHP.module.AC.pin.CMP0.ABCD=reshape([12 12 12],1,3);MCHP.module.AC.pin.CMP1.txt=reshape({ 'PA13','PA19','PB25'},1,3);MCHP.module.AC.pin.CMP1.Rx_idx=reshape([13 19 57],1,3);MCHP.module.AC.pin.CMP1.ABCD=reshape([12 12 12],1,3);MCHP.module.DAC(1).PID=123;MCHP.module.DAC(1).vector='DAC_OTHER';MCHP.module.DAC(1).pin.VOUT0.txt={ 'PA02'};MCHP.module.DAC(1).pin.VOUT0.Rx_idx=2;MCHP.module.DAC(1).pin.VOUT0.ABCD=1;MCHP.module.DAC(1).pin.VOUT1.txt={ 'PA05'};MCHP.module.DAC(1).pin.VOUT1.Rx_idx=5;MCHP.module.DAC(1).pin.VOUT1.ABCD=1;MCHP.module.DAC(2).PID=124;MCHP.module.DAC(2).vector='DAC_EMPTY_0';MCHP.module.DAC(2).pin=reshape(MCHP_Fun.Hex2num('[]'),0,0);MCHP.module.DAC(3).PID=125;MCHP.module.DAC(3).vector='DAC_EMPTY_1';MCHP.module.DAC(3).pin=reshape(MCHP_Fun.Hex2num('[]'),0,0);MCHP.module.DAC(4).PID=126;MCHP.module.DAC(4).vector='DAC_RESRDY_0';MCHP.module.DAC(4).pin=reshape(MCHP_Fun.Hex2num('[]'),0,0);MCHP.module.DAC(5).PID=127;MCHP.module.DAC(5).vector='DAC_RESRDY_1';MCHP.module.DAC(5).pin=reshape(MCHP_Fun.Hex2num('[]'),0,0);MCHP.module.I2S.PID=128;MCHP.module.I2S.vector='I2S';MCHP.module.I2S.pin.FS0.txt=reshape({ 'PA09','PA20'},1,2);MCHP.module.I2S.pin.FS0.Rx_idx=reshape([9 20],1,2);MCHP.module.I2S.pin.FS0.ABCD=reshape([9 9],1,2);MCHP.module.I2S.pin.FS1.txt=reshape({ 'PA23','PB11'},1,2);MCHP.module.I2S.pin.FS1.Rx_idx=reshape([23 43],1,2);MCHP.module.I2S.pin.FS1.ABCD=reshape([9 9],1,2);MCHP.module.I2S.pin.MCK0.txt=reshape({ 'PA08','PB17'},1,2);MCHP.module.I2S.pin.MCK0.Rx_idx=reshape([8 49],1,2);MCHP.module.I2S.pin.MCK0.ABCD=reshape([9 9],1,2);MCHP.module.I2S.pin.MCK1.txt=reshape({ 'PB29','PB13'},1,2);MCHP.module.I2S.pin.MCK1.Rx_idx=reshape([61 45],1,2);MCHP.module.I2S.pin.MCK1.ABCD=reshape([9 9],1,2);MCHP.module.I2S.pin.SCK0.txt=reshape({ 'PA10','PB16'},1,2);MCHP.module.I2S.pin.SCK0.Rx_idx=reshape([10 48],1,2);MCHP.module.I2S.pin.SCK0.ABCD=reshape([9 9],1,2);MCHP.module.I2S.pin.SCK1.txt=reshape({ 'PB28','PB12'},1,2);MCHP.module.I2S.pin.SCK1.Rx_idx=reshape([60 44],1,2);MCHP.module.I2S.pin.SCK1.ABCD=reshape([9 9],1,2);MCHP.module.I2S.pin.SDI.txt=reshape({ 'PA22','PB10'},1,2);MCHP.module.I2S.pin.SDI.Rx_idx=reshape([22 42],1,2);MCHP.module.I2S.pin.SDI.ABCD=reshape([9 9],1,2);MCHP.module.I2S.pin.SDO.txt=reshape({ 'PA11','PA21'},1,2);MCHP.module.I2S.pin.SDO.Rx_idx=reshape([11 21],1,2);MCHP.module.I2S.pin.SDO.ABCD=reshape([9 9],1,2);MCHP.module.PCC.PID=129;MCHP.module.PCC.vector='PCC';MCHP.module.PCC.pin.CLK.txt={ 'PA14'};MCHP.module.PCC.pin.CLK.Rx_idx=14;MCHP.module.PCC.pin.CLK.ABCD=10;MCHP.module.PCC.pin.DATA0.txt={ 'PA16'};MCHP.module.PCC.pin.DATA0.Rx_idx=16;MCHP.module.PCC.pin.DATA0.ABCD=10;MCHP.module.PCC.pin.DATA1.txt={ 'PA17'};MCHP.module.PCC.pin.DATA1.Rx_idx=17;MCHP.module.PCC.pin.DATA1.ABCD=10;MCHP.module.PCC.pin.DATA2.txt={ 'PA18'};MCHP.module.PCC.pin.DATA2.Rx_idx=18;MCHP.module.PCC.pin.DATA2.ABCD=10;MCHP.module.PCC.pin.DATA3.txt={ 'PA19'};MCHP.module.PCC.pin.DATA3.Rx_idx=19;MCHP.module.PCC.pin.DATA3.ABCD=10;MCHP.module.PCC.pin.DATA4.txt={ 'PA20'};MCHP.module.PCC.pin.DATA4.Rx_idx=20;MCHP.module.PCC.pin.DATA4.ABCD=10;MCHP.module.PCC.pin.DATA5.txt={ 'PA21'};MCHP.module.PCC.pin.DATA5.Rx_idx=21;MCHP.module.PCC.pin.DATA5.ABCD=10;MCHP.module.PCC.pin.DATA6.txt={ 'PA22'};MCHP.module.PCC.pin.DATA6.Rx_idx=22;MCHP.module.PCC.pin.DATA6.ABCD=10;MCHP.module.PCC.pin.DATA7.txt={ 'PA23'};MCHP.module.PCC.pin.DATA7.Rx_idx=23;MCHP.module.PCC.pin.DATA7.ABCD=10;MCHP.module.PCC.pin.DATA8.txt={ 'PB14'};MCHP.module.PCC.pin.DATA8.Rx_idx=46;MCHP.module.PCC.pin.DATA8.ABCD=10;MCHP.module.PCC.pin.DATA9.txt={ 'PB15'};MCHP.module.PCC.pin.DATA9.Rx_idx=47;MCHP.module.PCC.pin.DATA9.ABCD=10;MCHP.module.PCC.pin.DATA10.txt={ 'PC12'};MCHP.module.PCC.pin.DATA10.Rx_idx=76;MCHP.module.PCC.pin.DATA10.ABCD=10;MCHP.module.PCC.pin.DATA11.txt={ 'PC13'};MCHP.module.PCC.pin.DATA11.Rx_idx=77;MCHP.module.PCC.pin.DATA11.ABCD=10;MCHP.module.PCC.pin.DATA12.txt={ 'PC14'};MCHP.module.PCC.pin.DATA12.Rx_idx=78;MCHP.module.PCC.pin.DATA12.ABCD=10;MCHP.module.PCC.pin.DATA13.txt={ 'PC15'};MCHP.module.PCC.pin.DATA13.Rx_idx=79;MCHP.module.PCC.pin.DATA13.ABCD=10;MCHP.module.PCC.pin.DEN1.txt={ 'PA12'};MCHP.module.PCC.pin.DEN1.Rx_idx=12;MCHP.module.PCC.pin.DEN1.ABCD=10;MCHP.module.PCC.pin.DEN2.txt={ 'PA13'};MCHP.module.PCC.pin.DEN2.Rx_idx=13;MCHP.module.PCC.pin.DEN2.ABCD=10;MCHP.module.AES.PID=130;MCHP.module.AES.vector='AES';MCHP.module.TRNG.PID=131;MCHP.module.TRNG.vector='TRNG';MCHP.module.ICM.PID=132;MCHP.module.ICM.vector='ICM';MCHP.module.PUKCC.PID=133;MCHP.module.PUKCC.vector='PUKCC';MCHP.module.QSPI.PID=134;MCHP.module.QSPI.vector='QSPI';MCHP.module.QSPI.pin.CS.txt={ 'PB11'};MCHP.module.QSPI.pin.CS.Rx_idx=43;MCHP.module.QSPI.pin.CS.ABCD=7;MCHP.module.QSPI.pin.DATA0.txt={ 'PA08'};MCHP.module.QSPI.pin.DATA0.Rx_idx=8;MCHP.module.QSPI.pin.DATA0.ABCD=7;MCHP.module.QSPI.pin.DATA1.txt={ 'PA09'};MCHP.module.QSPI.pin.DATA1.Rx_idx=9;MCHP.module.QSPI.pin.DATA1.ABCD=7;MCHP.module.QSPI.pin.DATA2.txt={ 'PA10'};MCHP.module.QSPI.pin.DATA2.Rx_idx=10;MCHP.module.QSPI.pin.DATA2.ABCD=7;MCHP.module.QSPI.pin.DATA3.txt={ 'PA11'};MCHP.module.QSPI.pin.DATA3.Rx_idx=11;MCHP.module.QSPI.pin.DATA3.ABCD=7;MCHP.module.QSPI.pin.SCK.txt={ 'PB10'};MCHP.module.QSPI.pin.SCK.Rx_idx=42;MCHP.module.QSPI.pin.SCK.ABCD=7;MCHP.module.SDHC0.PID=135;MCHP.module.SDHC0.vector='SDHC0';MCHP.module.SDHC0.pin.SDCD.txt=reshape({ 'PA06','PA12','PB12','PC06'},1,4);MCHP.module.SDHC0.pin.SDCD.Rx_idx=reshape([6 12 44 70],1,4);MCHP.module.SDHC0.pin.SDCD.ABCD=reshape([8 8 8 8],1,4);MCHP.module.SDHC0.pin.SDCK.txt={ 'PB11'};MCHP.module.SDHC0.pin.SDCK.Rx_idx=43;MCHP.module.SDHC0.pin.SDCK.ABCD=8;MCHP.module.SDHC0.pin.SDCMD.txt={ 'PA08'};MCHP.module.SDHC0.pin.SDCMD.Rx_idx=8;MCHP.module.SDHC0.pin.SDCMD.ABCD=8;MCHP.module.SDHC0.pin.SDDAT0.txt={ 'PA09'};MCHP.module.SDHC0.pin.SDDAT0.Rx_idx=9;MCHP.module.SDHC0.pin.SDDAT0.ABCD=8;MCHP.module.SDHC0.pin.SDDAT1.txt={ 'PA10'};MCHP.module.SDHC0.pin.SDDAT1.Rx_idx=10;MCHP.module.SDHC0.pin.SDDAT1.ABCD=8;MCHP.module.SDHC0.pin.SDDAT2.txt={ 'PA11'};MCHP.module.SDHC0.pin.SDDAT2.Rx_idx=11;MCHP.module.SDHC0.pin.SDDAT2.ABCD=8;MCHP.module.SDHC0.pin.SDDAT3.txt={ 'PB10'};MCHP.module.SDHC0.pin.SDDAT3.Rx_idx=42;MCHP.module.SDHC0.pin.SDDAT3.ABCD=8;MCHP.module.SDHC0.pin.SDWP.txt=reshape({ 'PA07','PA13','PB13','PC07'},1,4);MCHP.module.SDHC0.pin.SDWP.Rx_idx=reshape([7 13 45 71],1,4);MCHP.module.SDHC0.pin.SDWP.ABCD=reshape([8 8 8 8],1,4);MCHP.module.SDHC1.PID=136;MCHP.module.SDHC1.vector='SDHC1';MCHP.module.SDHC1.pin.SDCD.txt=reshape({ 'PB16','PC20','PD20'},1,3);MCHP.module.SDHC1.pin.SDCD.Rx_idx=reshape([48 84 116],1,3);MCHP.module.SDHC1.pin.SDCD.ABCD=reshape([8 8 8],1,3);MCHP.module.SDHC1.pin.SDCK.txt={ 'PA21'};MCHP.module.SDHC1.pin.SDCK.Rx_idx=21;MCHP.module.SDHC1.pin.SDCK.ABCD=8;MCHP.module.SDHC1.pin.SDCMD.txt={ 'PA20'};MCHP.module.SDHC1.pin.SDCMD.Rx_idx=20;MCHP.module.SDHC1.pin.SDCMD.ABCD=8;MCHP.module.SDHC1.pin.SDDAT0.txt={ 'PB18'};MCHP.module.SDHC1.pin.SDDAT0.Rx_idx=50;MCHP.module.SDHC1.pin.SDDAT0.ABCD=8;MCHP.module.SDHC1.pin.SDDAT1.txt={ 'PB19'};MCHP.module.SDHC1.pin.SDDAT1.Rx_idx=51;MCHP.module.SDHC1.pin.SDDAT1.ABCD=8;MCHP.module.SDHC1.pin.SDDAT2.txt={ 'PB20'};MCHP.module.SDHC1.pin.SDDAT2.Rx_idx=52;MCHP.module.SDHC1.pin.SDDAT2.ABCD=8;MCHP.module.SDHC1.pin.SDDAT3.txt={ 'PB21'};MCHP.module.SDHC1.pin.SDDAT3.Rx_idx=53;MCHP.module.SDHC1.pin.SDDAT3.ABCD=8;MCHP.module.SDHC1.pin.SDWP.txt=reshape({ 'PB17','PC21','PD21'},1,3);MCHP.module.SDHC1.pin.SDWP.Rx_idx=reshape([49 85 117],1,3);MCHP.module.SDHC1.pin.SDWP.ABCD=reshape([8 8 8],1,3);MCHP.module.CCL.pin.IN0.txt=reshape({ 'PA04','PA16','PB22'},1,3);MCHP.module.CCL.pin.IN0.Rx_idx=reshape([4 16 54],1,3);MCHP.module.CCL.pin.IN0.ABCD=reshape([13 13 13],1,3);MCHP.module.CCL.pin.IN1.txt=reshape({ 'PA05','PA17','PB00'},1,3);MCHP.module.CCL.pin.IN1.Rx_idx=reshape([5 17 32],1,3);MCHP.module.CCL.pin.IN1.ABCD=reshape([13 13 13],1,3);MCHP.module.CCL.pin.IN2.txt=reshape({ 'PA06','PA18','PB01'},1,3);MCHP.module.CCL.pin.IN2.Rx_idx=reshape([6 18 33],1,3);MCHP.module.CCL.pin.IN2.ABCD=reshape([13 13 13],1,3);MCHP.module.CCL.pin.IN3.txt=reshape({ 'PA08','PA30'},1,2);MCHP.module.CCL.pin.IN3.Rx_idx=reshape([8 30],1,2);MCHP.module.CCL.pin.IN3.ABCD=reshape([13 13],1,2);MCHP.module.CCL.pin.IN4.txt=reshape({ 'PA09','PC27'},1,2);MCHP.module.CCL.pin.IN4.Rx_idx=reshape([9 91],1,2);MCHP.module.CCL.pin.IN4.ABCD=reshape([13 13],1,2);MCHP.module.CCL.pin.IN5.txt=reshape({ 'PA10','PC28'},1,2);MCHP.module.CCL.pin.IN5.Rx_idx=reshape([10 92],1,2);MCHP.module.CCL.pin.IN5.ABCD=reshape([13 13],1,2);MCHP.module.CCL.pin.IN6.txt=reshape({ 'PA22','PB06'},1,2);MCHP.module.CCL.pin.IN6.Rx_idx=reshape([22 38],1,2);MCHP.module.CCL.pin.IN6.ABCD=reshape([13 13],1,2);MCHP.module.CCL.pin.IN7.txt=reshape({ 'PA23','PB07'},1,2);MCHP.module.CCL.pin.IN7.Rx_idx=reshape([23 39],1,2);MCHP.module.CCL.pin.IN7.ABCD=reshape([13 13],1,2);MCHP.module.CCL.pin.IN8.txt=reshape({ 'PA24','PB08'},1,2);MCHP.module.CCL.pin.IN8.Rx_idx=reshape([24 40],1,2);MCHP.module.CCL.pin.IN8.ABCD=reshape([13 13],1,2);MCHP.module.CCL.pin.IN9.txt=reshape({ 'PB14','PC20'},1,2);MCHP.module.CCL.pin.IN9.Rx_idx=reshape([46 84],1,2);MCHP.module.CCL.pin.IN9.ABCD=reshape([13 13],1,2);MCHP.module.CCL.pin.IN10.txt=reshape({ 'PB15','PC21'},1,2);MCHP.module.CCL.pin.IN10.Rx_idx=reshape([47 85],1,2);MCHP.module.CCL.pin.IN10.ABCD=reshape([13 13],1,2);MCHP.module.CCL.pin.IN11.txt=reshape({ 'PB10','PB16'},1,2);MCHP.module.CCL.pin.IN11.Rx_idx=reshape([42 48],1,2);MCHP.module.CCL.pin.IN11.ABCD=reshape([13 13],1,2);MCHP.module.CCL.pin.OUT0.txt=reshape({ 'PA07','PA19','PB02','PB23'},1,4);MCHP.module.CCL.pin.OUT0.Rx_idx=reshape([7 19 34 55],1,4);MCHP.module.CCL.pin.OUT0.ABCD=reshape([13 13 13 13],1,4);MCHP.module.CCL.pin.OUT1.txt=reshape({ 'PA11','PA31','PB11'},1,3);MCHP.module.CCL.pin.OUT1.Rx_idx=reshape([11 31 43],1,3);MCHP.module.CCL.pin.OUT1.ABCD=reshape([13 13 13],1,3);MCHP.module.CCL.pin.OUT2.txt=reshape({ 'PA25','PB09'},1,2);MCHP.module.CCL.pin.OUT2.Rx_idx=reshape([25 41],1,2);MCHP.module.CCL.pin.OUT2.ABCD=reshape([13 13],1,2);MCHP.module.CCL.pin.OUT3.txt={ 'PB17'};MCHP.module.CCL.pin.OUT3.Rx_idx=49;MCHP.module.CCL.pin.OUT3.ABCD=13;MCHP.module.GCLK.pin.IO0.txt=reshape({ 'PA30','PB14','PA14','PB22'},1,4);MCHP.module.GCLK.pin.IO0.Rx_idx=reshape([30 46 14 54],1,4);MCHP.module.GCLK.pin.IO0.ABCD=reshape([12 12 12 12],1,4);MCHP.module.GCLK.pin.IO1.txt=reshape({ 'PB15','PA15','PB23','PA27'},1,4);MCHP.module.GCLK.pin.IO1.Rx_idx=reshape([47 15 55 27],1,4);MCHP.module.GCLK.pin.IO1.ABCD=reshape([12 12 12 12],1,4);MCHP.module.GCLK.pin.IO2.txt=reshape({ 'PA16','PB16'},1,2);MCHP.module.GCLK.pin.IO2.Rx_idx=reshape([16 48],1,2);MCHP.module.GCLK.pin.IO2.ABCD=reshape([12 12],1,2);MCHP.module.GCLK.pin.IO3.txt=reshape({ 'PA17','PB17'},1,2);MCHP.module.GCLK.pin.IO3.Rx_idx=reshape([17 49],1,2);MCHP.module.GCLK.pin.IO3.ABCD=reshape([12 12],1,2);MCHP.module.GCLK.pin.IO4.txt=reshape({ 'PA10','PB10','PB18'},1,3);MCHP.module.GCLK.pin.IO4.Rx_idx=reshape([10 42 50],1,3);MCHP.module.GCLK.pin.IO4.ABCD=reshape([12 12 12],1,3);MCHP.module.GCLK.pin.IO5.txt=reshape({ 'PA11','PB11','PB19'},1,3);MCHP.module.GCLK.pin.IO5.Rx_idx=reshape([11 43 51],1,3);MCHP.module.GCLK.pin.IO5.ABCD=reshape([12 12 12],1,3);MCHP.module.GCLK.pin.IO6.txt=reshape({ 'PB12','PB20'},1,2);MCHP.module.GCLK.pin.IO6.Rx_idx=reshape([44 52],1,2);MCHP.module.GCLK.pin.IO6.ABCD=reshape([12 12],1,2);MCHP.module.GCLK.pin.IO7.txt=reshape({ 'PB13','PB21'},1,2);MCHP.module.GCLK.pin.IO7.Rx_idx=reshape([45 53],1,2);MCHP.module.GCLK.pin.IO7.ABCD=reshape([12 12],1,2);MCHP.module.TPIU.pin.TRACECLK.txt={ 'PC27'};MCHP.module.TPIU.pin.TRACECLK.Rx_idx=91;MCHP.module.TPIU.pin.TRACECLK.ABCD=7;MCHP.module.TPIU.pin.TRACED0.txt={ 'PC28'};MCHP.module.TPIU.pin.TRACED0.Rx_idx=92;MCHP.module.TPIU.pin.TRACED0.ABCD=7;MCHP.module.TPIU.pin.TRACED1.txt={ 'PC26'};MCHP.module.TPIU.pin.TRACED1.Rx_idx=90;MCHP.module.TPIU.pin.TRACED1.ABCD=7;MCHP.module.TPIU.pin.TRACED2.txt={ 'PC25'};MCHP.module.TPIU.pin.TRACED2.Rx_idx=89;MCHP.module.TPIU.pin.TRACED2.ABCD=7;MCHP.module.TPIU.pin.TRACED3.txt={ 'PC24'};MCHP.module.TPIU.pin.TRACED3.Rx_idx=88;MCHP.module.TPIU.pin.TRACED3.ABCD=7;MCHP.module.FUSES.reglist=reshape({ 'USER_WORD_0','USER_WORD_1','USER_WORD_2'},1,3);MCHP.module.FUSES.reg.USER_WORD_0.caption='USER Page Word 0';MCHP.module.FUSES.reg.USER_WORD_0.bitfieldList=reshape({ 'BOD33_DIS','BOD33USERLEVEL','BOD33_ACTION','BOD33_HYST','NVMCTRL_BOOTPROT'},1,5);MCHP.module.FUSES.reg.USER_WORD_0.BOD33_DIS.mask=2;MCHP.module.FUSES.reg.USER_WORD_0.BOD33_DIS.choice=reshape({ 'CLEAR','SET'},1,2);MCHP.module.FUSES.reg.USER_WORD_0.BOD33_DIS.choiceCaption=reshape({ 'clear','set'},1,2);MCHP.module.FUSES.reg.USER_WORD_0.BOD33_DIS.choiceDefault='SET';MCHP.module.FUSES.reg.USER_WORD_0.BOD33USERLEVEL.mask=256;MCHP.module.FUSES.reg.USER_WORD_0.BOD33USERLEVEL.choice={};MCHP.module.FUSES.reg.USER_WORD_0.BOD33USERLEVEL.choiceCaption={ 'range in [0 - 255]'};MCHP.module.FUSES.reg.USER_WORD_0.BOD33USERLEVEL.choiceDefault='0xFF';MCHP.module.FUSES.reg.USER_WORD_0.BOD33_ACTION.mask=4;MCHP.module.FUSES.reg.USER_WORD_0.BOD33_ACTION.choice=reshape({ 'NONE','RESET','INT','BKUP'},1,4);MCHP.module.FUSES.reg.USER_WORD_0.BOD33_ACTION.choiceCaption=reshape({ 'No action','The BOD33 generates a reset','The BOD33 generates an interrupt','The BOD33 puts the device in backup sleep mode'},1,4);MCHP.module.FUSES.reg.USER_WORD_0.BOD33_ACTION.choiceDefault='NONE';MCHP.module.FUSES.reg.USER_WORD_0.BOD33_HYST.mask=16;MCHP.module.FUSES.reg.USER_WORD_0.BOD33_HYST.choice=reshape({ '0','1','2','3','4','5','6','7','8','9','A','B','C','D','E','F','10'},1,17);MCHP.module.FUSES.reg.USER_WORD_0.BOD33_HYST.choiceCaption=reshape({ '0','1','2','3','4','5','6','7','8','9','A','B','C','D','E','F','10'},1,17);MCHP.module.FUSES.reg.USER_WORD_0.BOD33_HYST.choiceDefault='0xF';MCHP.module.FUSES.reg.USER_WORD_0.NVMCTRL_BOOTPROT.mask=16;MCHP.module.FUSES.reg.USER_WORD_0.NVMCTRL_BOOTPROT.choice=reshape({ '0','8','16','24','32','40','48','56','64','72','80','88','96','104','112','120'},1,16);MCHP.module.FUSES.reg.USER_WORD_0.NVMCTRL_BOOTPROT.choiceCaption=reshape({ '0 kbytes','8 kbytes','16 kbytes','24 kbytes','32 kbytes','40 kbytes','48 kbytes','56 kbytes','64 kbytes','72 kbytes','80 kbytes','88 kbytes','96 kbytes','104 kbytes','112 kbytes','120 kbytes'},1,16);MCHP.module.FUSES.reg.USER_WORD_0.NVMCTRL_BOOTPROT.choiceDefault='0';MCHP.module.FUSES.reg.USER_WORD_1.caption='USER Page Word 1';MCHP.module.FUSES.reg.USER_WORD_1.bitfieldList=reshape({ 'NVMCTRL_SEESBLK','NVMCTRL_SEEPSZ','RAMECC_ECCDIS','WDT_ENABLE','WDT_ALWAYSON','WDT_PER','WDT_WINDOW','WDT_EWOFFSET','WDT_WEN'},1,9);MCHP.module.FUSES.reg.USER_WORD_1.NVMCTRL_SEESBLK.mask=16;MCHP.module.FUSES.reg.USER_WORD_1.NVMCTRL_SEESBLK.choice=reshape({ '0','1','2','3','4','5','6','7','8','9','A','B','C','D','E','F','10'},1,17);MCHP.module.FUSES.reg.USER_WORD_1.NVMCTRL_SEESBLK.choiceCaption=reshape({ '0','1','2','3','4','5','6','7','8','9','A','B','C','D','E','F','10'},1,17);MCHP.module.FUSES.reg.USER_WORD_1.NVMCTRL_SEESBLK.choiceDefault='0xF';MCHP.module.FUSES.reg.USER_WORD_1.NVMCTRL_SEEPSZ.mask=8;MCHP.module.FUSES.reg.USER_WORD_1.NVMCTRL_SEEPSZ.choice=reshape({ '0','1','2','3','4','5','6','7','8'},1,9);MCHP.module.FUSES.reg.USER_WORD_1.NVMCTRL_SEEPSZ.choiceCaption=reshape({ '0','1','2','3','4','5','6','7','8'},1,9);MCHP.module.FUSES.reg.USER_WORD_1.NVMCTRL_SEEPSZ.choiceDefault='0x7';MCHP.module.FUSES.reg.USER_WORD_1.RAMECC_ECCDIS.mask=2;MCHP.module.FUSES.reg.USER_WORD_1.RAMECC_ECCDIS.choice=reshape({ 'CLEAR','SET'},1,2);MCHP.module.FUSES.reg.USER_WORD_1.RAMECC_ECCDIS.choiceCaption=reshape({ 'clear','set'},1,2);MCHP.module.FUSES.reg.USER_WORD_1.RAMECC_ECCDIS.choiceDefault='SET';MCHP.module.FUSES.reg.USER_WORD_1.WDT_ENABLE.mask=2;MCHP.module.FUSES.reg.USER_WORD_1.WDT_ENABLE.choice=reshape({ 'CLEAR','SET'},1,2);MCHP.module.FUSES.reg.USER_WORD_1.WDT_ENABLE.choiceCaption=reshape({ 'clear','set'},1,2);MCHP.module.FUSES.reg.USER_WORD_1.WDT_ENABLE.choiceDefault='CLEAR';MCHP.module.FUSES.reg.USER_WORD_1.WDT_ALWAYSON.mask=2;MCHP.module.FUSES.reg.USER_WORD_1.WDT_ALWAYSON.choice=reshape({ 'CLEAR','SET'},1,2);MCHP.module.FUSES.reg.USER_WORD_1.WDT_ALWAYSON.choiceCaption=reshape({ 'clear','set'},1,2);MCHP.module.FUSES.reg.USER_WORD_1.WDT_ALWAYSON.choiceDefault='CLEAR';MCHP.module.FUSES.reg.USER_WORD_1.WDT_PER.mask=16;MCHP.module.FUSES.reg.USER_WORD_1.WDT_PER.choice=reshape({ 'CYC8','CYC16','CYC32','CYC64','CYC128','CYC256','CYC512','CYC1024','CYC2048','CYC4096','CYC8192','CYC16384'},1,12);MCHP.module.FUSES.reg.USER_WORD_1.WDT_PER.choiceCaption=reshape({ '8 clock cycles','16 clock cycles','32 clock cycles','64 clock cycles','128 clock cycles','256 clock cycles','512 clock cycles','1024 clock cycles','2048 clock cycles','4096 clock cycles','8192 clock cycles','16384 clock cycles'},1,12);MCHP.module.FUSES.reg.USER_WORD_1.WDT_PER.choiceDefault='CYC16384';MCHP.module.FUSES.reg.USER_WORD_1.WDT_WINDOW.mask=16;MCHP.module.FUSES.reg.USER_WORD_1.WDT_WINDOW.choice=reshape({ 'CYC8','CYC16','CYC32','CYC64','CYC128','CYC256','CYC512','CYC1024','CYC2048','CYC4096','CYC8192','CYC16384'},1,12);MCHP.module.FUSES.reg.USER_WORD_1.WDT_WINDOW.choiceCaption=reshape({ '8 clock cycles','16 clock cycles','32 clock cycles','64 clock cycles','128 clock cycles','256 clock cycles','512 clock cycles','1024 clock cycles','2048 clock cycles','4096 clock cycles','8192 clock cycles','16384 clock cycles'},1,12);MCHP.module.FUSES.reg.USER_WORD_1.WDT_WINDOW.choiceDefault='CYC16384';MCHP.module.FUSES.reg.USER_WORD_1.WDT_EWOFFSET.mask=16;MCHP.module.FUSES.reg.USER_WORD_1.WDT_EWOFFSET.choice=reshape({ 'CYC8','CYC16','CYC32','CYC64','CYC128','CYC256','CYC512','CYC1024','CYC2048','CYC4096','CYC8192','CYC16384'},1,12);MCHP.module.FUSES.reg.USER_WORD_1.WDT_EWOFFSET.choiceCaption=reshape({ '8 clock cycles','16 clock cycles','32 clock cycles','64 clock cycles','128 clock cycles','256 clock cycles','512 clock cycles','1024 clock cycles','2048 clock cycles','4096 clock cycles','8192 clock cycles','16384 clock cycles'},1,12);MCHP.module.FUSES.reg.USER_WORD_1.WDT_EWOFFSET.choiceDefault='CYC16384';MCHP.module.FUSES.reg.USER_WORD_1.WDT_WEN.mask=2;MCHP.module.FUSES.reg.USER_WORD_1.WDT_WEN.choice=reshape({ 'CLEAR','SET'},1,2);MCHP.module.FUSES.reg.USER_WORD_1.WDT_WEN.choiceCaption=reshape({ 'clear','set'},1,2);MCHP.module.FUSES.reg.USER_WORD_1.WDT_WEN.choiceDefault='CLEAR';MCHP.module.FUSES.reg.USER_WORD_2.caption='USER Page Word 2';MCHP.module.FUSES.reg.USER_WORD_2.bitfieldList={ 'NVMCTRL_REGION_LOCKS'};MCHP.module.FUSES.reg.USER_WORD_2.NVMCTRL_REGION_LOCKS.mask=MCHP_Fun.Hex2num('41F0000000000000');MCHP.module.FUSES.reg.USER_WORD_2.NVMCTRL_REGION_LOCKS.choice={};MCHP.module.FUSES.reg.USER_WORD_2.NVMCTRL_REGION_LOCKS.choiceCaption={ 'range in [0 - 4294967295]'};MCHP.module.FUSES.reg.USER_WORD_2.NVMCTRL_REGION_LOCKS.choiceDefault='0xFFFFFFFF';MCHP.PortBase=32;MCHP.PortPrefixe='P';MCHP.PowerSave=0;MCHP.fcy.GCLKx=reshape([1e+08 -1 -1 -1 -1 -1 -1 -1 -1 -1 -1 -1],1,12);MCHP.fcy.MIPS=1e+08;MCHP.fcy.APB_HS=1e+08;MCHP.fcy.APB_CPU=1e+08;MCHP.fcy.AHB_CPU=1e+08;MCHP.NTIMERS=0;MCHP.SCCP.nSCCP=0;MCHP.SYS_TICK_TS_Load=99999;MCHP.TimeStepFactor=1;MCHP.INT_PRIORITY_DMA='0';, MCHP_CRC=28109702, BTMODE=Not used, RES1=Not used, PLLSS=Not used, RES2=Not used, ALTCMPI=Not used, BOREN1=Not used, ALTRB6=Not used, RETCFG=Not used, DFMCY=Not used, BSS2=No Boot Segment, BSEN=No Boot Segment, CWRP=Configuration Segment may be written, CSS=No Protection (other than CWRP), AIVTDIS=Disabled AIVT, BSLIM=Not used, WDTEN=Disable, BTSWP=BOOTSWP instruction is disabled, DBCC=No Cross Connection between DAC outputs, CTXT1=Not Assigned, CTXT2=Not Assigned, SEQNUM=Not used, nSEQNUM=Not used, BOREN0=Enabled, DMTIVT=Not used, DMTCNT=2^31 (2147483648), DMTEN=Dead Man Timer is Disabled and can be enabled by software, ON=Not used, USERID=Not used, RESERVED1=Not used, PGL1WAY=Allow only one reconfiguration, FPLLRNG=34-68 MHz Input, FPLLICLK=FRC is input to the System PLL, FPLLMULT=PLL Multiply by 128, UPLLFSEL=USB PLL input is 24 MHz, DMTINTV=Window/Interval value is 127/128 counter value, WDTSPGM=WDT stops during Flash programming, FDMTEN=Deadman Timer is disabled, TRCEN=Trace features in the CPU are enabled, BOOTISA=Boot code and Exception code is MIPS32, FECCCON=ECC and Dynamic ECC are disabled (ECCCON bits are writable), EXTDDRSIZE=Not used, FSLEEP=Flash is powered down when the device is in Sleep mode, DBGPER=Allow CPU access to all permission regions, EJTAGBEN=Normal EJTAG functionality, TSEQ=Not used, CSEQ=Not used, RWDTPS=1:1048576, RCLKSEL=Always use LPRC, SWDTPS=1:1048576, DMTIVTL=Not used, DMTIVTH=Not used, DMTCNTL=Not used, DMTCNTH=Not used, DMTDIS=Dead Man Timer is Disabled and can be enabled by software, SMBEN=SMBus input threshold is enabled, SPI2PIN=SPI2 uses I/O remap (PPS) pins, CTXT3=Not Assigned, CTXT4=Not Assigned, MBXM0=Mailbox register configured for Master data read (Slave to Master data transfer), MBXM1=Mailbox register configured for Master data read (Slave to Master data transfer), MBXM2=Mailbox register configured for Master data read (Slave to Master data transfer), MBXM3=Mailbox register configured for Master data read (Slave to Master data transfer), MBXM4=Mailbox register configured for Master data read (Slave to Master data transfer), MBXM5=Mailbox register configured for Master data read (Slave to Master data transfer), MBXM6=Mailbox register configured for Master data read (Slave to Master data transfer), MBXM7=Mailbox register configured for Master data read (Slave to Master data transfer), MBXM8=Mailbox register configured for Master data read (Slave to Master data transfer), MBXM9=Mailbox register configured for Master data read (Slave to Master data transfer), MBXM10=Mailbox register configured for Master data read (Slave to Master data transfer), MBXM11=Mailbox register configured for Master data read (Slave to Master data transfer), MBXM12=Mailbox register configured for Master data read (Slave to Master data transfer), MBXM13=Mailbox register configured for Master data read (Slave to Master data transfer), MBXM14=Mailbox register configured for Master data read (Slave to Master data transfer), MBXM15=Mailbox register configured for Master data read (Slave to Master data transfer), MBXHSA=MSIxMBXD15 assigned to mailbox handshake protocol block A, MBXHSB=MSIxMBXD15 assigned to mailbox handshake protocol block B, MBXHSC=MSIxMBXD15 assigned to mailbox handshake protocol block C, MBXHSD=MSIxMBXD15 assigned to mailbox handshake protocol block D, MBXHSE=MSIxMBXD15 assigned to mailbox handshake protocol block E, MBXHSF=MSIxMBXD15 assigned to mailbox handshake protocol block F, MBXHSG=MSIxMBXD15 assigned to mailbox handshake protocol block G, MBXHSH=MSIxMBXD15 assigned to mailbox handshake protocol block H, HSAEN=Mailbox data flow control handshake protocol block disabled., HSBEN=Mailbox data flow control handshake protocol block disabled., HSCEN=Mailbox data flow control handshake protocol block disabled., HSDEN=Mailbox data flow control handshake protocol block disabled., HSEEN=Mailbox data flow control handshake protocol block disabled., HSFEN=Mailbox data flow control handshake protocol block disabled., HSGEN=Mailbox data flow control handshake protocol block disabled., HSHEN=Mailbox data flow control handshake protocol block disabled., CPRA0=Master core owns pin., CPRA1=Master core owns pin., CPRA2=Master core owns pin., CPRA3=Master core owns pin., CPRA4=Master core owns pin., CPRB0=Master core owns pin., CPRB1=Master core owns pin., CPRB2=Master core owns pin., CPRB3=Master core owns pin., CPRB4=Master core owns pin., CPRB5=Master core owns pin., CPRB6=Master core owns pin., CPRB7=Master core owns pin., CPRB8=Master core owns pin., CPRB9=Master core owns pin., CPRB10=Master core owns pin., CPRB11=Master core owns pin., CPRB12=Master core owns pin., CPRB13=Master core owns pin., CPRB14=Master core owns pin., CPRB15=Master core owns pin., CPRC0=Master core owns pin., CPRC1=Master core owns pin., CPRC2=Master core owns pin., CPRC3=Master core owns pin., CPRC4=Master core owns pin., CPRC5=Master core owns pin., CPRC6=Master core owns pin., CPRC7=Master core owns pin., CPRC8=Master core owns pin., CPRC9=Master core owns pin., CPRC10=Master core owns pin., CPRC11=Master core owns pin., CPRC12=Master core owns pin., CPRC13=Master core owns pin., CPRC14=Master core owns pin., CPRC15=Master core owns pin., CPRD0=Master core owns pin., CPRD1=Master core owns pin., CPRD2=Master core owns pin., CPRD3=Master core owns pin., CPRD4=Master core owns pin., CPRD5=Master core owns pin., CPRD6=Master core owns pin., CPRD7=Master core owns pin., CPRD8=Master core owns pin., CPRD9=Master core owns pin., CPRD10=Master core owns pin., CPRD11=Master core owns pin., CPRD12=Master core owns pin., CPRD13=Master core owns pin., CPRD14=Master core owns pin., CPRD15=Master core owns pin., CPRE0=Master core owns pin., CPRE1=Master core owns pin., CPRE2=Master core owns pin., CPRE3=Master core owns pin., CPRE4=Master core owns pin., CPRE5=Master core owns pin., CPRE6=Master core owns pin., CPRE7=Master core owns pin., CPRE8=Master core owns pin., CPRE9=Master core owns pin., CPRE10=Master core owns pin., CPRE11=Master core owns pin., CPRE12=Master core owns pin., CPRE13=Master core owns pin., CPRE14=Master core owns pin., CPRE15=Master core owns pin., S1FNOSC=Internal Fast RC (FRC) Oscillator with postscaler, S1IESO=Start up with FRC; then switch, S1OSCIOFNC=OSC2 is clock output, S1FCKSM=Both Clock switching and Fail-safe Clock Monitor are disabled, S1PLLKEN=S1PLLKEN_ON, S1RWDTPS=1:1048576, S1RCLKSEL=Always use LPRC, S1WINDIS=Watchdog Timer operates in Non-Window mode, S1WDTWIN=WDT Window is 25% of WDT period, S1SWDTPS=1:1048576, S1FWDTEN=Disable, S1ICS=Communicate on PGC1 and PGD1, S1DEBUG=Not used, S1ISOLAT=The slave can operate (in debug mode) even if the SLVEN bit in the MSI is zero., S1NOBTSWP=BOOTSWP instruction is disabled, S1ALTI2C1=I2C1 mapped to SDA1/SCL1 pins, S1SPI1PIN=Slave SPI1 uses I/O remap (PPS) pins, S1SSRE=Slave generated resets will reset the Slave Enable Bit in the MSI module, S1MSRE=The master software oriented RESET events (RESET Op-Code; Watchdog timeout; TRAP reset; illegalInstruction) will also cause the slave subsystem to reset., S1CTXT1=Not Assigned, S1CTXT2=Not Assigned, S1CTXT3=Not Assigned, S1CTXT4=Not Assigned, BORLVL=Not used, BSSO=Not used, MCA=Not used, MAXTEMP=Not used, CFGAN14=Not used, CFGAN15=Not used, S1IOL1WAY=Not used, S1BSSO=Not used, S1BACKBUG=Not used, BISTDIS=mBIST on reset feature disabled, NOBTSWP=BOOTSWP instruction is disabled, S1BISTDIS=Slave BIST on reset feature disabled, S1DMTIVTL=Not used, S1DMTIVTH=Not used, S1DMTCNTL=Not used, S1DMTCNTH=Not used, S1DMTDIS=Slave Dead Man Timer is Disabled and can be enabled by software, BSEQ=Not used, IBSEQ=Not used, SMB3EN=SMBus 3.0 input levels, FUSBIDIO2=USBID pin is controlled by the USB2 module, FVBUSIO2=VBUSON pin is controlled by the USB2 module, FUSBIDIO1=USBID pin is controlled by the USB1 module, FVBUSIO1=VBUSON pin is controlled by the USB1 module, VBATBOREN=Enable ZPBOR during VBAT Mode, FDSEN=Enable DSEN bit in DSCON, BORSEL=BOR trip voltage 2.1v (Non-OPAMP deviced operation), POSCFGAIN=Gain is G3, POSCAGCDLY=Settling time = 25ms x AGCRNG, POSCAGCRNG=Range 1x, POSCAGC=Automatic Gain Control for Oscillator, FDBGWP=Not used}
      mask prompts: PICREF "Target"; TIMESTEP_REF "Time-Step synchronisation"; BUSYFLAG "Busy Flag Port"; BUSYFLAG_TXT "Busy Flag Port txt"; PWRTEN "Power-up Timer Enable"; BOREN "Brown-out Reset Enable"; BODENV "Brown Out Voltage"; BORV "Brown-out Reset Voltage"; FPWRT "Power-on Reset Timer Value"; DSBOREN "Deep Sleep Zero-Power BOR Enable"; DSLPBOR "Deep Sleep Zero-Power BOR Enable"; MCLRE "Master Clear Enable"; SMCLR "Soft Master Clear Enable"; PMDL1WAY "Peripheral Module Disable Configuration"; RSTPRI "Reset Target Vector Select"; TEMP "Temperature Protection Enable"; SOSCSRC "SOSC Source Type"; SOSCSEL "SOSC Power Selection Configuration"; IOL1WAY "Peripheral pin select configuration"; ALTVREF "Alternate VREF location Enable"; DISUVREG "Internal USB 3.3V Regulator Disable"; DSSWEN "DSEN Enable"; LPCFG "Low power regulator control"; RTCBAT "RTC Battery Operation Enable"; VBTBOR "VBAT BOR enable"; WUTSEL "Voltage Regulator Wake-up Time Select"; POWERSAVE "Power Save Mode (Idle)"; FNOSC "Oscillator Source Selection"; FPR "Primary Oscillator Mode"; FOSFPR "Oscillator"; FOS "Oscillator Source"; FRANGE "Frequency Range Select"; OSCILLATOR_SELECT "Oscillator Source"; QUARTZ "Crystal range in 8e6 - 48e6 (Hz)"; POSCGAIN "Primary Oscillator Gain"; POSCBOOST "Primary Oscillator Boost Kick Start"; SOSCGAIN "Secondary Oscillator Gain"; SOSCBOOST "Secondary Oscillator Boost Kick Start"; ACTIV_PLL "Activate clock multiplier/divider (PLL)"; MIPS_DESIRED "Targeted Clock frequency in [96  -  120] (MHz)"; FPLLMUL "PLL Multiplier"; FPLLIDIV "PLL Input Divider"; POSCFREQ "Primary Oscillator Frequency Range Configuration"; POSCMD "Primary Oscillator Mode"; POSCMOD "Primary Oscillator Configuration"; MIPS "Achieved Frequency (Hz) with PLLin =2e+06, PLLout =1e+08  (x50)"; ACLKCON "Auxilliary Clock for PWM & ADC"; ACLKCON_Info "Auxilliary Clock Infos:"; FPLLODIV "System PLL Output Clock Divider"; PLLKEN "PLL Lock Enable"; FCKSM "Clock Switching and Monitor"; FCKSMEN "Clock Switching and Monitor"; IESO "Two-speed Oscillator Start-Up"; DSWDTPS "Deep Sleep Watchdog Timer Postscale"; FWDTEN "Watchdog Timer Enable"; FWDTWINSZ "Watchdog Timer Window Size"; FWPSA "WDT Prescaler A"; FWPSA0 "WDT Prescaler"; FWPSB "WDT Prescaler B"; WDT "Watchdog Timer"; WDTPOST "Watchdog Timer Postscaler"; WDTPRE "Watchdog Timer Prescaler"; WDTPS "Watchdog Timer Postscaler"; WINDIS "Watchdog Timer Window"; WWDTEN "Watchdog Timer Window"; DSWDTEN "Deep Sleep Watchdog Timer"; DSWDTOSC "DSWDT Reference Clock Select"; FPBDIV "Peripheral Clock Divisor"; FSOSCEN "Secondary Oscillator Enable"; LPRCSEL "LPRC Oscillator Power and Accuracy"; OSCIOFCN "OSC2 Pin Function"; OSCIOFNC "OSC2 Pin Function"; PLL_96MHZ "96MHz PLL"; PLL96MHZ "96MHz PLL Disable"; PLLDIV "96 MHz PLL Prescaler Select"; WDTCLK "WDT Clock Source Select bits"; WDTCMX "WDT Clock Source Select bits"; WDTWIN "Watch Dog Timer Window Width"; XTCFG "Crystal Oscillator Drive Select depending on crystal value"; XTBST "Oscillator Kick-Start Programmability bit"; APL "Auxiliary Segment Code-protect"; APLK "Auxiliary Segment Key"; AWRP "Auxiliary Segment Write-protect"; BSS "Boot segment Protect"; BWP "Boot Flash Write Protect"; BWRP "Boot Segment Write Protect"; CP "Code Protect"; EBS "Boot Segment Data EEPROM Protection"; ESS "Secure Segment Data EEPROM Protection"; GCP "General Segment Code Protection"; GSS "General Segment Code Protection"; GSS0 "General Segment Code Protect"; GSSK "General Segment Key"; GWRP "General Code Segment Write Protect"; PWP "Program Flash Write Protect"; RBS "Boot Segment Data RAM Protection"; RSS "Secure Segment Data RAM Protection"; SSS "Secure Segment Program Flash Code Protection"; SWRP "Secure Segment Program Write Protect"; WPCFG "Configuration Word Code Page Protection Select"; WPDIS "Segment Write Protection Disable"; WPEND "Segment Write Protection End Page Select"; WPFP "Write Protection Flash Page Segment Boundary"; ICESEL "ICE/ICD Comm Channel Select"; ICS "ICD Communication Channel Select"; JTAGEN "JTAG Port Enable"; COE "Set Clip On Emulation Mode"; RES "Set Clip On Emulation"; DEBUG "Background Debugger Enable"; BACKBUG "Background Debug"; BKBUG "Background Debugger Enable"; ALTI2C "Alternate I2C  pins"; ALTI2C1 "Alternate I2C pins for I2C1"; ALTI2C2 "Alternate I2C pins for I2C2"; ALTI2C3 "Alternate I2C pins for I2C3"; ALTQIO "Enable Alternate QEI1 pin"; ALTSS1 "Enable Alternate SS1 pin"; CMPPOL0 "Comparator Hysteresis Polarity (even comp)"; CMPPOL1 "Comparator Hysteresis Polarity (odd comp)"; FCANIO "CAN I/O Pin Select"; FETHIO "Ethernet I/O Pin Select"; FMIIEN "Ethernet RMII/MII Enable"; FSRSSEL "SRS Select"; FUSBIDIO "USB USID Selection"; FVBUSONIO "USB VBUS ON Selection"; HPOL "Motor Control PWM High Side Polarity"; HYST0 "Even Comparator Hysteresis Select"; HYST1 "Odd Comparator Hysteresis Select"; I2C1SEL "Alternate I2C1 Pin Mapping"; LPOL "Motor Control PWM Low Side Polarity"; PWMPIN "Motor Control PWM Module Pin Mode"; RTCOSC "RTCC Reference Clock Select"; UPLLEN "USB PLL Enable"; UPLLIDIV "USB PLL Input Divider"; ALTPMP "Alternate PMP Pin Mapping"; I2C2SEL "Alternate I2C2"; ALTADREF "External 12-Bit A/D Reference Location"; ALTCVREF "External Comparator Reference Location"; PWMLOCK "PWM Lock Enable"; INT_PRIORITY_DMA "DMA Interrupt Priority"; MCHP_PLLRegisters "MCHP_PLLReg"; BTMODE "xxx"; RES1 "xxx"; PLLSS "PLL Secondary Selection Configuration bit"; ALTCMPI "Alternate Comparator Input bit"; BOREN1 "BOR Override bit"; ALTRB6 "Alternate RB6 pin function enable bit"; RETCFG "xxx"; DFMCY "Data Flash Memory Cycle Count"; BSS2 "Boot Segment Control bit"; BSEN "Boot Segment Control bit"; CWRP "Configuration Segment Write-Protect bit"; CSS "Configuration Segment Code-Protect Level bits"; AIVTDIS "Alternate Interrupt Vector Table bit"; BSLIM "Boot Segment Flash Page Address Limit bits"; WDTEN "Watchdog Timer Enable"; BTSWP "BOOTSWP Instruction Enable/Disable bit"; DBCC "DACx Output Cross Connection bit"; CTXT1 "Specifies Interrupt Priority Level (IPL) Associated to Alternate Working Register 1 bits"; CTXT2 "Specifies Interrupt Priority Level (IPL) Associated to Alternate Working Register 2 bits"; SEQNUM "Sequence Number to Determine the Active Panel in Dual Panel Mode bits"; nSEQNUM "xxx"; BOREN0 "xxx"; DMTIVT "xxx"; DMTCNT "Deadman Timer Count Selection"; DMTEN "Deadman Timer Count Selection"; ON "xxx"; USERID "xxx"; RESERVED1 "xxx"; PGL1WAY "Permission Group Lock One Way Configuration"; FPLLRNG "System PLL Input Range"; FPLLICLK "System PLL Input Clock Selection"; FPLLMULT "System PLL Multiplier"; UPLLFSEL "USB PLL Input Frequency Selection"; DMTINTV "DMT Count Window Interval"; WDTSPGM "Watchdog Timer Stop During Flash Programming"; FDMTEN "Deadman Timer Enable"; TRCEN "Trace Enable"; BOOTISA "Boot ISA Selection"; FECCCON "Dynamic Flash ECC Configuration"; FSLEEP "Flash Sleep Mode"; DBGPER "Debug Mode CPU Access Permission"; EJTAGBEN "EJTAG Boot"; TSEQ "xxx"; CSEQ "xxx"; RWDTPS "Run Mode Watchdog Timer Post Scaler select bits"; RCLKSEL "Watchdog Timer Clock Select bits"; SWDTPS "Sleep Mode Watchdog Timer Post Scaler select bits"; DMTIVTL "xxx"; DMTIVTH "xxx"; DMTCNTL "xxx"; DMTCNTH "xxx"; DMTDIS "Dead Man Timer Disable bit"; SMBEN "SM Bus Enable"; SPI2PIN "SPI2 Pin Select bit"; CTXT3 "Specifies Interrupt Priority Level (IPL) Associated to Alternate Working Register 3 bits"; CTXT4 "Specifies Interrupt Priority Level (IPL) Associated to Alternate Working Register 4 bits"; MBXM0 "Mailbox 0 data direction"; MBXM1 "Mailbox 1 data direction"; MBXM2 "Mailbox 2 data direction"; MBXM3 "Mailbox 3 data direction"; MBXM4 "Mailbox 4 data direction"; MBXM5 "Mailbox 5 data direction"; MBXM6 "Mailbox 6 data direction"; MBXM7 "Mailbox 7 data direction"; MBXM8 "Mailbox 8 data direction"; MBXM9 "Mailbox 9 data direction"; MBXM10 "Mailbox 10 data direction"; MBXM11 "Mailbox 11 data direction"; MBXM12 "Mailbox 12 data direction"; MBXM13 "Mailbox 13 data direction"; MBXM14 "Mailbox 14 data direction"; MBXM15 "Mailbox 15 data direction"; MBXHSA "Mailbox Protocol A assigned to mailbox x"; MBXHSB "Mailbox Protocol B assigned to mailbox x"; MBXHSC "Mailbox Protocol C assigned to mailbox x"; MBXHSD "Mailbox Protocol D assigned to mailbox x"; MBXHSE "Mailbox Protocol E assigned to mailbox x"; MBXHSF "Mailbox Protocol F assigned to mailbox x"; MBXHSG "Mailbox Protocol G assigned to mailbox x"; MBXHSH "Mailbox Protocol H assigned to mailbox x"; HSAEN "Mailbox A data flow control protocol block enable"; HSBEN "Mailbox B data flow control protocol block enable"; HSCEN "Mailbox C data flow control protocol block enable"; HSDEN "Mailbox D data flow control protocol block enable"; HSEEN "Mailbox E data flow control protocol block enable"; HSFEN "Mailbox F data flow control protocol block enable"; HSGEN "Mailbox G data flow control protocol block enable"; HSHEN "Mailbox H data flow control protocol block enable"; CPRA0 "Pin RA0 Ownership Bits"; CPRA1 "Pin RA1 Ownership Bits"; CPRA2 "Pin RA2 Ownership Bits"; CPRA3 "Pin RA3 Ownership Bits"; CPRA4 "Pin RA4 Ownership Bits"; CPRB0 "Pin RB0 Ownership Bits"; CPRB1 "Pin RB1 Ownership Bits"; CPRB2 "Pin RB2 Ownership Bits"; CPRB3 "Pin RB3 Ownership Bits"; CPRB4 "Pin RB4 Ownership Bits"; CPRB5 "Pin RB5 Ownership Bits"; CPRB6 "Pin RB6 Ownership Bits"; CPRB7 "Pin RB7 Ownership Bits"; CPRB8 "Pin RB8 Ownership Bits"; CPRB9 "Pin RB9 Ownership Bits"; CPRB10 "Pin RB10 Ownership Bits"; CPRB11 "Pin RB11 Ownership Bits"; CPRB12 "Pin RB12 Ownership Bits"; CPRB13 "Pin RB13 Ownership Bits"; CPRB14 "Pin RB14 Ownership Bits"; CPRB15 "Pin RB15 Ownership Bits"; CPRC0 "Pin RC0 Ownership Bits"; CPRC1 "Pin RC1 Ownership Bits"; CPRC2 "Pin RC2 Ownership Bits"; CPRC3 "Pin RC3 Ownership Bits"; CPRC4 "Pin RC4 Ownership Bits"; CPRC5 "Pin RC5 Ownership Bits"; CPRC6 "Pin RC6 Ownership Bits"; CPRC7 "Pin RC7 Ownership Bits"; CPRC8 "Pin RC8 Ownership Bits"; CPRC9 "Pin RC9 Ownership Bits"; CPRC10 "Pin RC10 Ownership Bits"; CPRC11 "Pin RC11 Ownership Bits"; CPRC12 "Pin RC12 Ownership Bits"; CPRC13 "Pin RC13 Ownership Bits"; CPRC14 "Pin RC14 Ownership Bits"; CPRC15 "Pin RC15 Ownership Bits"; CPRD0 "Pin RD0 Ownership Bits"; CPRD1 "Pin RD1 Ownership Bits"; CPRD2 "Pin RD2 Ownership Bits"; CPRD3 "Pin RD3 Ownership Bits"; CPRD4 "Pin RD4 Ownership Bits"; CPRD5 "Pin RD5 Ownership Bits"; CPRD6 "Pin RD6 Ownership Bits"; CPRD7 "Pin RD7 Ownership Bits"; CPRD8 "Pin RD8 Ownership Bits"; CPRD9 "Pin RD9 Ownership Bits"; CPRD10 "Pin RD10 Ownership Bits"; CPRD11 "Pin RD11 Ownership Bits"; CPRD12 "Pin RD12 Ownership Bits"; CPRD13 "Pin RD13 Ownership Bits"; CPRD14 "Pin RD14 Ownership Bits"; CPRD15 "Pin RD15 Ownership Bits"; CPRE0 "Pin RE0 Ownership Bits"; CPRE1 "Pin RE1 Ownership Bits"; CPRE2 "Pin RE2 Ownership Bits"; CPRE3 "Pin RE3 Ownership Bits"; CPRE4 "Pin RE4 Ownership Bits"; CPRE5 "Pin RE5 Ownership Bits"; CPRE6 "Pin RE6 Ownership Bits"; CPRE7 "Pin RE7 Ownership Bits"; CPRE8 "Pin RE8 Ownership Bits"; CPRE9 "Pin RE9 Ownership Bits"; CPRE10 "Pin RE10 Ownership Bits"; CPRE11 "Pin RE11 Ownership Bits"; CPRE12 "Pin RE12 Ownership Bits"; CPRE13 "Pin RE13 Ownership Bits"; CPRE14 "Pin RE14 Ownership Bits"; CPRE15 "Pin RE15 Ownership Bits"; S1FNOSC "Oscillator Source Selection"; S1IESO "Two-speed Oscillator Start-Up"; S1OSCIOFNC "Slave OSC2 Pin Function bit"; S1FCKSM "Clock Switching and Monitor"; S1RWDTPS "Run Mode Watchdog Timer Post Scaler select bits"; S1RCLKSEL "Watchdog Timer Clock Select bits"; S1WINDIS "Watchdog Timer Window"; S1WDTWIN "Watchdog Timer Window Select bits"; S1SWDTPS "Sleep Mode Watchdog Timer Post Scaler select bits"; S1FWDTEN "Watchdog Timer Enable"; S1ICS "Slave ICD Communication Channel"; S1DEBUG "Background Debugger Enable"; S1ISOLAT "Isolate the Slave core subsystem from the master subsystem during Debug"; S1NOBTSWP "BOOTSWP Instruction Enable/Disable bit"; S1ALTI2C1 "Alternate I2C1 Pin bit"; S1SPI1PIN "S1 SPI1 Pin Select bit"; S1SSRE "Slave Slave Reset Enable"; S1MSRE "Master Slave Reset Enable"; S1CTXT1 "Specifies Interrupt Priority Level (IPL) Associated to Alternate Working Register 1 bits"; S1CTXT2 "Specifies Interrupt Priority Level (IPL) Associated to Alternate Working Register 2 bits"; S1CTXT3 "Specifies Interrupt Priority Level (IPL) Associated to Alternate Working Register 3 bits"; S1CTXT4 "Specifies Interrupt Priority Level (IPL) Associated to Alternate Working Register 4 bits"; BORLVL "xxx"; BSSO "xxx"; MCA "xxx"; MAXTEMP "xxx"; CFGAN14 "xxx"; CFGAN15 "xxx"; S1IOL1WAY "xxx"; S1BSSO "xxx"; S1BACKBUG "xxx"; BISTDIS "Memory BIST Feature Disable"; NOBTSWP "BOOTSWP instruction disable bit"; S1BISTDIS "Slave BIST on reset disable bit"; S1DMTIVTL "xxx"; S1DMTIVTH "xxx"; S1DMTCNTL "xxx"; S1DMTCNTH "xxx"; S1DMTDIS "Slave Dead Man Timer Disable bit"; BSEQ "xxx"; IBSEQ "xxx"; SMB3EN "SM Bus Enable"; FUSBIDIO2 "USB2 USBID Selection"; FVBUSIO2 "USB2 VBUSON Selection bit"; FUSBIDIO1 "USB1 USBID Selection"; FVBUSIO1 "USB2 VBUSON Selection bit"; VBATBOREN "VBAT BOR Enable"; FDSEN "Deep Sleep Enable"; BORSEL "Brown-out trip voltage"; POSCFGAIN "Primary Oscillator Fine Gain Control bits"; POSCAGCDLY "AGC Gain Search Step Settling Time Control"; POSCAGCRNG "AGC Lock Range bit"; POSCAGC "Primary Oscillator Gain Control bit"; FDBGWP "xxx"
      mask init:
      | MCHP_Master_Callback(gcbh,'INITIALISATION')
      settings: PreSaveFcn=MCHP_Fun.PreSaveFcn_DynamicOptions(gcbh);  OpenFcn=MCHP_Master_Callback(gcbh,'OPEN');
      mask TypeOptions PICREF: 30F2010 | 30F2011 | 30F2012 | 30F3010 | 30F3011 | 30F3012 | 30F3013 | 30F3014 | 30F4011 | 30F4012 | 30F4013 | 30F5011 | 30F5013 | 30F5015 | 30F5016 | 30F6010 | 30F6011 | 30F6012 | 30F6013 | 30F6014 | 30F6015 | 33CH128MP202 | 33CH128MP202S1 | 33CH128MP203 | 33CH128MP203S1 | 33CH128MP205 | 33CH128MP205S1 | 33CH128MP206 | 33CH128MP206S1 | 33CH128MP208 | 33CH128MP208S1 | 33CH128MP502 | 33CH128MP502S1 | 33CH128MP503 | 33CH128MP503S1 | 33CH128MP505 | 33CH128MP505S1 | 33CH128MP506 | 33CH128MP506S1 | 33CH128MP508 | 33CH128MP508S1 | 33CH256MP205 | 33CH256MP205S1 | 33CH256MP206 | 33CH256MP206S1 | 33CH256MP208 | 33CH256MP208S1 | 33CH256MP505 | 33CH256MP505S1 | 33CH256MP506 | 33CH256MP506S1 | 33CH256MP508 | 33CH256MP508S1 | 33CH512MP205 | 33CH512MP205S1 | 33CH512MP206 | 33CH512MP206S1 | 33CH512MP208 | 33CH512MP208S1 | 33CH512MP505 | 33CH512MP505S1 | 33CH512MP506 | 33CH512MP506S1 | 33CH512MP508 | 33CH512MP508S1 | 33CH64MP202 | 33CH64MP202S1 | 33CH64MP203 | 33CH64MP203S1 | 33CH64MP205 | 33CH64MP205S1 | 33CH64MP206 | 33CH64MP206S1 | 33CH64MP208 | 33CH64MP208S1 | 33CH64MP502 | 33CH64MP502S1 | 33CH64MP503 | 33CH64MP503S1 | 33CH64MP505 | 33CH64MP505S1 | 33CH64MP506 | 33CH64MP506S1 | 33CH64MP508 | 33CH64MP508S1 | 33CK128MP202 | 33CK128MP203 | 33CK128MP205 | 33CK128MP206 | 33CK128MP208 | 33CK128MP502 | 33CK128MP503 | 33CK128MP505 | 33CK128MP506 | 33CK128MP508 | 33CK256MP202 | 33CK256MP203 | 33CK256MP205 | 33CK256MP206 | 33CK256MP208 | 33CK256MP502 | 33CK256MP503 | 33CK256MP505 | 33CK256MP506 | 33CK256MP508 | 33CK32MP102 | 33CK32MP103 | 33CK32MP105 | 33CK32MP202 | 33CK32MP203 | 33CK32MP205 | 33CK32MP206 | 33CK32MP502 | 33CK32MP503 | 33CK32MP505 | 33CK32MP506 | 33CK64MP102 | 33CK64MP103 | 33CK64MP105 | 33CK64MP202 | 33CK64MP203 | 33CK64MP205 | 33CK64MP206 | 33CK64MP208 | 33CK64MP502 | 33CK64MP503 | 33CK64MP505 | 33CK64MP506 | 33CK64MP508 | 33EP128GM304 | 33EP128GM306 | 33EP128GM310 | 33EP128GM604 | 33EP128GM706 | 33EP128GM710 | 33EP128GP502 | 33EP128GP504 | 33EP128GP506 | 33EP128GS702 | 33EP128GS704 | 33EP128GS705 | 33EP128GS706 | 33EP128GS708 | 33EP128GS804 | 33EP128GS805 | 33EP128GS806 | 33EP128GS808 | 33EP128MC202 | 33EP128MC204 | 33EP128MC206 | 33EP128MC502 | 33EP128MC504 | 33EP128MC506 | 33EP16GS202 | 33EP16GS502 | 33EP16GS504 | 33EP16GS505 | 33EP16GS506 | 33EP256GM304 | 33EP256GM306 | 33EP256GM310 | 33EP256GM604 | 33EP256GM706 | 33EP256GM710 | 33EP256GP502 | 33EP256GP504 | 33EP256GP506 | 33EP256MC202 | 33EP256MC204 | 33EP256MC206 | 33EP256MC502 | 33EP256MC504 | 33EP256MC506 | 33EP256MU806 | 33EP256MU810 | 33EP256MU814 | 33EP32GP502 | 33EP32GP503 | 33EP32GP504 | 33EP32GS202 | 33EP32GS502 | 33EP32GS504 | 33EP32GS505 | 33EP32GS506 | 33EP32MC202 | 33EP32MC203 | 33EP32MC204 | 33EP32MC502 | 33EP32MC503 | 33EP32MC504 | 33EP512GM304 | 33EP512GM306 | 33EP512GM310 | 33EP512GM604 | 33EP512GM706 | 33EP512GM710 | 33EP512GP502 | 33EP512GP504 | 33EP512GP506 | 33EP512GP806 | 33EP512MC202 | 33EP512MC204 | 33EP512MC206 | 33EP512MC502 | 33EP512MC504 | 33EP512MC506 | 33EP512MC806 | 33EP512MU810 | 33EP512MU814 | 33EP64GP502 | 33EP64GP503 | 33EP64GP504 | 33EP64GP506 | 33EP64GS502 | 33EP64GS504 | 33EP64GS505 | 33EP64GS506 | 33EP64GS708 | 33EP64GS804 | 33EP64GS805 | 33EP64GS806 | 33EP64GS808 | 33EP64MC202 | 33EP64MC203 | 33EP64MC204 | 33EP64MC206 | 33EP64MC502 | 33EP64MC503 | 33EP64MC504 | 33EP64MC506 | 33EV128GM002 | 33EV128GM003 | 33EV128GM004 | 33EV128GM006 | 33EV128GM102 | 33EV128GM103 | 33EV128GM104 | 33EV128GM106 | 33EV256GM002 | 33EV256GM003 | 33EV256GM004 | 33EV256GM006 | 33EV256GM102 | 33EV256GM103 | 33EV256GM104 | 33EV256GM106 | 33EV32GM002 | 33EV32GM003 | 33EV32GM004 | 33EV32GM006 | 33EV32GM102 | 33EV32GM103 | 33EV32GM104 | 33EV32GM106 | 33EV64GM002 | 33EV64GM003 | 33EV64GM004 | 33EV64GM006 | 33EV64GM102 | 33EV64GM103 | 33EV64GM104 | 33EV64GM106 | 33FJ128GP202 | 33FJ128GP204 | 33FJ128GP206 | 33FJ128GP206A | 33FJ128GP306 | 33FJ128GP306A | 33FJ128GP310 | 33FJ128GP310A | 33FJ128GP706 | 33FJ128GP706A | 33FJ128GP708 | 33FJ128GP708A | 33FJ128GP710 | 33FJ128GP710A | 33FJ128GP802 | 33FJ128GP804 | 33FJ128MC202 | 33FJ128MC204 | 33FJ128MC506 | 33FJ128MC506A | 33FJ128MC510 | 33FJ128MC510A | 33FJ128MC706 | 33FJ128MC706A | 33FJ128MC708 | 33FJ128MC708A | 33FJ128MC710 | 33FJ128MC710A | 33FJ128MC802 | 33FJ128MC804 | 33FJ12GP201 | 33FJ12GP202 | 33FJ12MC201 | 33FJ12MC202 | 33FJ16GP304 | 33FJ16MC304 | 33FJ256GP506 | 33FJ256GP506A | 33FJ256GP510 | 33FJ256GP510A | 33FJ256GP710 | 33FJ256GP710A | 33FJ256MC510 | 33FJ256MC510A | 33FJ256MC710 | 33FJ256MC710A | 33FJ32GP202 | 33FJ32GP204 | 33FJ32GP302 | 33FJ32GP304 | 33FJ32MC202 | 33FJ32MC204 | 33FJ32MC302 | 33FJ32MC304 | 33FJ64GP202 | 33FJ64GP204 | 33FJ64GP206 | 33FJ64GP206A | 33FJ64GP306 | 33FJ64GP306A | 33FJ64GP310 | 33FJ64GP310A | 33FJ64GP706 | 33FJ64GP706A | 33FJ64GP708 | 33FJ64GP708A | 33FJ64GP710 | 33FJ64GP710A | 33FJ64GP802 | 33FJ64GP804 | 33FJ64MC202 | 33FJ64MC204 | 33FJ64MC506 | 33FJ64MC506A | 33FJ64MC508 | 33FJ64MC508A | 33FJ64MC510 | 33FJ64MC510A | 33FJ64MC706 | 33FJ64MC706A | 33FJ64MC710 | 33FJ64MC710A | 33FJ64MC802 | 33FJ64MC804 | 32MK0256GPG048 | 32MK0256GPG064 | 32MK0256MCJ048 | 32MK0256MCJ064 | 32MK0512GPG048 | 32MK0512GPG064 | 32MK0512GPK064 | 32MK0512GPK100 | 32MK0512MCF064 | 32MK0512MCF100 | 32MK0512MCJ048 | 32MK0512MCJ064 | 32MK0512MCM064 | 32MK0512MCM100 | 32MK1024GPK064 | 32MK1024GPK100 | 32MK1024MCF064 | 32MK1024MCF100 | 32MK1024MCM064 | 32MK1024MCM100 | 32MZ1024EFG064 | 32MZ1024EFG100 | 32MZ1024EFG124 | 32MZ1024EFG144 | 32MZ1024EFH064 | 32MZ1024EFH100 | 32MZ1024EFH124 | 32MZ1024EFH144 | 32MZ1024EFM064 | 32MZ1024EFM100 | 32MZ1024EFM124 | 32MZ1024EFM144 | 32MZ2048EFG064 | 32MZ2048EFG100 | 32MZ2048EFG124 | 32MZ2048EFG144 | 32MZ2048EFH064 | 32MZ2048EFH100 | 32MZ2048EFH124 | 32MZ2048EFH144 | 32MZ2048EFM064 | 32MZ2048EFM100 | 32MZ2048EFM124 | 32MZ2048EFM144 | SAMD51G18A - QFN48 | SAMD51G19A - QFN48 | SAMD51J18A - QFN64 | SAMD51J19A - WLCSP64 | SAMD51J19A - QFN64 | SAMD51J20A - WLCSP64 | SAMD51J20A - QFN64 | SAMD51N19A - TQFP100 | SAMD51N20A - TQFP100 | SAMD51P19A - TFBGA120 | SAMD51P19A - TQFP128 | SAMD51P20A - TFBGA120 | SAMD51P20A - TQFP128 | SAMD51J19B - TQFP64 | SAMD51J20C - WLCSP64 | SAME51G18A - QFN48 | SAME51G19A - QFN48 | SAME51J18A - QFN64 | SAME51J19A - QFN64 | SAME51J20A - QFN64 | SAME51N19A - TQFP100 | SAME51N20A - TQFP100 | SAME53J18A - QFN64 | SAME53J19A - QFN64 | SAME53J20A - QFN64 | SAME53N19A - TQFP100 | SAME53N20A - TQFP100 | SAME54N19A - TQFP100 | SAME54N20A - TQFP100 | SAME54P19A - TFBGA120 | SAME54P19A - TQFP128 | SAME54P20A - TFBGA120 | SAME54P20A - TQFP128 | SAME70J19B - LQFP64 | SAME70J20B - LQFP64 | SAME70J21B - LQFP64 | SAME70N19B - TFBGA100 | SAME70N19B - LQFP100 | SAME70N20B - TFBGA100 | SAME70N20B - LQFP100 | SAME70N21B - TFBGA100 | SAME70N21B - LQFP100 | SAME70Q19B - LFBGA144 | SAME70Q19B - UFBGA144 | SAME70Q19B - LQFP144 | SAME70Q20B - LFBGA144 | SAME70Q20B - UFBGA144 | SAME70Q20B - LQFP144 | SAME70Q21B - LFBGA144 | SAME70Q21B - UFBGA144 | SAME70Q21B - LQFP144 | SAMS70J19B - LQFP64 | SAMS70J19B - QFN64 | SAMS70J20B - LQFP64 | SAMS70J20B - QFN64 | SAMS70J21B - LQFP64 | SAMS70J21B - QFN64 | SAMS70N19B - TFBGA100 | SAMS70N19B - VFBGA100 | SAMS70N19B - LQFP100 | SAMS70N20B - TFBGA100 | SAMS70N20B - VFBGA100 | SAMS70N20B - LQFP100 | SAMS70N21B - TFBGA100 | SAMS70N21B - VFBGA100 | SAMS70N21B - LQFP100 | SAMS70Q19B - LFBGA144 | SAMS70Q19B - UFBGA144 | SAMS70Q19B - LQFP144 | SAMS70Q20B - LFBGA144 | SAMS70Q20B - UFBGA144 | SAMS70Q20B - LQFP144 | SAMS70Q21B - LFBGA144 | SAMS70Q21B - UFBGA144 | SAMS70Q21B - LQFP144 | SAMV70J19B - LQFP64 | SAMV70J20B - LQFP64 | SAMV70N19B - TFBGA100 | SAMV70N19B - LQFP100 | SAMV70N20B - TFBGA100 | SAMV70N20B - LQFP100 | SAMV70Q19B - TFBGA144 | SAMV70Q19B - LQFP144 | SAMV70Q20B - TFBGA144 | SAMV70Q20B - LQFP144 | SAMV71J19B - LQFP64 | SAMV71J20B - LQFP64 | SAMV71J21B - LQFP64 | SAMV71N19B - TFBGA100 | SAMV71N19B - LQFP100 | SAMV71N20B - TFBGA100 | SAMV71N20B - LQFP100 | SAMV71N21B - TFBGA100 | SAMV71N21B - LQFP100 | SAMV71Q19B - TFBGA144 | SAMV71Q19B - LQFP144 | SAMV71Q20B - TFBGA144 | SAMV71Q20B - LQFP144 | SAMV71Q21B - TFBGA144 | SAMV71Q21B - LQFP144
      mask Callback PICREF: MCHP_Master_Callback(gcbh , 'PICREF' ); % do not use spd field as that cause a problem
      mask TypeOptions BUSYFLAG: Dynamic Options
      mask TypeOptions PWRTEN: Not used
      mask TypeOptions BOREN: Enabled | Disable | Undefined
      mask TypeOptions BODENV: 2.7V | 4.2V | 4.5V | 2.0V
      mask TypeOptions BORV: Not used
      mask TypeOptions FPWRT: 128ms | 64ms | 32ms | 16ms | 8ms | 4ms | 2ms | Off | Timer Disabled | Disable
      mask TypeOptions DSBOREN: Enable ZPBOR during Deep Sleep Mode | Disable ZPBOR during Deep Sleep Mode
      mask TypeOptions DSLPBOR: Not used
      mask TypeOptions MCLRE: Enabled | Disable
      mask TypeOptions SMCLR: MCLR pin generates a normal system Reset | MCLR pin generates an emulated POR Reset
      mask TypeOptions PMDL1WAY: Allow only one reconfiguration | Allow multiple reconfigurations
      mask TypeOptions RSTPRI: Device will obtain reset instruction from Primary flash | Device will obtain reset instruction from Aux flash
      mask TypeOptions TEMP: Not used
      mask TypeOptions SOSCSRC: Not used
      mask TypeOptions SOSCSEL: Not used
      mask TypeOptions IOL1WAY: Allow only one reconfiguration | Allow multiple reconfigurations | Allow Only One Re-configuration | Allow Multiple Re-configurations
      mask TypeOptions ALTVREF: Not used
      mask TypeOptions DISUVREG: Not used
      mask TypeOptions DSSWEN: Not used
      mask TypeOptions LPCFG: Not used
      mask TypeOptions RTCBAT: Not used
      mask TypeOptions VBTBOR: Not used
      mask TypeOptions WUTSEL: Not used
      mask TypeOptions FNOSC: Primary Oscillator (HS; EC) w/ PLL | Primary Oscillator (HS; EC) | Internal Fast RC (FRC) w/ PLL | Internal Fast RC (FRC) | Internal Fast RC (FRC) Oscillator with postscaler | Back up Fast RC (BFRC) Oscillator | Low-Power RC Oscillator (LPRC) | Primary Oscillator with PLL module (XT + PLL; HS + PLL; EC + PLL) | Primary Oscillator (XT; HS; EC) | Fast RC Oscillator with PLL module (FRCPLL)  | Fast RC Oscillator with divide-by-N with PLL module (FRCPLL)  | Fast RC Oscillator with divide-by-N with PLL module (FRCPLL) | Secondary Oscillator (SOSC) | Fast RC Oscillator with divide-by-16 | Internal Fast RC (FRC) Oscillator with divide-by-16 | Primary Oscillator (XT; HS; EC) with PLL | Internal Fast RC with PLL (FRCPLL) | Internal Fast RC (FRC) Oscillator with divide by 16 | Internal Fast RC (FRC) with divide by 16 | Low Power RC oscillator (LPRC) | Internal Fast RC (FRC) with PLL | Internal Fast RC (FRC) oscillator | Internal Fast RC (FRC) with divide by N | Internal Fast RC (FRC) divide by 16 | Primary Oscillator (XT; HS; EC) w/ PLL | Primary Oscillator (MS; HS; EC) w/ PLL | Primary Oscillator (MS; HS; EC) | Low Power RC Osc (LPRC) | Low Power Secondary Osc (SOSC) | USB PLL (UPLL) | Primary Osc (HS;EC) | System PLL | Fast RC Osc w/Div-by-N (FRCDIV)
      mask TypeOptions FPR: ECIO w/ PLL 16x | ECIO w/ PLL 8x | ECIO w/ PLL 4x | ECIO | EC | ERC | ERCIO | XT w/PLL 16x | XT w/PLL 8x | XT w/PLL 4x | XT | HS | XTL | FRC w/ PLL 8x | FRC w/ PLL 16x | FRC w/ PLL 4x
      mask TypeOptions FOSFPR: HS3 w/PLL 16x | HS3 w/PLL 8x | HS3 w/PLL 4x | HS2 w/PLL 16x | HS2 w/PLL 8x | HS2 w/PLL 4x | ECIO w/PLL 16x | ECIO w/PLL 8x | ECIO w/PLL 4x | FRC w/PLL 8x | XT w/PLL 16x | XT w/PLL 8x | XT w/PLL 4x | FRC w/PLL 16x | FRC w/PLL 4x | ECIO | EC | ERC | ERCIO | XT | HS | XTL | Internal Low-Power RC (No change to Primary Osc Mode bits) | Internal Fast RC (No change to Primary Osc Mode bits) | Low-Power 32KHz Osc (No change to Primary Osc Mode bits)
      mask TypeOptions FOS: Primary Oscillator | Internal Low-Power RC | Internal Fast RC | Low-Power 32KHz Osc <TMR1 Osc>
      mask TypeOptions FRANGE: High Range | Low Range
      mask TypeOptions OSCILLATOR_SELECT: Internal Low Power 32 768 Hz Osc | Internal 48MHz Oscillator | Crystal Oscillator at 32kHz on XIN32/XOUT32 | Crystal Oscillator in 8-48MHz on XIN/XOUT 0 | Crystal Oscillator in 8-48MHz on XIN/XOUT 1 | External Clock in 8-48Mhz on XIN 0 | External Clock in 8-48Mhz on XIN
      mask Callback OSCILLATOR_SELECT: MCHP_Fun.BlockUpdate(gcbh); % Make sure it is executed at least once! %if ~strcmp(get_param(gcbh , 'OSCILLATOR_SELECT') , get_param(gcbh , 'OSCILLATOR_SELECT_spd')) MCHP_Master_Callback(gcbh , 'OSCILLATOR_SELECT' );  end;
      mask Callback QUARTZ: if ~strcmp(get_param(gcbh , 'QUARTZ'),get_param(gcbh , 'QUARTZ_spd')) MCHP_Fun.BlockUpdate(gcbh);  end;
      mask TypeOptions POSCGAIN: Gain Level 3 (highest) | Gain Level 2 | Gain Level 1 | Gain Level 0 (Lowest) | 2x gain setting | 1.5x gain setting | 1x gain setting | 0.5x gain setting
      mask TypeOptions POSCBOOST: Boost the kick start of the oscillator | Normal start of the oscillator
      mask TypeOptions SOSCGAIN: Gain is G3 | Gain is G2 | Gain is G1 | Gain is G0 | 2x gain setting | 1.5x gain setting | 0.5x gain setting | 1x gain setting | Gain Level 3 (highest) | Gain Level 2 | Gain Level 1 | Gain Level 0 (Lowest)
      mask TypeOptions SOSCBOOST: Boost the kick start of the oscillator | Normal start of the oscillator
      mask Callback ACTIV_PLL: if ~strcmp(get_param(gcbh , 'ACTIV_PLL'),get_param(gcbh , 'ACTIV_PLL_spd')) MCHP_Fun.BlockUpdate(gcbh); end;
      mask Callback MIPS_DESIRED: if ~strcmp(get_param(gcbh , 'MIPS_DESIRED'),get_param(gcbh , 'MIPS_DESIRED_spd')) MCHP_Fun.BlockUpdate(gcbh);  end;
      mask TypeOptions FPLLMUL: Not used
      mask TypeOptions FPLLIDIV: 8x Divider | 7x Divider | 6x Divider | 5x Divider | 4x Divider | 3x Divider | 2x Divider | 1x Divider
      mask TypeOptions POSCFREQ: Not used
      mask TypeOptions POSCMD: Primary Oscillator Disabled | HS Oscillator Mode | EC Oscillator Mode | HS Crystal Oscillator Mode | XT Crystal Oscillator Mode | EC (External Clock) Mode | XT Oscillator Mode
      mask TypeOptions POSCMOD: Primary Oscillator Disabled | HS Oscillator mode selected | MS Oscillator mode selected | EC Oscillator mode selected | Primary osc disabled | HS osc mode | External clock mode
      mask TypeOptions ACLKCON: Optimized for PWM resolution & ADC conversion speed | Optimized for PWM precision | Optimized for Low Power Consumption | Use Principal Oscillator with PLL | Use Principal Oscillator without PLL | Use FRC with PLL | Use FRC without PLL
      mask Callback ACLKCON: if ~strcmp(get_param(gcbh , 'ACLKCON'),get_param(gcbh , 'ACLKCON_spd')) MCHP_Fun.BlockUpdate(gcbh);  end;
      mask TypeOptions FPLLODIV: 32x Divider | 16x Divider | 8x Divider | 4x Divider | 2x Divider
      mask TypeOptions PLLKEN: PLL lock signal will be used to disable PLL clock output if lock is lost | PLL lock signal is not used; the PLL clock output will not be disabled if lock is lost | PLL clock output will be disabled if LOCK is lost | PLL clock output will not be disabled if LOCK is lost | Clock switch to PLL source will wait until the PLL lock signal is valid. | Clock switch will not wait for the PLL lock signal. | Clock switch to PLL source will wait until the PLL lock signal is valid | Clock switch will not wait for the PLL lock signal
      mask TypeOptions FCKSM: Sw Disabled; Mon Disabled | Sw Enabled; Mon Disabled | Sw Enabled; Mon Enabled | Both Clock switching and Fail-safe Clock Monitor are disabled | Clock switching is enabled;Fail-safe Clock Monitor is disabled | Both Clock switching and Fail-safe Clock Monitor are enabled | Clock switching and Fail-Safe Clock Monitor are disabled; Mon Disabled | Clock switching is enabled; Fail-Safe Clock Monitor is Disabled | Clock switching and Fail-Safe Clock Monitor are enabled | Clock switching and Fail-Safe Clock Monitor are disabled | Clock switching is enabled; Fail-Safe Clock Monitor is enabled | Clock Switch Enabled; FSCM Enabled | Clock Switch Disabled; FSCM Enabled | Clock Switch Enabled; FSCM Disabled | Clock Switch Disabled; FSCM Disabled
      mask TypeOptions FCKSMEN: Sw Disabled; Mon Disabled | Sw Enabled; Mon Disabled | Sw Enabled; Mon Enabled
      mask TypeOptions IESO: Start up with FRC; then switch | Disable | Start up device with FRC;then automatically switch to user selected oscillator source | Start up device with user selected oscillator source | Enabled
      mask TypeOptions DSWDTPS: 1:2^36 | 1:2^35 | 1:2^34 | 1:2^33 | 1:2^32 | 1:2^31 | 1:2^30 | 1:2^29 | 1:2^28 | 1:2^27 | 1:2^26 | 1:2^25 | 1:2^24 | 1:2^23 | 1:2^22 | 1:2^21 | 1:2^20 | 1:2^19 | 1:2^18 | 1:2^17 | 1:2^16 | 1:2^15 | 1:2^14 | 1:2^13 | 1:2^12 | 1:2^11 | 1:2^10 | 1:2^9 | 1:2^8 | 1:2^7 | 1:2^6 | 1:2^5
      mask TypeOptions FWDTEN: Enable | Disable
      mask TypeOptions FWDTWINSZ: Window size is 25% | Window size is 37.5% | Window size is 50% | Window size is 75%
      mask TypeOptions FWPSA: 1:512 | 1:64 | 1:8 | 1:1
      mask TypeOptions FWPSA0: 1:128 | 1:32
      mask TypeOptions FWPSB: 1:16 | 1:15 | 1:14 | 1:13 | 1:12 | 1:11 | 1:10 | 1:9 | 1:8 | 1:7 | 1:6 | 1:5 | 1:4 | 1:3 | 1:2 | 1:1
      mask TypeOptions WDT: Enabled | Disable
      mask TypeOptions WDTPOST: 1:32768 | 1:16;384 | 1:8192 | 1:4096 | 1:2;048 | 1:1024 | 1:512 | 1:256 | 1:128 | 1:64 | 1:32 | 1:16 | 1:8 | 1:4 | 1:2 | 1:1
      mask TypeOptions WDTPRE: 1:128 | 1:32 | Prescaler ratio of 1:128 | Prescaler ratio of 1:32
      mask TypeOptions WDTPS: 1:32768 | 1:16;384 | 1:8192 | 1:4096 | 1:2;048 | 1:1024 | 1:512 | 1:256 | 1:128 | 1:64 | 1:32 | 1:16 | 1:8 | 1:4 | 1:2 | 1:1 | 1:1048576 | 1:524288 | 1:262144 | 1:131072 | 1:65536 | 1:16384 | 1:2048
      mask TypeOptions WINDIS: Watchdog Timer operates in Non-Window mode | Watchdog Timer operates in Window mode | Watchdog Timer in Non-Window mode | Watchdog Timer in Window mode | Watchdog Timer is in non-Window mode | Watchdog Timer is in Window mode
      mask TypeOptions WWDTEN: Non-Window mode | Window mode
      mask TypeOptions DSWDTEN: Enable DSWDT during Deep Sleep Mode | Disable DSWDT during Deep Sleep Mode
      mask TypeOptions DSWDTOSC: Select LPRC as DSWDT Reference clock | Select SOSC as DSWDT Reference Clock
      mask TypeOptions FPBDIV: Not used
      mask TypeOptions FSOSCEN: Enable Secondary Oscillator | Disable Secondary Oscillator
      mask TypeOptions LPRCSEL: Not used
      mask TypeOptions OSCIOFCN: Not used
      mask TypeOptions OSCIOFNC: OSCO pin has clock out function | general purpose digital I/O pin | OSC2 is clock output | Disable | Enabled
      mask TypeOptions LVRCFG: Not used
      mask TypeOptions PLL_96MHZ: Not used
      mask TypeOptions PLL96MHZ: Not used
      mask TypeOptions PLLDIV: Not used
      mask TypeOptions WDTCLK: Not used
      mask TypeOptions WDTCMX: Not used
      mask TypeOptions WDTWIN: WDT Window is 25% of WDT period | WDT Window is 37.5% of WDT period | WDT Window is 50% of WDT period | WDT Windo is 75% of WDT period | WDT Window is 75% of WDT period | Watchdog Window is 25% of WDT period | Watchdog Window is 37.5% of WDT period | Watchdog Window is 50% of WDT period | Watchdog Window is 75% of WDT period
      mask TypeOptions XTCFG: 24-32 MHz crystals | 16-24 MHz crystals | 8-16 MHz crystals | 4-8 MHz crystals
      mask TypeOptions XTBST: Boost the kick-start | Default kick-start
      mask TypeOptions APL: Aux Flash Code protect is disabled | Aux Flash Code protect is enabled
      mask TypeOptions APLK: Aux Flash Write Protection or Code Protection is Enabled | Aux Flash Write Protection and Code Protection is Disabled
      mask TypeOptions AWRP: Aux Flash may be written | Aux Flash is write protected | Auxiliary program memory is not write-protected | Auxiliary program memory is write-protected
      mask TypeOptions BSS: No Boot Segment | Standard Security; Small-sized Boot Flash | Standard Security; Medium-sized Boot Flash | High Security; Small-sized Boot Flash | High Security; Medium-sized Boot Flash | Standard Security; Large-sized Boot Flash | High Security; Large-sized Boot Flash | No Protection (other than BWRP) | Standard Security | High Security | No Boot Segment Program Memory | No Boot program Flash segment
      mask TypeOptions BWP: Not used
      mask TypeOptions BWRP: Boot Segment may be written | Boot Segment is write protected | Boot Segment Program Memory may be written | Boot Segment Program Memory is write protected | Boot segment is write-protected
      mask TypeOptions CP: Protection Disabled | Protection Enabled
      mask TypeOptions EBS: No Boot EEPROM | Boot EEPROM Enabled
      mask TypeOptions ESS: No Segment Data EEPROM | Small-sized Secure Data EEPROM | Medium-sized Secure Data EEPROM | Large-sized Secure Data EEPROM
      mask TypeOptions GCP: Disable | Enabled | High Security Code Protection Enabled | General Segment Code protect is Disabled | General Segment Code protection Enabled | Standard Security Code protection Enabled
      mask TypeOptions GSS: Disable | Enabled | High Security Code Protection Enabled | No Protection (other than GWRP) | Standard Security | High Security | General Segment Code protect is Disabled | Standard Security Code protection Enabled | User program memory is not code-protected | Standard Security Code Protection is Enabled
      mask TypeOptions GSS0: Not used
      mask TypeOptions GSSK: General Segment Write Protection or Code Protection is Enabled | General Segment Write Protection and Code Protection is Disabled
      mask TypeOptions GWRP: General Segment may be written | General Segment is write protected | Disable | Enabled | User program memory is write-protected | Writes to program memory are allowed | Writes to program memory are disabled
      mask TypeOptions PWP: Not used
      mask TypeOptions RBS: No Boot RAM | Small-sized Boot RAM | Medium-sized Boot RAM | Large-sized Boot RAM
      mask TypeOptions RSS: No Secure RAM | Small-sized Secure RAM | Medium-sized Secure RAM | Large-sized Secure RAM
      mask TypeOptions SSS: No Secure Segment | Standard Security; Small-sized Secure Flash | Standard Security; Medium-sized Secure Flash | Standard Security; Large-sized Secure Flash | High Security; Small-sized Secure Flash | High Security; Medium-sized Secure Flash | High Security; Large-sized Secure Flash
      mask TypeOptions SWRP: Disable | Enabled | Secure segment may be written | Secure segment is write protected
      mask TypeOptions WPCFG: Not used
      mask TypeOptions WPDIS: Not used
      mask TypeOptions WPEND: Not used
      mask TypeOptions WPFP: Not used
      mask TypeOptions ICESEL: Communicate on PGEC1/PGED1 | Communicate on PGEC2/PGED2 | Communicate on PGEC3/PGED3
      mask TypeOptions ICS: Use PGC/EMUC and PGD/EMUD | Use EMUC1 and EMUD1 | Use EMUC2 and EMUD2 | Use EMUC3 and EMUD3 | Communicate on PGC1 and PGD1 | Communicate on PGC2 and PGD2 | Communicate on PGC3 and PGD3 | Communicate on PGEC1 and PGED1 | Communicate on PGEC2 and PGED2 | Communicate on PGEC3 and PGED3 | Communicate on PGEC1/PGED1 | Communicate on PGEC2/PGED2 | Communicate on PGEC3/PGED3
      mask TypeOptions JTAGEN: Enable | Disable
      mask TypeOptions COE: Not used
      mask TypeOptions RES: Not used
      mask TypeOptions DEBUG: Debugger is disabled | Debugger is enabled
      mask TypeOptions BACKBUG: Not used
      mask TypeOptions BKBUG: Not used
      mask TypeOptions ALTI2C: I2C mapped to SDA1/SCL1 pins | I2C mapped to ASDA1/ASCL1 pins | I2C mapped to SDA1/SCL1 | I2C mapped to ASDA1/ASCL1
      mask TypeOptions ALTI2C1: I2C1 mapped to SDA1/SCL1 pins | I2C1 mapped to ASDA1/ASCL1 pins | SDA1/SCK1 pins are selected as the I/O pins for I2C1 | ASDA1/ASCK1 pins are selected as the I/O pins for I2C1
      mask TypeOptions ALTI2C2: I2C2 mapped to SDA2/SCL2 pins | I2C2 mapped to ASDA2/ASCL2 pins | SDA2/SCK2 pins are selected as the I/O pins for I2C2 | ASDA2/ASCK2 pins are selected as the I/O pins for I2C2
      mask TypeOptions ALTI2C3: I2C3 mapped to SDA3/SCL3 pins | I2C3 mapped to ASDA3/ASCL3 pins
      mask TypeOptions ALTQIO: QEA1; QEB1; INDX1 are selected as inputs to QEI1 | AQEA1; AQEB1; and AINDX1 are selected as inputs to QEI1
      mask TypeOptions ALTSS1: SS1A is selected as the I/O pin for SPI1 | SS1 is selected as the I/O pin for SPI1
      mask TypeOptions CMPPOL0: Hysteresis is applied to falling edge | Hysteresis is applied to rising edge
      mask TypeOptions CMPPOL1: Hysteresis is applied to falling edge | Hysteresis is applied to rising edge
      mask TypeOptions FCANIO: Not used
      mask TypeOptions FETHIO: Default Ethernet I/O | Alternate Ethernet I/O
      mask TypeOptions FMIIEN: MII Enabled | RMII Enabled
      mask TypeOptions FSRSSEL: Not used
      mask TypeOptions FUSBIDIO: Controlled by the USB Module | Controlled by Port Function
      mask TypeOptions FVBUSONIO: Not used
      mask TypeOptions HPOL: Active High | Active Low | PWM module high side output pins have active-high output polarity | PWM module high side output pins have active-low output polarity
      mask TypeOptions HYST0: 45 mV Hysteresis | 30 mV Hysteresis | 15 mV Hysteresis | No Hysteresis
      mask TypeOptions HYST1: 45 mV Hysteresis | 30 mV Hysteresis | 15 mV Hysteresis | No Hysteresis
      mask TypeOptions I2C1SEL: Not used
      mask TypeOptions LPOL: Active High | Active Low | PWM module low side output pins have active-high output polarity | PWM module low side output pins have active-low output polarity
      mask TypeOptions PWMPIN: Control with PORT/TRIS regs | Control with HPOL/LPOL bits | PWM module pins controlled by PORT register at device Reset | PWM module pins controlled by PWM module at device Reset
      mask TypeOptions RTCOSC: Not used
      mask TypeOptions UPLLEN: USB PLL Disabled | USB PLL Enabled
      mask TypeOptions UPLLIDIV: Not used
      mask TypeOptions ATMOD8: Not used
      mask TypeOptions ALTPMP: Not used
      mask TypeOptions I2C2SEL: Not used
      mask TypeOptions ALTADREF: Not used
      mask TypeOptions ALTCVREF: Not used
      mask TypeOptions PWMLOCK: Certain PWM registers may only be written after key sequence | PWM registers may be written without key sequence
      mask TypeOptions INT_PRIORITY_DMA: 0 | 1 | 2 | 3 | 4 | 5 | 6 | 7
      mask TypeOptions BTMODE: Not used
      mask TypeOptions RES1: Not used
      mask TypeOptions PLLSS: Not used
      mask TypeOptions RES2: Not used
      mask TypeOptions ALTCMPI: Not used
      mask TypeOptions BOREN1: Not used
      mask TypeOptions ALTRB6: Not used
      mask TypeOptions RETCFG: Not used
      mask TypeOptions DFMCY: Not used
      mask TypeOptions BSS2: No Boot Segment | Boot Segment size determined by FBSLIM
      mask TypeOptions BSEN: No Boot Segment | Boot Segment size determined by FBSLIM
      mask TypeOptions CWRP: Configuration Segment may be written | Configuration Segment is write protected
      mask TypeOptions CSS: No Protection (other than CWRP) | Standard Security | Enhanced Security | High Security
      mask TypeOptions AIVTDIS: Disabled AIVT | Enabled AIVT | Disable Alternate Vector Table | Enable Alternate Vector Table
      mask TypeOptions BSLIM: Not used
      mask TypeOptions WDTEN: Enable | Disable
      mask TypeOptions BTSWP: BOOTSWP instruction is disabled | BOOTSWP instruction is enabled
      mask TypeOptions DBCC: No Cross Connection between DAC outputs | Interconnects DACOUT1 and DACOUT2
      mask TypeOptions CTXT1: Not Assigned | Alternate Register set assigned to IPL level 7 | Alternate Register set assigned to IPL level 6 | Alternate Register set assigned to IPL level 5 | Alternate Register set assigned to IPL level 4 | Alternate Register set assigned to IPL level 3 | Alternate Register set assigned to IPL level 2 | Alternate Register set assigned to IPL level 1 | Alternate register set 1 assigned to IPL level 7 | Alternate register set 1 assigned to IPL level 6 | Alternate register set 1 assigned to IPL level 5 | Alternate register set 1 assigned to IPL level 4 | Alternate register set 1 assigned to IPL level 3 | Alternate register set 1 assigned to IPL level 2 | Alternate register set 1 assigned to IPL level 1
      mask TypeOptions CTXT2: Not Assigned | Alternate Register set assigned to IPL level 7 | Alternate Register set assigned to IPL level 6 | Alternate Register set assigned to IPL level 5 | Alternate Register set assigned to IPL level 4 | Alternate Register set assigned to IPL level 3 | Alternate Register set assigned to IPL level 2 | Alternate Register set assigned to IPL level 1 | Alternate register set 2 assigned to IPL level 7 | Alternate register set 2  assigned to IPL level 6 | Alternate register set 2  assigned to IPL level 5 | Alternate register set 2  assigned to IPL level 4 | Alternate register set 2  assigned to IPL level 3 | Alternate register set 2  assigned to IPL level 2 | Alternate register set 2  assigned to IPL level 1
      mask TypeOptions SEQNUM: Not used
      mask TypeOptions nSEQNUM: Not used
      mask TypeOptions BOREN0: Enabled | Disable
      mask TypeOptions DMTIVT: Not used
      mask TypeOptions DMTCNT: 2^31 (2147483648) | 2^30 (1073741824) | 2^29 (536870912) | 2^28 (268435456) | 2^27 (134217728) | 2^26 (67108864) | 2^25 (33554432) | 2^24 (16777216) | 2^23 (8388608) | 2^22 (4194304) | 2^21 (2097152) | 2^20 (1048576) | 2^19 (524288) | 2^18 (262144) | 2^17 (131072) | 2^16 (65536) | 2^15 (32768) | 2^14 (16384) | 2^13 (8192) | 2^12 (4096) | 2^11 (2048) | 2^10 (1024) | 2^9 (512) | 2^8 (256)
      mask TypeOptions DMTEN: Dead Man Timer is Enabled and cannot be disabled by software | Dead Man Timer is Disabled and can be enabled by software
      mask TypeOptions ON: Not used
      mask TypeOptions USERID: Not used
      mask TypeOptions RESERVED1: Not used
      mask TypeOptions PGL1WAY: Allow only one reconfiguration | Allow multiple reconfigurations
      mask TypeOptions FPLLRNG: 54-64 MHz Input | 34-64 MHz Input | 21-42 MHz Input | 13-26 MHz Input | 8-16 MHz Input | 5-10 MHz Input | Bypass | 34-68 MHz Input
      mask TypeOptions FPLLICLK: FRC is input to the System PLL | POSC is input to the System PLL
